simulink library "Centralized_I_Lib_Controller"  (R2024b)
settings: Solver=VariableStepAuto  StartTime=0.0  StopTime=10.0  RelTol=1e-3
(part 2 of 7)

== matlab function Centralized_I_Lib_Controller/computedTorqueControl_sym ==
  data: ddqd input; dqd input; qd input; kd input; kp input; tau output; dq input; q input
function tau = computedTorqueControl_sym(ddqd,dqd,qd,kd,kp,dq,q)
%#codegen

% Manually assign inputs from vectors to scalars
q1 = q(1);  q2 = q(2);  q3 = q(3);
q4 = q(4);  q5 = q(5);  q6 = q(6);

dq1 = dq(1);  dq2 = dq(2);  dq3 = dq(3);
dq4 = dq(4);  dq5 = dq(5);  dq6 = dq(6);

qd1 = qd(1);  qd2 = qd(2);  qd3 = qd(3);
qd4 = qd(4);  qd5 = qd(5);  qd6 = qd(6);

dqd1 = dqd(1);  dqd2 = dqd(2);  dqd3 = dqd(3);
dqd4 = dqd(4);  dqd5 = dqd(5);  dqd6 = dqd(6);

ddqd1 = ddqd(1);  ddqd2 = ddqd(2);  ddqd3 = ddqd(3);
ddqd4 = ddqd(4);  ddqd5 = ddqd(5);  ddqd6 = ddqd(6);

kp1 = kp(1); kp2 = kp(2); kp3 = kp(3);
kp4 = kp(4); kp5 = kp(5); kp6 = kp(6);

kd1 = kd(1); kd2 = kd(2); kd3 = kd(3);
kd4 = kd(4); kd5 = kd(5); kd6 = kd(6);

% Kp = diag(kp);
% Kd = diag(kd);

%    This function was generated by the Symbolic Math Toolbox version 24.2.
%    13-Jun-2025 15:28:52

% ddqd1 = complex(ddqd1);  % if required to enforce complex operations
% ddqd2 = complex(ddqd2);  % if required to enforce complex operations
% ddqd3 = complex(ddqd3);  % if required to enforce complex operations
% ddqd4 = complex(ddqd4);  % if required to enforce complex operations
% ddqd5 = complex(ddqd5);  % if required to enforce complex operations
% ddqd6 = complex(ddqd6);  % if required to enforce complex operations
% dq1 = complex(dq1);  % if required to enforce complex operations
% dq2 = complex(dq2);  % if required to enforce complex operations
% dq3 = complex(dq3);  % if required to enforce complex operations
% dq4 = complex(dq4);  % if required to enforce complex operations
% dq5 = complex(dq5);  % if required to enforce complex operations
% dq6 = complex(dq6);  % if required to enforce complex operations
% dqd1 = complex(dqd1);  % if required to enforce complex operations
% dqd2 = complex(dqd2);  % if required to enforce complex operations
% dqd3 = complex(dqd3);  % if required to enforce complex operations
% dqd4 = complex(dqd4);  % if required to enforce complex operations
% dqd5 = complex(dqd5);  % if required to enforce complex operations
% dqd6 = complex(dqd6);  % if required to enforce complex operations
% kd1 = complex(kd1);  % if required to enforce complex operations
% kd2 = complex(kd2);  % if required to enforce complex operations
% kd3 = complex(kd3);  % if required to enforce complex operations
% kd4 = complex(kd4);  % if required to enforce complex operations
% kd5 = complex(kd5);  % if required to enforce complex operations
% kd6 = complex(kd6);  % if required to enforce complex operations
% kp1 = complex(kp1);  % if required to enforce complex operations
% kp2 = complex(kp2);  % if required to enforce complex operations
% kp3 = complex(kp3);  % if required to enforce complex operations
% kp4 = complex(kp4);  % if required to enforce complex operations
% kp5 = complex(kp5);  % if required to enforce complex operations
% kp6 = complex(kp6);  % if required to enforce complex operations
% q1 = complex(q1);  % if required to enforce complex operations
% q2 = complex(q2);  % if required to enforce complex operations
% q3 = complex(q3);  % if required to enforce complex operations
% q4 = complex(q4);  % if required to enforce complex operations
% q5 = complex(q5);  % if required to enforce complex operations
% q6 = complex(q6);  % if required to enforce complex operations
% qd1 = complex(qd1);  % if required to enforce complex operations
% qd2 = complex(qd2);  % if required to enforce complex operations
% qd3 = complex(qd3);  % if required to enforce complex operations
% qd4 = complex(qd4);  % if required to enforce complex operations
% qd5 = complex(qd5);  % if required to enforce complex operations
% qd6 = complex(qd6);  % if required to enforce complex operations
t2 = cos(q1);
t3 = cos(q2);
t4 = cos(q3);
t5 = cos(q4);
t6 = cos(q5);
t7 = cos(q6);
t8 = sin(q1);
t9 = sin(q2);
t10 = sin(q3);
t11 = sin(q4);
t12 = sin(q5);
t13 = sin(q6);
t14 = q4.*2.0;
t15 = q5.*2.0;
t30 = -ddqd1;
t31 = -ddqd2;
t32 = -ddqd3;
t33 = -ddqd4;
t34 = -ddqd5;
t35 = -ddqd6;
t36 = -dqd1;
t37 = -dqd2;
t38 = -dqd3;
t39 = -dqd4;
t40 = -dqd5;
t41 = -dqd6;
t42 = -qd1;
t43 = -qd2;
t44 = -qd3;
t45 = -qd4;
t46 = -qd5;
t47 = -qd6;
t63 = sqrt(2.0);
t64 = pi./2.0;
t16 = cos(t14);
t17 = cos(t15);
t18 = t3.^2;
t19 = t4.^2;
t20 = t5.^2;
t21 = t6.^2;
t22 = t7.^2;
t23 = sin(t14);
t24 = sin(t15);
t25 = t9.^2;
t26 = t10.^2;
t27 = t11.^2;
t28 = t12.^2;
t29 = t13.^2;
t48 = t2.*t4;
t49 = t3.*t5;
t50 = t4.*t5;
t51 = t4.*t6;
t52 = t2.*t10;
t53 = t4.*t8;
t54 = t3.*t11;
t55 = t5.*t9;
t56 = t4.*t11;
t57 = t4.*t12;
t58 = t6.*t10;
t59 = t8.*t10;
t60 = t9.*t11;
t61 = t10.*t11;
t62 = t10.*t12;
t67 = t5.*t10.*4.0;
t68 = dq1+t36;
t69 = dq2+t37;
t70 = dq3+t38;
t71 = dq4+t39;
t72 = dq5+t40;
t73 = dq6+t41;
t74 = q1+t42;
t75 = q2+t43;
t76 = q3+t44;
t77 = q4+t45;
t78 = q5+t46;
t79 = q6+t47;
t80 = -t64;
t90 = t3.*(3.0./1.0e+1);
t91 = t6.*(3.0./4.0e+1);
t92 = t6.*(3.0./5.0e+1);
t93 = t9.*(3.0./1.0e+1);
t94 = t63+2.0;
t139 = t3.*(9.0./1.0e+1);
t141 = t6.*(3.0./2.0e+2);
t142 = t9.*(9.0./1.0e+1);
t143 = t12.*(3.0./1.0e+2);
t157 = -t63;
t158 = t63.*4.7e+1;
t175 = t5.*t12.*(3.0./4.0e+1);
t182 = t11.*t12.*(3.0./4.0e+1);
t184 = t4.*(3.9e+1./2.0e+2);
t185 = t5.*(9.0./4.0e+2);
t187 = t11.*(2.7e+1./1.0e+2);
t188 = t10.*(9.0./2.0e+2);
t229 = t3.*t6.*(3.0./1.0e+2);
t246 = t6.*t11.*(-3.0./4.0e+1);
t248 = t5.*t10.*(9.0./5.0e+1);
t249 = t3.*t12.*(3.0./2.0e+2);
t253 = t5.*t12.*(3.0./2.0e+2);
t257 = t5.*t10.*(3.0./4.0e+2);
t263 = t11.*t12.*(3.0./2.0e+2);
t266 = t5.*(1.17e+2./2.0e+2);
t309 = t5.*t6.*(-3.0./2.0e+2);
t310 = t3.*t4.*(9.0./2.0e+2);
t312 = t5.*t6.*(9.0./2.0e+2);
t331 = t5.*t12.*(9.0./1.0e+2);
t332 = t6.*t11.*(9.0./1.0e+2);
t335 = t6.*t9.*(-3.0./2.0e+2);
t338 = t6.*t11.*(-3.0./2.0e+2);
t340 = t4.*t9.*(9.0./2.0e+2);
t343 = t3.*t10.*(3.9e+1./2.0e+2);
t347 = t9.*t12.*(-3.0./1.0e+2);
t351 = t11.*t12.*(9.0./2.0e+2);
t352 = t9.*t10.*(3.9e+1./2.0e+2);
t436 = t5.*t6.*t11.*(6.0./2.5e+1);
t494 = t5.*t11.*t12.*(3.0./2.5e+1);
t519 = t6.*5.9765625e-3;
t520 = t2.*1.0675e-2;
t521 = t8.*1.0675e-2;
t522 = t12.*2.98828125e-3;
t595 = t3.*t6.*t9.*(-3.0./5.0e+1);
t663 = t4.*2.444921875e-1;
t664 = t5.*1.048828125e-2;
t667 = t11.*2.09765625e-2;
t933 = t5.*t11.*t12.*(-3.0./1.0e+2);
t955 = t5.*t6.*2.98828125e-3;
t957 = t7.*t13.*5.5078125e-3;
t959 = t5.*t12.*5.9765625e-3;
t1077 = t5.*t6.*t11.*t12.*(-3.0./5.0e+1);
t1132 = t5.*t6.*t11.*(-9.0./2.0e+2);
t1137 = t5.*t6.*t12.*2.05078125e-2;
t1191 = t11.*t12.*(-2.98828125e-3);
t1323 = t63.*2.75390625e-3;
t1418 = t5.*t11.*6.88175e-1;
t1598 = t2.*t6.*t12.*1.865e-2;
t1599 = t3.*t4.*t10.*9.325e-3;
t1618 = t6.*t8.*t12.*1.865e-2;
t1625 = t4.*t9.*t10.*9.325e-3;
t1702 = t4.*5.198296875e-1;
t1803 = t7.*t9.*t13.*(-5.5078125e-3);
t1804 = t7.*t10.*t13.*(-5.5078125e-3);
t1805 = t7.*t11.*t13.*(-5.5078125e-3);
t1806 = t7.*t12.*t13.*(-5.5078125e-3);
t1831 = t3.*t4.*1.039659375;
t1845 = t3.*t9.*1.4703625;
t1846 = t6.*t12.*2.98328125e-2;
t1917 = t3.*t63.*1.376953125e-3;
t1918 = t5.*t63.*1.376953125e-3;
t1925 = t9.*t63.*(-2.75390625e-3);
t1926 = t11.*t63.*(-2.75390625e-3);
t1927 = t12.*t63.*1.376953125e-3;
t2024 = t3.*t10.*5.198296875e-1;
t2061 = t3.*t9.*t63.*5.5078125e-3;
t2062 = t5.*t11.*t63.*5.5078125e-3;
t2091 = t3.*t4.*t7.*t13.*(-5.5078125e-3);
t2213 = t6.*t7.*t63.*(-2.75390625e-3);
t2222 = t7.*t13.*t63.*(-2.75390625e-3);
t2250 = t5.*t6.*t7.*t11.*t13.*1.1015625e-2;
t2362 = t6.*t7.*t12.*t63.*5.5078125e-3;
t2423 = t5.*t10.*t63.*(-1.376953125e-3);
t2425 = t11.*t12.*t63.*(-1.376953125e-3);
t2571 = t5.*t6.*t13.*t63.*(-2.75390625e-3);
t3047 = t5.*t6.*t7.*t12.*t63.*(-5.5078125e-3);
t3690 = t3.*t6.*t7.*t9.*t12.*t63.*(-5.5078125e-3);
t6734 = t3.*1.181403645833333e-1;
t6735 = t9.*2.362807291666667e-1;
t6736 = t4.*t10.*1.180036458333333e-1;
t6754 = t3.*t4.*t10.*(-1.180036458333333e-1);
t65 = t50.*4.0;
t66 = t56.*4.0;
t82 = t9.*t59;
t83 = t8.*t60;
t84 = t11.*t59;
t85 = t10.*t60;
t86 = t12.*t60;
t87 = t12.*t61;
t88 = -t58;
t89 = -t61;
t95 = t2.*t49;
t96 = t5.*t48;
t97 = t3.*t51;
t98 = t6.*t49;
t99 = t6.*t50;
t100 = t9.*t48;
t101 = t2.*t54;
t102 = t2.*t55;
t103 = t8.*t49;
t104 = t11.*t48;
t105 = t5.*t52;
t106 = t8.*t50;
t107 = t10.*t49;
t108 = t3.*t57;
t109 = t3.*t58;
t110 = t9.*t51;
t111 = t12.*t49;
t112 = t6.*t55;
t113 = t12.*t50;
t114 = t11.*t51;
t115 = t9.*t52;
t116 = t9.*t53;
t117 = t2.*t60;
t118 = t8.*t54;
t119 = t8.*t55;
t120 = t11.*t52;
t121 = t11.*t53;
t122 = t5.*t59;
t123 = t10.*t54;
t124 = t10.*t55;
t125 = t3.*t62;
t126 = t9.*t57;
t127 = t12.*t55;
t128 = t6.*t60;
t129 = t12.*t56;
t130 = t11.*t58;
t131 = t49.*(2.0./5.0);
t132 = t49.*(6.0./5.0);
t133 = t54.*(2.0./5.0);
t134 = t55.*(2.0./5.0);
t135 = t54.*(6.0./5.0);
t136 = t55.*(6.0./5.0);
t137 = t60.*(2.0./5.0);
t138 = t60.*(6.0./5.0);
t140 = -t91;
t144 = kd1.*t68;
t145 = kd2.*t69;
t146 = kd3.*t70;
t147 = kd4.*t71;
t148 = kd5.*t72;
t149 = kd6.*t73;
t150 = kp1.*t74;
t151 = kp2.*t75;
t152 = kp3.*t76;
t153 = kp4.*t77;
t154 = kp5.*t78;
t155 = kp6.*t79;
t156 = q6+t80;
t159 = t2.*t90;
t160 = t49./1.0e+1;
t161 = t49.*(3.0./1.0e+1);
t162 = t51.*(3.0./2.5e+1);
t163 = t5.*t91;
t164 = t51.*(3.0./5.0e+1);
t167 = t2.*t93;
t168 = t8.*t90;
t169 = t54./1.0e+1;
t171 = t55./1.0e+1;
t172 = t54.*(3.0./1.0e+1);
t173 = t55.*(3.0./1.0e+1);
t174 = t58.*(3.0./4.0e+1);
t177 = t9.*t92;
t178 = t57.*(3.0./5.0e+1);
t179 = t8.*t93;
t180 = t60./1.0e+1;
t181 = t60.*(3.0./1.0e+1);
t183 = -t141;
t186 = -t143;
t189 = t3.*t6.*t48;
t190 = t49.*t52;
t191 = t48.*t55;
t192 = t3.*t12.*t48;
t194 = t51.*t54;
t195 = t49.*t58;
t196 = t52.*t54;
t197 = t48.*t60;
t198 = t52.*t55;
t199 = t49.*t59;
t201 = t3.*t12.*t53;
t202 = t54.*t57;
t203 = t49.*t62;
t204 = t54.*t58;
t206 = t52.*t60;
t207 = t54.*t59;
t208 = t53.*t60;
t209 = t55.*t59;
t210 = t54.*t62;
t211 = t58.*t60;
t214 = t59.*t60;
t215 = t60.*t62;
t227 = t2.*t139;
t228 = t50.*(9.0./4.0e+1);
t230 = t51.*(3.0./1.0e+2);
t231 = t51.*(3.0./2.0e+2);
t233 = t49.*(3.0./4.0e+2);
t242 = t2.*t142;
t243 = t8.*t139;
t245 = -t175;
t250 = t9.*t141;
t251 = t57.*(3.0./2.0e+2);
t252 = t58.*(3.0./2.0e+2);
t254 = t11.*t141;
t255 = t54.*(3.0./4.0e+2);
t256 = t55.*(3.0./4.0e+2);
t258 = t157+2.0;
t259 = t8.*t142;
t260 = t9.*t143;
t261 = t62.*(3.0./1.0e+2);
t262 = t61.*(3.0./2.0e+2);
t264 = t60.*(3.0./4.0e+2);
t265 = t61.*(3.0./4.0e+2);
t267 = t17.*(3.0./1.0e+2);
t268 = t24.*(3.0./1.0e+2);
t282 = t9.*t50.*(2.0./5.0);
t291 = t9.*t50.*(6.0./5.0);
t308 = -t229;
t311 = t51.*(9.0./2.0e+2);
t313 = t3.*t184;
t318 = (t12.*t59)./1.0e+1;
t321 = (t9.*t62)./1.0e+1;
t322 = t12.*t59.*(3.0./1.0e+1);
t325 = t62.*t93;
t333 = t56.*(2.7e+1./1.0e+2);
t334 = -t249;
t339 = t3.*t188;
t341 = t57.*(9.0./2.0e+2);
t342 = t58.*(9.0./2.0e+2);
t344 = t9.*t184;
t345 = -t257;
t346 = sqrt(t94);
t348 = t62.*(9.0./1.0e+2);
t349 = t9.*t188;
t350 = t62.*(9.0./2.0e+2);
t355 = -t266;
t356 = t6.*t20.*(3.0./2.5e+1);
t357 = t20.*t92;
t358 = t6.*t27.*(3.0./2.5e+1);
t359 = t16.*(3.9e+1./2.0e+2);
t361 = t23.*(3.9e+1./2.0e+2);
t371 = t4.*t49.*(-2.0./5.0);
t377 = (t6.*t48)./1.0e+1;
t381 = t6.*t48.*(3.0./1.0e+1);
t384 = t51.*t90;
t389 = t49.*t92;
t390 = t50.*t92;
t406 = (t12.*t48)./1.0e+1;
t408 = (t6.*t52)./1.0e+1;
t413 = (t8.*t51)./1.0e+1;
t420 = t12.*t48.*(3.0./1.0e+1);
t421 = t6.*t52.*(3.0./1.0e+1);
t425 = t8.*t51.*(3.0./1.0e+1);
t427 = t57.*t90;
t429 = t51.*t93;
t443 = t5.*t58.*(3.0./5.0e+1);
t444 = t5.*t11.*t92;
t460 = (t12.*t52)./1.0e+1;
t463 = (t12.*t53)./1.0e+1;
t464 = (t9.*t56)./1.0e+1;
t468 = (t8.*t58)./1.0e+1;
t474 = (t9.*t58)./1.0e+1;
t475 = t12.*t52.*(3.0./1.0e+1);
t478 = t12.*t53.*(3.0./1.0e+1);
t479 = t56.*t93;
t482 = t8.*t58.*(3.0./1.0e+1);
t484 = t62.*t90;
t486 = t58.*t93;
t490 = t9.*t58.*(3.0./2.5e+1);
t491 = t12.*t54.*(3.0./2.5e+1);
t493 = t5.*t62.*(3.0./2.5e+1);
t499 = t60.*t92;
t500 = t5.*t62.*(3.0./5.0e+1);
t502 = -t310;
t503 = t50.*(1.17e+2./2.0e+2);
t514 = -t340;
t517 = t56.*(8.1e+1./2.0e+2);
t518 = -t351;
t524 = t6.*t20.*(-3.0./5.0e+1);
t525 = t18.*t141;
t526 = t19.*t141;
t527 = t20.*t141;
t528 = t18.*t143;
t529 = t19.*t143;
t530 = t10.*t21.*(3.0./1.0e+2);
t531 = t20.*t143;
t532 = t11.*t19.*(3.0./4.0e+2);
t533 = t10.*t28.*(3.0./1.0e+2);
t534 = t11.*t26.*(3.0./4.0e+2);
t585 = t6.*t54.*(-1.0./1.0e+1);
t592 = t6.*t54.*(-3.0./1.0e+1);
t594 = -t436;
t597 = t10.*t51.*(-3.0./5.0e+1);
t598 = t9.*t49.*(2.7e+1./5.0e+1);
t603 = t51.*t143;
t614 = t9.*t50.*(3.0./4.0e+2);
t615 = t10.*t50.*(3.0./4.0e+2);
t636 = -t494;
t643 = t10.*t57.*(3.0./1.0e+2);
t649 = t12.*t54.*(3.0./2.0e+2);
t652 = t5.*t62.*(3.0./2.0e+2);
t665 = t20.*t51.*(6.0./2.5e+1);
t666 = t21.*t49.*(3.0./5.0e+1);
t668 = t18.*t58.*(3.0./2.5e+1);
t670 = t20.*t57.*(3.0./2.5e+1);
t671 = t5.*t12.*t19.*(3.0./2.5e+1);
t672 = t21.*t54.*(3.0./5.0e+1);
t673 = t21.*t55.*(3.0./5.0e+1);
t675 = t5.*t10.*t21.*(3.0./5.0e+1);
t677 = t25.*t58.*(3.0./2.5e+1);
t679 = t5.*t12.*t26.*(3.0./2.5e+1);
t680 = t21.*t60.*(3.0./5.0e+1);
t681 = t21.*t61.*(3.0./5.0e+1);
t682 = t4.*t20.*(3.9e+1./1.0e+2);
t683 = t6.*t18.*(-3.0./2.0e+2);
t684 = t6.*t19.*(-3.0./2.0e+2);
t685 = t6.*t20.*(-3.0./2.0e+2);
t686 = t4.*t18.*(9.0./2.0e+2);
t691 = t12.*t18.*(-3.0./1.0e+2);
t692 = t12.*t19.*(-3.0./1.0e+2);
t693 = t12.*t20.*(-3.0./1.0e+2);
t695 = t4.*t25.*(9.0./2.0e+2);
t696 = t12.*t20.*(9.0./2.0e+2);
t697 = t10.*t18.*(3.9e+1./2.0e+2);
t698 = t9.*t20.*(3.9e+1./2.0e+2);
t701 = t12.*t27.*(9.0./2.0e+2);
t702 = t10.*t25.*(3.9e+1./2.0e+2);
t703 = t9.*t27.*(3.9e+1./2.0e+2);
t704 = t48.*t49.*(-2.0./5.0);
t705 = t48.*t49.*(-6.0./5.0);
t708 = t6.*t48.*t90;
t715 = t49.*t53.*(-2.0./5.0);
t720 = t49.*t53.*(-6.0./5.0);
t731 = t12.*t48.*t90;
t732 = t6.*t52.*t90;
t734 = t6.*t48.*t93;
t753 = t49.*t57.*(3.0./2.5e+1);
t755 = t50.*t58.*(3.0./2.5e+1);
t762 = t19.*t21.*(3.0./5.0e+1);
t789 = t12.*t52.*t90;
t790 = t12.*t48.*t93;
t793 = t6.*t52.*t93;
t795 = t12.*t53.*t90;
t828 = t11.*t55.*t92;
t829 = t12.*t54.*t92;
t834 = t19.*t28.*(3.0./5.0e+1);
t835 = t4.*t49.*(2.7e+1./1.0e+2);
t861 = t12.*t52.*t93;
t863 = t12.*t59.*t90;
t864 = t12.*t53.*t93;
t887 = t55.*t62.*(3.0./2.5e+1);
t888 = t56.*t62.*(3.0./2.5e+1);
t894 = t12.*t51.*(-3.0./1.0e+2);
t897 = t4.*t54.*(2.7e+1./1.0e+2);
t899 = t9.*t50.*(2.7e+1./1.0e+2);
t900 = t11.*t50.*(3.9e+1./1.0e+2);
t902 = t6.*t54.*(-3.0./2.0e+2);
t905 = t5.*t58.*(-3.0./2.0e+2);
t909 = t6.*t54.*(9.0./2.0e+2);
t913 = t11.*t312;
t915 = t11.*t49.*(3.9e+1./2.0e+2);
t916 = t4.*t54.*(-3.0./4.0e+2);
t931 = t12.*t54.*(-3.0./1.0e+2);
t936 = t11.*t331;
t939 = t11.*t55.*(3.9e+1./1.0e+2);
t954 = t51.*2.98828125e-3;
t956 = t9.*t62.*(-9.0./2.0e+2);
t958 = t58.*5.9765625e-3;
t960 = t54.*1.0675e-2;
t961 = t55.*1.0675e-2;
t962 = t60.*1.0675e-2;
t963 = t62.*2.98828125e-3;
t964 = t11.*t522;
t966 = t3.*t4.*t21.*(3.0./1.0e+2);
t967 = t19.*t229;
t968 = t20.*t229;
t971 = t18.*t50.*(3.0./4.0e+2);
t973 = t6.*t9.*t20.*(-3.0./2.5e+1);
t979 = t3.*t4.*t28.*(3.0./1.0e+2);
t982 = t19.*t54.*(3.0./2.0e+2);
t983 = t19.*t249;
t984 = t20.*t249;
t988 = t25.*t50.*(3.0./4.0e+2);
t992 = t21.*t61.*(3.0./1.0e+2);
t993 = t26.*t249;
t997 = t18.*t266;
t998 = t4.*t21.*1.025390625e-2;
t999 = t5.*t21.*1.025390625e-2;
t1001 = t11.*t18.*(-2.7e+1./1.0e+2);
t1005 = t5.*t28.*1.025390625e-2;
t1009 = t22.*5.5078125e-3;
t1018 = t49.*t57.*(-1.0./1.0e+1);
t1022 = t49.*t57.*(-3.0./1.0e+1);
t1031 = t49.*t57.*(3.0./1.0e+2);
t1040 = t18.*t21.*(3.0./1.0e+2);
t1041 = t20.*t21.*(3.0./1.0e+2);
t1073 = t6.*t12.*t54.*(-3.0./5.0e+1);
t1076 = t5.*t12.*t58.*(-3.0./5.0e+1);
t1078 = t49.*t60.*(3.9e+1./5.0e+1);
t1095 = t18.*t28.*(3.0./1.0e+2);
t1096 = t20.*t28.*(3.0./1.0e+2);
t1098 = t4.*t49.*(1.17e+2./2.0e+2);
t1110 = t55.*t62.*(-1.0./1.0e+1);
t1114 = t55.*t62.*(-3.0./1.0e+1);
t1123 = t55.*t62.*(3.0./2.0e+2);
t1125 = t56.*t62.*(3.0./2.0e+2);
t1131 = t5.*t58.*(-9.0./2.0e+2);
t1134 = t4.*t54.*(1.17e+2./2.0e+2);
t1158 = t9.*t54.*(1.17e+2./1.0e+2);
t1160 = t9.*t56.*(1.17e+2./2.0e+2);
t1162 = t12.*t58.*2.05078125e-2;
t1163 = t50.*2.09765625e-2;
t1169 = -t957;
t1170 = t54.*1.048828125e-2;
tau = ft_1({dq1,dq2,dq3,dq4,dq5,dq6,t10,t100,t1001,t1005,t1009,t101,t1018,t102,t1022,t103,t1031,t104,t1040,t1041,t105,t106,t107,t1073,t1076,t1077,t1078,t108,t109,t1095,t1096,t1098,t11,t110,t111,t1110,t1114,t112,t1123,t1125,t113,t1131,t1132,t1134,t1137,t114,t115,t1158,t116,t1160,t1162,t1163,t1169,t117,t1170,t118,t119,t1191,t12,t120,t121,t122,t123,t124,t125,t126,t127,t128,t129,t13,t130,t131,t132,t1323,t133,t134,t135,t136,t137,t138,t139,t140,t141,t1418,t142,t143,t144,t145,t146,t147,t148,t149,t150,t151,t152,t153,t154,t155,t156,t158,t159,t1598,t1599,t160,t161,t1618,t162,t1625,t163,t164,t167,t168,t169,t1702,t171,t172,t173,t174,t177,t178,t179,t18,t180,t1803,t1804,t1805,t1806,t181,t182,t183,t1831,t184,t1845,t1846,t185,t186,t187,t188,t189,t19,t190,t191,t1917,t1918,t192,t1925,t1926,t1927,t194,t195,t196,t197,t198,t199,t2,t20,t201,t202,t2024,t203,t204,t206,t2061,t2062,t207,t208,t209,t2091,t21,t210,t211,t214,t215,t22,t2213,t2222,t2250,t227,t228,t229,t230,t231,t233,t2362,t242,t2423,t2425,t243,t245,t246,t248,t249,t25,t250,t251,t252,t253,t254,t255,t256,t2571,t258,t259,t26,t260,t261,t262,t263,t264,t265,t267,t268,t27,t28,t282,t29,t291,t3,t30,t3047,t308,t309,t31,t311,t312,t313,t318,t32,t321,t322,t325,t33,t331,t332,t333,t334,t335,t338,t339,t34,t341,t342,t343,t344,t345,t346,t347,t348,t349,t35,t350,t351,t352,t355,t356,t357,t358,t359,t361,t3690,t371,t377,t381,t384,t389,t390,t4,t406,t408,t413,t420,t421,t425,t427,t429,t436,t443,t444,t460,t463,t464,t468,t474,t475,t478,t479,t48,t482,t484,t486,t49,t490,t491,t493,t494,t499,t5,t50,t500,t502,t503,t51,t514,t517,t518,t519,t52,t520,t521,t522,t524,t525,t526,t527,t528,t529,t53,t530,t531,t532,t533,t534,t54,t55,t56,t57,t58,t585,t59,t592,t594,t595,t597,t598,t6,t60,t603,t61,t614,t615,t62,t63,t636,t643,t649,t65,t652,t66,t663,t664,t665,t666,t667,t668,t67,t670,t671,t672,t673,t6734,t6735,t6736,t675,t6754,t677,t679,t680,t681,t682,t683,t684,t685,t686,t691,t692,t693,t695,t696,t697,t698,t7,t701,t702,t703,t704,t705,t708,t715,t720,t731,t732,t734,t753,t755,t762,t789,t790,t793,t795,t8,t82,t828,t829,t83,t834,t835,t84,t85,t86,t861,t863,t864,t87,t88,t887,t888,t89,t894,t897,t899,t9,t90,t900,t902,t905,t909,t913,t915,t916,t92,t93,t931,t933,t936,t939,t95,t954,t955,t956,t957,t958,t959,t96,t960,t961,t962,t963,t964,t966,t967,t968,t97,t971,t973,t979,t98,t982,t983,t984,t988,t99,t992,t993,t997,t998,t999});
end
function tau = ft_1(ct)
[dq1,dq2,dq3,dq4,dq5,dq6,t10,t100,t1001,t1005,t1009,t101,t1018,t102,t1022,t103,t1031,t104,t1040,t1041,t105,t106,t107,t1073,t1076,t1077,t1078,t108,t109,t1095,t1096,t1098,t11,t110,t111,t1110,t1114,t112,t1123,t1125,t113,t1131,t1132,t1134,t1137,t114,t115,t1158,t116,t1160,t1162,t1163,t1169,t117,t1170,t118,t119,t1191,t12,t120,t121,t122,t123,t124,t125,t126,t127,t128,t129,t13,t130,t131,t132,t1323,t133,t134,t135,t136,t137,t138,t139,t140,t141,t1418,t142,t143,t144,t145,t146,t147,t148,t149,t150,t151,t152,t153,t154,t155,t156,t158,t159,t1598,t1599,t160,t161,t1618,t162,t1625,t163,t164,t167,t168,t169,t1702,t171,t172,t173,t174,t177,t178,t179,t18,t180,t1803,t1804,t1805,t1806,t181,t182,t183,t1831,t184,t1845,t1846,t185,t186,t187,t188,t189,t19,t190,t191,t1917,t1918,t192,t1925,t1926,t1927,t194,t195,t196,t197,t198,t199,t2,t20,t201,t202,t2024,t203,t204,t206,t2061,t2062,t207,t208,t209,t2091,t21,t210,t211,t214,t215,t22,t2213,t2222,t2250,t227,t228,t229,t230,t231,t233,t2362,t242,t2423,t2425,t243,t245,t246,t248,t249,t25,t250,t251,t252,t253,t254,t255,t256,t2571,t258,t259,t26,t260,t261,t262,t263,t264,t265,t267,t268,t27,t28,t282,t29,t291,t3,t30,t3047,t308,t309,t31,t311,t312,t313,t318,t32,t321,t322,t325,t33,t331,t332,t333,t334,t335,t338,t339,t34,t341,t342,t343,t344,t345,t346,t347,t348,t349,t35,t350,t351,t352,t355,t356,t357,t358,t359,t361,t3690,t371,t377,t381,t384,t389,t390,t4,t406,t408,t413,t420,t421,t425,t427,t429,t436,t443,t444,t460,t463,t464,t468,t474,t475,t478,t479,t48,t482,t484,t486,t49,t490,t491,t493,t494,t499,t5,t50,t500,t502,t503,t51,t514,t517,t518,t519,t52,t520,t521,t522,t524,t525,t526,t527,t528,t529,t53,t530,t531,t532,t533,t534,t54,t55,t56,t57,t58,t585,t59,t592,t594,t595,t597,t598,t6,t60,t603,t61,t614,t615,t62,t63,t636,t643,t649,t65,t652,t66,t663,t664,t665,t666,t667,t668,t67,t670,t671,t672,t673,t6734,t6735,t6736,t675,t6754,t677,t679,t680,t681,t682,t683,t684,t685,t686,t691,t692,t693,t695,t696,t697,t698,t7,t701,t702,t703,t704,t705,t708,t715,t720,t731,t732,t734,t753,t755,t762,t789,t790,t793,t795,t8,t82,t828,t829,t83,t834,t835,t84,t85,t86,t861,t863,t864,t87,t88,t887,t888,t89,t894,t897,t899,t9,t90,t900,t902,t905,t909,t913,t915,t916,t92,t93,t931,t933,t936,t939,t95,t954,t955,t956,t957,t958,t959,t96,t960,t961,t962,t963,t964,t966,t967,t968,t97,t971,t973,t979,t98,t982,t983,t984,t988,t99,t992,t993,t997,t998,t999] = ct{:};
t1171 = t55.*1.048828125e-2;
t1172 = t56.*1.048828125e-2;
t1173 = t10.*t664;
t1175 = t5.*t6.*t11.*t18.*(3.0./2.5e+1);
t1180 = t3.*t4.*t10.*t21.*(3.0./5.0e+1);
t1184 = t9.*t21.*t50.*(3.0./5.0e+1);
t1186 = t10.*t21.*t50.*(3.0./5.0e+1);
t1189 = t60.*2.09765625e-2;
t1196 = t19.*t494;
t1197 = t9.*t20.*t58.*(6.0./2.5e+1);
t1198 = t5.*t11.*t12.*t18.*(6.0./2.5e+1);
t1199 = t3.*t4.*t10.*t28.*(3.0./5.0e+1);
t1200 = t3.*t9.*t12.*t20.*(3.0./5.0e+1);
t1201 = t12.*t19.*t54.*(3.0./5.0e+1);
t1204 = t3.*t12.*t26.*t92;
t1205 = t5.*t11.*t12.*t18.*(3.0./5.0e+1);
t1207 = t3.*t6.*t20.*(-3.0./1.0e+2);
t1208 = t20.*t51.*(-3.0./1.0e+2);
t1211 = t18.*t312;
t1214 = t19.*t49.*(-3.0./4.0e+2);
t1219 = t3.*t6.*t26.*(-3.0./1.0e+2);
t1220 = t27.*t51.*(-3.0./1.0e+2);
t1221 = t18.*t57.*(9.0./1.0e+2);
t1222 = t18.*t331;
t1223 = t18.*t332;
t1224 = t20.*t57.*(9.0./1.0e+2);
t1225 = t3.*t10.*t20.*(3.9e+1./1.0e+2);
t1228 = t3.*t12.*t19.*(-3.0./2.0e+2);
t1229 = t3.*t12.*t20.*(-3.0./2.0e+2);
t1230 = t20.*t335;
t1231 = t20.*t57.*(-3.0./2.0e+2);
t1233 = t26.*t312;
t1234 = t20.*t347;
t1236 = t25.*t57.*(9.0./1.0e+2);
t1237 = t18.*t61.*(2.7e+1./1.0e+2);
t1238 = t9.*t10.*t20.*(3.9e+1./1.0e+2);
t1239 = t27.*t57.*(-3.0./2.0e+2);
t1240 = t26.*t338;
t1242 = t18.*t351;
t1246 = t11.*t12.*t26.*(-3.0./1.0e+2);
t1247 = t25.*t61.*(2.7e+1./1.0e+2);
t1266 = t6.*t18.*t20.*(6.0./2.5e+1);
t1294 = t6.*t18.*t27.*(6.0./2.5e+1);
t1295 = t12.*t18.*t20.*(3.0./5.0e+1);
t1297 = t49.*t51.*(9.0./1.0e+2);
t1298 = t49.*t51.*(-3.0./2.0e+2);
t1322 = t11.*t21.*t26.*(3.0./5.0e+1);
t1347 = t18.*t20.*(3.9e+1./1.0e+2);
t1348 = t19.*t20.*(3.9e+1./2.0e+2);
t1357 = t51.*t60.*(9.0./1.0e+2);
t1361 = t49.*t61.*(3.9e+1./1.0e+2);
t1362 = t50.*t60.*(3.9e+1./1.0e+2);
t1363 = t50.*t61.*(3.9e+1./1.0e+2);
t1366 = t55.*t58.*(-3.0./2.0e+2);
t1384 = t18.*t27.*(3.9e+1./1.0e+2);
t1385 = t19.*t27.*(3.9e+1./2.0e+2);
t1397 = t9.*t50.*(-1.17e+2./2.0e+2);
t1398 = -t1137;
t1413 = t4.*t21.*t49.*(-3.0./5.0e+1);
t1427 = t3.*t6.*t12.*t19.*(-3.0./5.0e+1);
t1429 = t6.*t19.*t54.*(3.0./1.0e+2);
t1434 = t11.*t21.*t50.*(3.0./1.0e+2);
t1438 = t12.*t19.*t54.*(-3.0./2.5e+1);
t1450 = t11.*t28.*t50.*(3.0./1.0e+2);
t1456 = t3.*t4.*t20.*(-3.9e+1./1.0e+2);
t1457 = t20.*t51.*(-9.0./2.0e+2);
t1458 = t5.*t6.*t19.*(-9.0./2.0e+2);
t1462 = t6.*t11.*t18.*(-9.0./1.0e+2);
t1464 = t4.*t9.*t20.*(-3.9e+1./1.0e+2);
t1465 = t25.*t51.*(-9.0./2.0e+2);
t1467 = t21.*t56.*1.025390625e-2;
t1473 = t28.*t56.*1.025390625e-2;
t1474 = t2.*t19.*9.325e-3;
t1475 = t3.*t19.*9.325e-3;
t1476 = t2.*t21.*9.325e-3;
t1477 = t3.*t22.*2.75390625e-3;
t1478 = t4.*t22.*2.75390625e-3;
t1479 = t5.*t22.*2.75390625e-3;
t1480 = t25.*t62.*(-9.0./2.0e+2);
t1481 = t9.*t12.*t27.*(-9.0./2.0e+2);
t1485 = t8.*t19.*9.325e-3;
t1486 = t3.*t26.*9.325e-3;
t1487 = t8.*t21.*9.325e-3;
t1488 = t12.*t22.*2.75390625e-3;
t1489 = t12.*t29.*2.75390625e-3;
t1490 = t20.*6.88175e-1;
t1493 = t6.*t19.*t20.*(-3.0./2.5e+1);
t1494 = t6.*t18.*t20.*(3.0./1.0e+2);
t1497 = t12.*t48.*t54.*(-1.0./1.0e+1);
t1502 = t12.*t48.*t54.*(-3.0./1.0e+1);
t1528 = t49.*t51.*(-9.0./2.0e+2);
t1532 = t12.*t53.*t54.*(-1.0./1.0e+1);
t1538 = t12.*t53.*t54.*(-3.0./1.0e+1);
t1557 = -t1323;
t1558 = t49.*t57.*(-9.0./2.0e+2);
t1581 = t51.*t60.*(-9.0./2.0e+2);
t1582 = t55.*t58.*(-9.0./2.0e+2);
t1597 = t10.*t48.*1.865e-2;
t1617 = t10.*t53.*1.865e-2;
t1619 = t9.*t957;
t1620 = t10.*t957;
t1621 = t11.*t957;
t1622 = t12.*t957;
t1638 = t3.*t6.*t9.*t12.*t19.*(3.0./2.5e+1);
t1643 = t6.*t18.*t494;
t1651 = t18.*t20.*t28.*(3.0./5.0e+1);
t1660 = -t1418;
t1684 = t10.*t18.*t50.*(-3.0./4.0e+2);
t1685 = t3.*t19.*t347;
t1689 = t10.*t20.*t57.*(-3.0./1.0e+2);
t1696 = t12.*t19.*t54.*(-3.0./2.0e+2);
t1713 = t5.*t10.*t25.*(-1.17e+2./2.0e+2);
t1719 = t18.*t21.*t50.*(3.0./5.0e+1);
t1720 = t10.*t22.*(-5.5078125e-3);
t1726 = t49.*t51.*t61.*(6.0./2.5e+1);
t1730 = t19.*t21.*t54.*(3.0./2.5e+1);
t1732 = t18.*t20.*t58.*(6.0./2.5e+1);
t1733 = t21.*t25.*t50.*(3.0./5.0e+1);
t1740 = t20.*t25.*t58.*(6.0./2.5e+1);
t1741 = t6.*t1323;
t1747 = t9.*t1323;
t1748 = t11.*t1323;
t1756 = t9.*t20.*t21.*(-3.0./1.0e+2);
t1757 = t12.*t18.*t20.*(9.0./1.0e+2);
t1760 = t11.*t18.*t19.*(-3.0./4.0e+2);
t1772 = t9.*t20.*t28.*(-3.0./1.0e+2);
t1773 = t12.*t18.*t27.*(9.0./1.0e+2);
t1774 = t10.*t20.*t25.*(3.9e+1./1.0e+2);
t1776 = t4.*t9.*t49.*(-1.17e+2./2.0e+2);
t1785 = t4.*t49.*1.048828125e-2;
t1801 = t18.*t20.*t21.*(3.0./5.0e+1);
t1808 = -t1625;
t1822 = t20.*t51.*t62.*(-3.0./5.0e+1);
t1823 = t19.*t1077;
t1828 = t21.*t50.*t60.*(3.0./1.0e+2);
t1832 = t18.*t19.*t28.*(-3.0./5.0e+1);
t1839 = t28.*t49.*t61.*(3.0./1.0e+2);
t1840 = t28.*t50.*t60.*(3.0./1.0e+2);
t1849 = t6.*t19.*t54.*(-9.0./2.0e+2);
t1852 = t3.*t4.*t10.*t20.*(-3.9e+1./2.0e+2);
t1853 = t11.*t19.*t49.*(-3.9e+1./2.0e+2);
t1858 = t3.*t4.*t10.*t27.*(-3.9e+1./2.0e+2);
t1861 = t22.*t51.*2.75390625e-3;
t1866 = t18.*t957;
t1867 = t19.*t957;
t1869 = t20.*t957;
t1870 = t21.*t957;
t1872 = t4.*t9.*t20.*9.325e-3;
t1873 = t21.*t54.*9.325e-3;
t1876 = t22.*t54.*2.75390625e-3;
t1877 = t22.*t55.*2.75390625e-3;
t1878 = t22.*t56.*2.75390625e-3;
t1880 = t29.*t51.*2.75390625e-3;
t1881 = t5.*t6.*t29.*2.75390625e-3;
t1884 = t2.*t9.*t26.*9.325e-3;
t1886 = t4.*t9.*t27.*9.325e-3;
t1887 = t28.*t54.*9.325e-3;
t1888 = t22.*t62.*2.75390625e-3;
t1890 = t8.*t9.*t26.*9.325e-3;
t1891 = t29.*t62.*2.75390625e-3;
t1893 = t19.*t21.*t49.*(-3.0./5.0e+1);
t1897 = t49.*t51.*t61.*(-3.0./5.0e+1);
t1899 = t5.*t12.*t18.*t19.*(-3.0./2.5e+1);
t1919 = t21.*2.98328125e-2;
t1944 = t12.*t19.*t27.*(-9.0./2.0e+2);
t1947 = t50.*t957;
t1948 = t51.*t957;
t1949 = t5.*t6.*t957;
t1950 = t3.*t10.*t48.*9.325e-3;
t1951 = t49.*t56.*9.325e-3;
t1962 = t57.*t957;
t1963 = t58.*t957;
t1967 = t3.*t10.*t53.*9.325e-3;
t1968 = t50.*t60.*9.325e-3;
t1969 = t6.*t12.*t54.*9.325e-3;
t1978 = t60.*t957;
t1979 = t62.*t957;
t1983 = t55.*t61.*9.325e-3;
t1989 = t11.*t50.*6.88175e-1;
t1999 = t11.*t55.*6.88175e-1;
t2001 = t18.*t51.*t61.*(-3.0./1.0e+2);
t2002 = t21.*t49.*t61.*(-3.0./1.0e+2);
t2008 = t19.*t49.*t60.*(3.9e+1./1.0e+2);
t2014 = t19.*t20.*t28.*(-3.0./1.0e+2);
t2023 = -t1846;
t2025 = t9.*t1702;
t2030 = t3.*t4.*t22.*(-5.5078125e-3);
t2031 = t5.*t6.*t22.*(-2.75390625e-3);
t2034 = t3.*t9.*t22.*(-5.5078125e-3);
t2035 = t2.*t9.*t19.*(-9.325e-3);
t2036 = t3.*t10.*t22.*(-2.75390625e-3);
t2037 = t4.*t9.*t22.*(-2.75390625e-3);
t2046 = t8.*t9.*t19.*(-9.325e-3);
t2052 = t50.*t1323;
t2053 = t5.*t7.*t1323;
t2055 = t3.*t20.*3.440875e-1;
t2056 = t4.*t20.*3.440875e-1;
t2058 = t11.*t12.*t29.*(-2.75390625e-3);
t2063 = t4.*t10.*t1323;
t2064 = t58.*t1323;
t2065 = t5.*t12.*t1323;
t2066 = t5.*t13.*t1323;
t2070 = t7.*t12.*t1323;
t2071 = t7.*t13.*t1323;
t2072 = t4.*t27.*3.440875e-1;
t2076 = t60.*t1323;
t2078 = t12.*t13.*t1323;
t2085 = -t1917;
t2086 = -t1918;
t2092 = t7.*t13.*t51.*(-5.5078125e-3);
t2094 = t20.*t22.*(-5.5078125e-3);
t2096 = t7.*t13.*t58.*(-5.5078125e-3);
t2097 = t6.*t1805;
t2111 = t7.*t13.*t62.*(-5.5078125e-3);
t2112 = t12.*t1805;
t2124 = t20.*t63.*5.5078125e-3;
t2125 = t21.*t1323;
t2126 = t22.*t1323;
t2136 = t18.*t50.*t62.*(-9.0./2.0e+2);
t2137 = t3.*t20.*t48.*9.325e-3;
t2141 = -t2024;
t2142 = t10.*t21.*t48.*3.73e-2;
t2143 = t2.*t6.*t12.*t19.*3.73e-2;
t2145 = t2.*t5.*t11.*t19.*1.865e-2;
t2146 = t3.*t4.*t10.*t21.*1.865e-2;
t2153 = t3.*t27.*t48.*9.325e-3;
t2154 = t3.*t20.*t53.*9.325e-3;
t2155 = t20.*t1599;
t2163 = t10.*t21.*t53.*3.73e-2;
t2164 = t6.*t8.*t12.*t19.*3.73e-2;
t2166 = t5.*t8.*t11.*t19.*1.865e-2;
t2167 = t4.*t9.*t10.*t21.*1.865e-2;
t2170 = t5.*t6.*t11.*t29.*5.5078125e-3;
t2174 = t3.*t27.*t53.*9.325e-3;
t2176 = t20.*t1625;
t2192 = t3.*t9.*t20.*1.37635;
t2193 = t5.*t11.*t18.*1.37635;
t2212 = t50.*t63.*(-2.75390625e-3);
t2214 = t51.*t63.*1.376953125e-3;
t2215 = t6.*t1918;
t2218 = t4.*t21.*1.491640625e-2;
t2221 = -t2062;
t2223 = t54.*t63.*1.376953125e-3;
t2224 = t55.*t63.*1.376953125e-3;
t2225 = t56.*t63.*1.376953125e-3;
t2226 = t10.*t1918;
t2231 = t60.*t63.*(-2.75390625e-3);
t2232 = t62.*t63.*1.376953125e-3;
t2233 = t11.*t1927;
t2235 = t18.*t20.*t62.*(-9.0./1.0e+2);
t2240 = t2.*t19.*t21.*1.865e-2;
t2241 = t3.*t19.*t21.*1.865e-2;
t2277 = t8.*t19.*t21.*1.865e-2;
t2278 = t3.*t21.*t26.*1.865e-2;
t2309 = t49.*t56.*6.88175e-1;
t2316 = t49.*t61.*6.88175e-1;
t2317 = t50.*t60.*6.88175e-1;
t2321 = t55.*t61.*6.88175e-1;
t2323 = t11.*t18.*t21.*t26.*(-3.0./5.0e+1);
t2324 = t22.*t63.*(-2.75390625e-3);
t2327 = t18.*t19.*t20.*(-3.9e+1./2.0e+2);
t2328 = t12.*t58.*2.98328125e-2;
t2331 = t10.*t20.*t48.*(-1.865e-2);
t2334 = t3.*t4.*t10.*t20.*(-9.325e-3);
t2343 = t6.*t7.*t13.*t27.*(-5.5078125e-3);
t2357 = t7.*t49.*t1323;
t2361 = t11.*t50.*t63.*5.5078125e-3;
t2366 = t7.*t54.*t1323;
t2369 = t7.*t56.*t1323;
t2371 = t13.*t51.*t1323;
t2372 = t7.*t57.*t1323;
t2378 = t4.*t10.*t20.*(-6.88175e-1);
t2379 = t5.*t11.*t19.*(-6.88175e-1);
t2382 = t4.*t10.*t21.*5.9665625e-2;
t2383 = t6.*t12.*t19.*5.9665625e-2;
t2387 = t3.*t4.*t10.*t20.*t21.*(-3.0./1.0e+2);
t2389 = t11.*t55.*t63.*5.5078125e-3;
t2391 = t13.*t54.*t1323;
t2395 = t13.*t56.*t1323;
t2398 = t7.*t61.*t1323;
t2402 = t7.*t62.*t1323;
t2409 = t3.*t10.*t27.*3.440875e-1;
t2412 = t3.*t4.*t10.*t20.*t28.*(-3.0./1.0e+2);
t2419 = t13.*t62.*t1323;
t2429 = t3.*t19.*t20.*(-9.325e-3);
t2430 = t3.*t19.*t22.*(-2.75390625e-3);
t2431 = t3.*t20.*t22.*(-2.75390625e-3);
t2432 = t4.*t20.*t22.*(-2.75390625e-3);
t2433 = t5.*t21.*t22.*(-2.75390625e-3);
t2450 = t4.*t22.*t27.*(-2.75390625e-3);
t2451 = t5.*t22.*t28.*(-2.75390625e-3);
t2453 = t58.*t1803;
t2454 = t54.*t1806;
t2466 = t3.*t20.*t1323;
t2467 = t4.*t20.*t1323;
t2473 = t4.*t27.*t1323;
t2478 = t7.*t28.*t1323;
t2494 = t21.*t48.*t61.*1.865e-2;
t2495 = t11.*t19.*t1598;
t2496 = t6.*t12.*t19.*t54.*1.865e-2;
t2519 = t28.*t48.*t61.*1.865e-2;
t2520 = t21.*t53.*t61.*1.865e-2;
t2526 = t29.*t50.*t62.*5.5078125e-3;
t2540 = t28.*t53.*t61.*1.865e-2;
t2541 = t11.*t26.*t1618;
t2546 = t5.*t18.*t61.*6.88175e-1;
t2556 = t5.*t2213;
t2557 = t4.*t49.*t63.*1.376953125e-3;
t2560 = t3.*t9.*t10.*t27.*6.88175e-1;
t2561 = t5.*t25.*t61.*6.88175e-1;
t2566 = t7.*t54.*t63.*(-2.75390625e-3);
t2567 = t7.*t55.*t63.*(-2.75390625e-3);
t2568 = t7.*t56.*t63.*(-2.75390625e-3);
t2569 = t13.*t51.*t63.*(-2.75390625e-3);
t2570 = t7.*t58.*t63.*(-2.75390625e-3);
t2572 = t6.*t7.*t1926;
t2580 = t3.*t10.*t20.*(-3.440875e-1);
t2581 = t4.*t9.*t20.*(-3.440875e-1);
t2583 = t18.*t1846;
t2585 = t20.*t1846;
t2586 = t3.*t10.*t21.*1.491640625e-2;
t2588 = t21.*t54.*1.491640625e-2;
t2589 = t21.*t55.*1.491640625e-2;
t2590 = t21.*t56.*1.491640625e-2;
t2591 = t5.*t10.*t21.*1.491640625e-2;
t2593 = t18.*t19.*t1132;
t2595 = t13.*t54.*t63.*(-2.75390625e-3);
t2597 = t13.*t55.*t63.*(-2.75390625e-3);
t2598 = t13.*t56.*t63.*(-2.75390625e-3);
t2599 = t13.*t57.*t63.*(-2.75390625e-3);
t2600 = t7.*t13.*t1925;
t2601 = t10.*t2222;
t2602 = t7.*t13.*t1926;
t2603 = t12.*t2222;
t2607 = t4.*t9.*t27.*(-3.440875e-1);
t2608 = t28.*t54.*1.491640625e-2;
t2609 = t28.*t55.*1.491640625e-2;
t2610 = t28.*t56.*1.491640625e-2;
t2611 = t5.*t10.*t28.*1.491640625e-2;
t2614 = t13.*t62.*t63.*(-2.75390625e-3);
t2615 = t12.*t13.*t1926;
t2632 = t3.*t9.*t20.*t22.*1.1015625e-2;
t2633 = t5.*t11.*t18.*t22.*1.1015625e-2;
t2634 = t4.*t10.*t21.*t22.*1.1015625e-2;
t2635 = t7.*t13.*t18.*t20.*1.1015625e-2;
t2636 = t6.*t12.*t19.*t22.*1.1015625e-2;
t2637 = t7.*t13.*t19.*t21.*1.1015625e-2;
t2639 = t19.*t21.*t54.*1.865e-2;
t2646 = t20.*t29.*t51.*5.5078125e-3;
t2672 = t49.*t61.*t957;
t2684 = t2.*t9.*t21.*t26.*1.865e-2;
t2686 = t19.*t28.*t54.*1.865e-2;
t2708 = t8.*t9.*t21.*t26.*1.865e-2;
t2725 = t3.*t20.*t63.*(-2.75390625e-3);
t2726 = t4.*t20.*t63.*(-2.75390625e-3);
t2727 = t7.*t21.*t63.*(-2.75390625e-3);
t2729 = t22.*t1917;
t2730 = t4.*t21.*t63.*1.376953125e-3;
t2731 = t4.*t22.*t63.*1.376953125e-3;
t2732 = t21.*t1918;
t2733 = t22.*t1918;
t2735 = t54.*t1846;
t2738 = t4.*t27.*t63.*(-2.75390625e-3);
t2740 = t26.*t1917;
t2741 = t28.*t1918;
t2742 = t22.*t1927;
t2746 = t29.*t1927;
t2749 = t7.*t13.*t20.*t51.*1.1015625e-2;
t2762 = t3.*t10.*t21.*t53.*(-1.865e-2);
t2765 = t6.*t12.*t22.*t54.*(-5.5078125e-3);
t2769 = t7.*t13.*t20.*t57.*(-5.5078125e-3);
t2771 = t3.*t10.*t20.*t53.*(-9.325e-3);
t2779 = t2.*t6.*t11.*t12.*t26.*(-1.865e-2);
t2780 = t6.*t8.*t11.*t12.*t19.*(-1.865e-2);
t2785 = t6.*t27.*t1803;
t2786 = t5.*t26.*t1806;
t2788 = t21.*t55.*t61.*(-9.325e-3);
t2791 = t49.*t56.*t63.*5.5078125e-3;
t2792 = t5.*t2362;
t2793 = t4.*t13.*t49.*t1323;
t2822 = t18.*t19.*t20.*t21.*(-3.0./1.0e+2);
t2823 = t49.*t61.*t63.*5.5078125e-3;
t2824 = t50.*t60.*t63.*5.5078125e-3;
t2825 = t7.*t12.*t58.*t63.*5.5078125e-3;
t2854 = t3.*t9.*t10.*t20.*(-6.88175e-1);
t2867 = t3.*t4.*t21.*(-2.98328125e-2);
t2868 = t55.*t61.*t63.*5.5078125e-3;
t2869 = t12.*t13.*t2062;
t2899 = t5.*t11.*t21.*(-2.98328125e-2);
t2900 = t6.*t12.*t20.*(-2.98328125e-2);
t2902 = t4.*t9.*t21.*(-1.491640625e-2);
t2933 = t6.*t12.*t18.*t22.*(-5.5078125e-3);
t2935 = t4.*t9.*t20.*t21.*(-9.325e-3);
t2939 = t21.*t22.*t54.*(-2.75390625e-3);
t2942 = t7.*t13.*t49.*t61.*(-5.5078125e-3);
t2948 = t2.*t9.*t20.*t26.*(-9.325e-3);
t2951 = t22.*t28.*t54.*(-2.75390625e-3);
t2952 = t22.*t28.*t55.*(-2.75390625e-3);
t2953 = t22.*t28.*t56.*(-2.75390625e-3);
t2961 = t5.*t7.*t21.*t63.*5.5078125e-3;
t2967 = t8.*t9.*t20.*t26.*(-9.325e-3);
t2968 = t9.*t49.*t56.*(-6.88175e-1);
t2974 = t3.*t9.*t20.*t63.*1.1015625e-2;
t2975 = t5.*t11.*t18.*t63.*1.1015625e-2;
t2977 = t4.*t10.*t21.*t63.*5.5078125e-3;
t2978 = t19.*t2062;
t2979 = t6.*t12.*t19.*t63.*5.5078125e-3;
t3002 = t3.*t10.*t27.*t1323;
t3010 = t3.*t19.*t63.*(-1.376953125e-3);
t3011 = t3.*t22.*t63.*(-1.376953125e-3);
t3013 = t5.*t21.*t63.*(-1.376953125e-3);
t3015 = t5.*t12.*t58.*(-2.98328125e-2);
t3016 = t5.*t28.*t63.*(-1.376953125e-3);
t3017 = t12.*t22.*t63.*(-1.376953125e-3);
t3020 = t12.*t29.*t63.*(-1.376953125e-3);
t3021 = t3.*t10.*t21.*t48.*(-1.865e-2);
t3023 = t3.*t10.*t20.*t48.*(-9.325e-3);
t3034 = t4.*t7.*t49.*t63.*(-2.75390625e-3);
t3049 = t7.*t50.*t1925;
t3052 = t3.*t4.*t2222;
t3054 = t51.*t2222;
t3056 = t4.*t28.*t49.*1.491640625e-2;
t3058 = t20.*t21.*t63.*(-2.75390625e-3);
t3067 = t6.*t12.*t54.*t63.*(-2.75390625e-3);
t3075 = t5.*t13.*t58.*t63.*(-2.75390625e-3);
t3077 = t5.*t6.*t13.*t1926;
t3078 = t58.*t2222;
t3099 = t62.*t2222;
t3101 = t10.*t28.*t56.*2.98328125e-2;
t3102 = t11.*t26.*t1846;
t3109 = t13.*t62.*t1925;
t3118 = t19.*t20.*t1598;
t3138 = t5.*t6.*t11.*t18.*t29.*1.1015625e-2;
t3139 = t6.*t7.*t13.*t18.*t27.*1.1015625e-2;
t3143 = t19.*t20.*t1618;
t3192 = t3.*t20.*t21.*1.491640625e-2;
t3204 = t4.*t10.*t20.*t63.*(-5.5078125e-3);
t3206 = t5.*t11.*t19.*t63.*(-5.5078125e-3);
t3208 = t3.*t19.*t1925;
t3210 = t3.*t21.*t1925;
t3211 = t4.*t20.*t1925;
t3212 = t3.*t22.*t1925;
t3213 = t6.*t12.*t18.*t63.*(-2.75390625e-3);
t3214 = t6.*t12.*t20.*t63.*(-2.75390625e-3);
t3216 = t5.*t13.*t21.*t63.*(-2.75390625e-3);
t3217 = t10.*t21.*t1917;
t3231 = t3.*t20.*t26.*(-3.440875e-1);
t3245 = t4.*t27.*t1925;
t3246 = t7.*t26.*t1926;
t3262 = t12.*t13.*t27.*t63.*(-2.75390625e-3);
t3272 = t3.*t4.*t7.*t10.*t13.*t21.*1.1015625e-2;
t3298 = t7.*t9.*t13.*t20.*t58.*1.1015625e-2;
t3299 = t5.*t7.*t11.*t12.*t13.*t18.*1.1015625e-2;
t3320 = t7.*t51.*t62.*t63.*1.1015625e-2;
t3326 = t54.*t2362;
t3330 = t6.*t7.*t12.*t2062;
t3388 = t7.*t19.*t28.*t63.*5.5078125e-3;
t3396 = t4.*t21.*t49.*(-1.491640625e-2);
t3453 = t11.*t21.*t50.*(-2.98328125e-2);
t3470 = t10.*t21.*t56.*(-2.98328125e-2);
t3471 = t11.*t21.*t55.*(-2.98328125e-2);
t3473 = t6.*t11.*t12.*t19.*(-2.98328125e-2);
t3479 = t3.*t20.*t21.*t48.*(-9.325e-3);
t3480 = t4.*t21.*t22.*t49.*(-2.75390625e-3);
t3483 = t3.*t4.*t10.*t21.*t22.*(-1.1015625e-2);
t3484 = t5.*t6.*t11.*t18.*t22.*(-1.1015625e-2);
t3485 = t6.*t7.*t13.*t18.*t20.*(-1.1015625e-2);
t3486 = t2.*t5.*t11.*t19.*t21.*(-1.865e-2);
t3490 = t3.*t20.*t21.*t53.*(-9.325e-3);
t3491 = t4.*t22.*t28.*t49.*(-2.75390625e-3);
t3497 = t10.*t20.*t21.*t53.*(-1.865e-2);
t3498 = t5.*t18.*t22.*t61.*(-5.5078125e-3);
t3501 = t5.*t6.*t11.*t19.*t29.*(-5.5078125e-3);
t3510 = t7.*t21.*t49.*t63.*5.5078125e-3;
t3511 = t7.*t21.*t50.*t63.*5.5078125e-3;
t3521 = t6.*t11.*t12.*t22.*t26.*(-5.5078125e-3);
t3526 = t7.*t19.*t54.*t63.*5.5078125e-3;
t3527 = t7.*t21.*t54.*t63.*5.5078125e-3;
t3528 = t7.*t21.*t55.*t63.*5.5078125e-3;
t3529 = t7.*t21.*t56.*t63.*5.5078125e-3;
t3546 = t3.*t9.*t19.*t21.*5.9665625e-2;
t3547 = t3.*t9.*t20.*t21.*5.9665625e-2;
t3549 = t5.*t11.*t18.*t21.*5.9665625e-2;
t3551 = t6.*t12.*t18.*t20.*5.9665625e-2;
t3559 = t5.*t18.*t61.*t63.*5.5078125e-3;
t3560 = t7.*t21.*t60.*t63.*5.5078125e-3;
t3562 = t7.*t21.*t61.*t63.*5.5078125e-3;
t3589 = t5.*t6.*t22.*t63.*(-1.376953125e-3);
t3590 = t3.*t19.*t21.*(-2.98328125e-2);
t3592 = t4.*t20.*t21.*(-1.491640625e-2);
t3593 = t10.*t27.*t2061;
t3594 = t5.*t25.*t61.*t63.*5.5078125e-3;
t3595 = t10.*t28.*t56.*t1323;
t3608 = t3.*t10.*t21.*t63.*(-1.376953125e-3);
t3609 = t21.*t54.*t63.*(-1.376953125e-3);
t3611 = t4.*t9.*t22.*t63.*(-1.376953125e-3);
t3612 = t22.*t54.*t63.*(-1.376953125e-3);
t3613 = t21.*t2423;
t3614 = t22.*t56.*t63.*(-1.376953125e-3);
t3615 = t29.*t51.*t63.*(-1.376953125e-3);
tau = ft_2({dq1,dq2,dq3,dq4,dq5,dq6,t10,t100,t1001,t1005,t1009,t101,t1018,t102,t1022,t103,t1031,t104,t1040,t1041,t105,t106,t107,t1073,t1076,t1077,t1078,t108,t109,t1095,t1096,t1098,t11,t110,t111,t1110,t1114,t112,t1123,t1125,t113,t1131,t1132,t1134,t114,t115,t1158,t116,t1160,t1162,t1163,t1169,t117,t1170,t1171,t1172,t1173,t1175,t118,t1180,t1184,t1186,t1189,t119,t1191,t1196,t1197,t1198,t1199,t12,t120,t1200,t1201,t1204,t1205,t1207,t1208,t121,t1211,t1214,t1219,t122,t1220,t1221,t1222,t1223,t1224,t1225,t1228,t1229,t123,t1230,t1231,t1233,t1234,t1236,t1237,t1238,t1239,t124,t1240,t1242,t1246,t1247,t125,t126,t1266,t127,t128,t129,t1294,t1295,t1297,t1298,t13,t130,t131,t132,t1322,t1323,t133,t134,t1347,t1348,t135,t1357,t136,t1361,t1362,t1363,t1366,t137,t138,t1384,t1385,t139,t1397,t1398,t140,t141,t1413,t142,t1427,t1429,t143,t1434,t1438,t144,t145,t1450,t1456,t1457,t1458,t146,t1462,t1464,t1465,t1467,t147,t1473,t1474,t1475,t1476,t1477,t1478,t1479,t148,t1480,t1481,t1485,t1486,t1487,t1488,t1489,t149,t1490,t1493,t1494,t1497,t150,t1502,t151,t152,t1528,t153,t1532,t1538,t154,t155,t1557,t1558,t156,t158,t1581,t1582,t159,t1597,t1598,t1599,t160,t161,t1617,t1618,t1619,t162,t1620,t1621,t1622,t163,t1638,t164,t1643,t1651,t1660,t167,t168,t1684,t1685,t1689,t169,t1696,t1702,t171,t1713,t1719,t172,t1720,t1726,t173,t1730,t1732,t1733,t174,t1740,t1741,t1747,t1748,t1756,t1757,t1760,t177,t1772,t1773,t1774,t1776,t178,t1785,t179,t18,t180,t1801,t1803,t1804,t1805,t1806,t1808,t181,t182,t1822,t1823,t1828,t183,t1831,t1832,t1839,t184,t1840,t1845,t1849,t185,t1852,t1853,t1858,t186,t1861,t1866,t1867,t1869,t187,t1870,t1872,t1873,t1876,t1877,t1878,t188,t1880,t1881,t1884,t1886,t1887,t1888,t189,t1890,t1891,t1893,t1897,t1899,t19,t190,t191,t1917,t1919,t192,t1925,t1926,t1927,t194,t1944,t1947,t1948,t1949,t195,t1950,t1951,t196,t1962,t1963,t1967,t1968,t1969,t197,t1978,t1979,t198,t1983,t1989,t199,t1999,t2,t20,t2001,t2002,t2008,t201,t2014,t202,t2023,t2024,t2025,t203,t2030,t2031,t2034,t2035,t2036,t2037,t204,t2046,t2052,t2053,t2055,t2056,t2058,t206,t2061,t2062,t2063,t2064,t2065,t2066,t207,t2070,t2071,t2072,t2076,t2078,t208,t2085,t2086,t209,t2091,t2092,t2094,t2096,t2097,t21,t210,t211,t2111,t2112,t2124,t2125,t2126,t2136,t2137,t214,t2141,t2142,t2143,t2145,t2146,t215,t2153,t2154,t2155,t2163,t2164,t2166,t2167,t2170,t2174,t2176,t2192,t2193,t22,t2212,t2213,t2214,t2215,t2218,t2221,t2222,t2223,t2224,t2225,t2226,t2231,t2232,t2233,t2235,t2240,t2241,t2250,t227,t2277,t2278,t228,t229,t230,t2309,t231,t2316,t2317,t2321,t2323,t2324,t2327,t2328,t233,t2331,t2334,t2343,t2357,t2361,t2362,t2366,t2369,t2371,t2372,t2378,t2379,t2382,t2383,t2387,t2389,t2391,t2395,t2398,t2402,t2409,t2412,t2419,t242,t2423,t2425,t2429,t243,t2430,t2431,t2432,t2433,t245,t2450,t2451,t2453,t2454,t246,t2466,t2467,t2473,t2478,t248,t249,t2494,t2495,t2496,t25,t250,t251,t2519,t252,t2520,t2526,t253,t254,t2540,t2541,t2546,t255,t2556,t2557,t256,t2560,t2561,t2566,t2567,t2568,t2569,t2570,t2571,t2572,t258,t2580,t2581,t2583,t2585,t2586,t2588,t2589,t259,t2590,t2591,t2593,t2595,t2597,t2598,t2599,t26,t260,t2600,t2601,t2602,t2603,t2607,t2608,t2609,t261,t2610,t2611,t2614,t2615,t262,t263,t2632,t2633,t2634,t2635,t2636,t2637,t2639,t264,t2646,t265,t267,t2672,t268,t2684,t2686,t27,t2708,t2725,t2726,t2727,t2729,t2730,t2731,t2732,t2733,t2735,t2738,t2740,t2741,t2742,t2746,t2749,t2762,t2765,t2769,t2771,t2779,t2780,t2785,t2786,t2788,t2791,t2792,t2793,t28,t282,t2822,t2823,t2824,t2825,t2854,t2867,t2868,t2869,t2899,t29,t2900,t2902,t291,t2933,t2935,t2939,t2942,t2948,t2951,t2952,t2953,t2961,t2967,t2968,t2974,t2975,t2977,t2978,t2979,t3,t30,t3002,t3010,t3011,t3013,t3015,t3016,t3017,t3020,t3021,t3023,t3034,t3047,t3049,t3052,t3054,t3056,t3058,t3067,t3075,t3077,t3078,t308,t309,t3099,t31,t3101,t3102,t3109,t311,t3118,t312,t313,t3138,t3139,t3143,t318,t3192,t32,t3204,t3206,t3208,t321,t3210,t3211,t3212,t3213,t3214,t3216,t3217,t322,t3231,t3245,t3246,t325,t3262,t3272,t3298,t3299,t33,t331,t332,t3320,t3326,t333,t3330,t334,t338,t3388,t339,t3396,t34,t341,t342,t343,t344,t345,t3453,t346,t347,t3470,t3471,t3473,t3479,t348,t3480,t3483,t3484,t3485,t3486,t349,t3490,t3491,t3497,t3498,t35,t350,t3501,t3510,t3511,t352,t3521,t3526,t3527,t3528,t3529,t3546,t3547,t3549,t355,t3551,t3559,t356,t3560,t3562,t357,t358,t3589,t359,t3590,t3592,t3593,t3594,t3595,t3608,t3609,t361,t3611,t3612,t3613,t3614,t3615,t3690,t371,t377,t381,t384,t389,t390,t4,t406,t408,t413,t420,t421,t425,t427,t429,t436,t443,t444,t460,t463,t464,t468,t474,t475,t478,t479,t48,t482,t484,t486,t49,t490,t491,t493,t494,t499,t5,t50,t500,t502,t503,t51,t514,t517,t518,t519,t52,t520,t521,t522,t524,t525,t526,t527,t528,t529,t53,t530,t531,t532,t533,t534,t54,t55,t56,t57,t58,t585,t59,t592,t594,t595,t597,t598,t6,t60,t603,t61,t614,t615,t62,t63,t636,t643,t649,t65,t652,t66,t663,t664,t665,t666,t667,t668,t67,t670,t671,t672,t673,t6734,t6735,t6736,t675,t6754,t677,t679,t680,t681,t682,t683,t684,t685,t686,t691,t692,t693,t695,t696,t697,t698,t7,t701,t702,t703,t704,t705,t708,t715,t720,t731,t732,t734,t753,t755,t762,t789,t790,t793,t795,t8,t82,t828,t829,t83,t834,t835,t84,t85,t86,t861,t863,t864,t87,t88,t887,t888,t89,t894,t897,t899,t9,t90,t900,t902,t905,t909,t913,t915,t916,t92,t93,t931,t933,t936,t939,t95,t954,t955,t956,t957,t958,t959,t96,t960,t961,t962,t963,t964,t966,t967,t968,t97,t971,t973,t979,t98,t982,t983,t984,t988,t99,t992,t993,t997,t998,t999});
end
function tau = ft_2(ct)
[dq1,dq2,dq3,dq4,dq5,dq6,t10,t100,t1001,t1005,t1009,t101,t1018,t102,t1022,t103,t1031,t104,t1040,t1041,t105,t106,t107,t1073,t1076,t1077,t1078,t108,t109,t1095,t1096,t1098,t11,t110,t111,t1110,t1114,t112,t1123,t1125,t113,t1131,t1132,t1134,t114,t115,t1158,t116,t1160,t1162,t1163,t1169,t117,t1170,t1171,t1172,t1173,t1175,t118,t1180,t1184,t1186,t1189,t119,t1191,t1196,t1197,t1198,t1199,t12,t120,t1200,t1201,t1204,t1205,t1207,t1208,t121,t1211,t1214,t1219,t122,t1220,t1221,t1222,t1223,t1224,t1225,t1228,t1229,t123,t1230,t1231,t1233,t1234,t1236,t1237,t1238,t1239,t124,t1240,t1242,t1246,t1247,t125,t126,t1266,t127,t128,t129,t1294,t1295,t1297,t1298,t13,t130,t131,t132,t1322,t1323,t133,t134,t1347,t1348,t135,t1357,t136,t1361,t1362,t1363,t1366,t137,t138,t1384,t1385,t139,t1397,t1398,t140,t141,t1413,t142,t1427,t1429,t143,t1434,t1438,t144,t145,t1450,t1456,t1457,t1458,t146,t1462,t1464,t1465,t1467,t147,t1473,t1474,t1475,t1476,t1477,t1478,t1479,t148,t1480,t1481,t1485,t1486,t1487,t1488,t1489,t149,t1490,t1493,t1494,t1497,t150,t1502,t151,t152,t1528,t153,t1532,t1538,t154,t155,t1557,t1558,t156,t158,t1581,t1582,t159,t1597,t1598,t1599,t160,t161,t1617,t1618,t1619,t162,t1620,t1621,t1622,t163,t1638,t164,t1643,t1651,t1660,t167,t168,t1684,t1685,t1689,t169,t1696,t1702,t171,t1713,t1719,t172,t1720,t1726,t173,t1730,t1732,t1733,t174,t1740,t1741,t1747,t1748,t1756,t1757,t1760,t177,t1772,t1773,t1774,t1776,t178,t1785,t179,t18,t180,t1801,t1803,t1804,t1805,t1806,t1808,t181,t182,t1822,t1823,t1828,t183,t1831,t1832,t1839,t184,t1840,t1845,t1849,t185,t1852,t1853,t1858,t186,t1861,t1866,t1867,t1869,t187,t1870,t1872,t1873,t1876,t1877,t1878,t188,t1880,t1881,t1884,t1886,t1887,t1888,t189,t1890,t1891,t1893,t1897,t1899,t19,t190,t191,t1917,t1919,t192,t1925,t1926,t1927,t194,t1944,t1947,t1948,t1949,t195,t1950,t1951,t196,t1962,t1963,t1967,t1968,t1969,t197,t1978,t1979,t198,t1983,t1989,t199,t1999,t2,t20,t2001,t2002,t2008,t201,t2014,t202,t2023,t2024,t2025,t203,t2030,t2031,t2034,t2035,t2036,t2037,t204,t2046,t2052,t2053,t2055,t2056,t2058,t206,t2061,t2062,t2063,t2064,t2065,t2066,t207,t2070,t2071,t2072,t2076,t2078,t208,t2085,t2086,t209,t2091,t2092,t2094,t2096,t2097,t21,t210,t211,t2111,t2112,t2124,t2125,t2126,t2136,t2137,t214,t2141,t2142,t2143,t2145,t2146,t215,t2153,t2154,t2155,t2163,t2164,t2166,t2167,t2170,t2174,t2176,t2192,t2193,t22,t2212,t2213,t2214,t2215,t2218,t2221,t2222,t2223,t2224,t2225,t2226,t2231,t2232,t2233,t2235,t2240,t2241,t2250,t227,t2277,t2278,t228,t229,t230,t2309,t231,t2316,t2317,t2321,t2323,t2324,t2327,t2328,t233,t2331,t2334,t2343,t2357,t2361,t2362,t2366,t2369,t2371,t2372,t2378,t2379,t2382,t2383,t2387,t2389,t2391,t2395,t2398,t2402,t2409,t2412,t2419,t242,t2423,t2425,t2429,t243,t2430,t2431,t2432,t2433,t245,t2450,t2451,t2453,t2454,t246,t2466,t2467,t2473,t2478,t248,t249,t2494,t2495,t2496,t25,t250,t251,t2519,t252,t2520,t2526,t253,t254,t2540,t2541,t2546,t255,t2556,t2557,t256,t2560,t2561,t2566,t2567,t2568,t2569,t2570,t2571,t2572,t258,t2580,t2581,t2583,t2585,t2586,t2588,t2589,t259,t2590,t2591,t2593,t2595,t2597,t2598,t2599,t26,t260,t2600,t2601,t2602,t2603,t2607,t2608,t2609,t261,t2610,t2611,t2614,t2615,t262,t263,t2632,t2633,t2634,t2635,t2636,t2637,t2639,t264,t2646,t265,t267,t2672,t268,t2684,t2686,t27,t2708,t2725,t2726,t2727,t2729,t2730,t2731,t2732,t2733,t2735,t2738,t2740,t2741,t2742,t2746,t2749,t2762,t2765,t2769,t2771,t2779,t2780,t2785,t2786,t2788,t2791,t2792,t2793,t28,t282,t2822,t2823,t2824,t2825,t2854,t2867,t2868,t2869,t2899,t29,t2900,t2902,t291,t2933,t2935,t2939,t2942,t2948,t2951,t2952,t2953,t2961,t2967,t2968,t2974,t2975,t2977,t2978,t2979,t3,t30,t3002,t3010,t3011,t3013,t3015,t3016,t3017,t3020,t3021,t3023,t3034,t3047,t3049,t3052,t3054,t3056,t3058,t3067,t3075,t3077,t3078,t308,t309,t3099,t31,t3101,t3102,t3109,t311,t3118,t312,t313,t3138,t3139,t3143,t318,t3192,t32,t3204,t3206,t3208,t321,t3210,t3211,t3212,t3213,t3214,t3216,t3217,t322,t3231,t3245,t3246,t325,t3262,t3272,t3298,t3299,t33,t331,t332,t3320,t3326,t333,t3330,t334,t338,t3388,t339,t3396,t34,t341,t342,t343,t344,t345,t3453,t346,t347,t3470,t3471,t3473,t3479,t348,t3480,t3483,t3484,t3485,t3486,t349,t3490,t3491,t3497,t3498,t35,t350,t3501,t3510,t3511,t352,t3521,t3526,t3527,t3528,t3529,t3546,t3547,t3549,t355,t3551,t3559,t356,t3560,t3562,t357,t358,t3589,t359,t3590,t3592,t3593,t3594,t3595,t3608,t3609,t361,t3611,t3612,t3613,t3614,t3615,t3690,t371,t377,t381,t384,t389,t390,t4,t406,t408,t413,t420,t421,t425,t427,t429,t436,t443,t444,t460,t463,t464,t468,t474,t475,t478,t479,t48,t482,t484,t486,t49,t490,t491,t493,t494,t499,t5,t50,t500,t502,t503,t51,t514,t517,t518,t519,t52,t520,t521,t522,t524,t525,t526,t527,t528,t529,t53,t530,t531,t532,t533,t534,t54,t55,t56,t57,t58,t585,t59,t592,t594,t595,t597,t598,t6,t60,t603,t61,t614,t615,t62,t63,t636,t643,t649,t65,t652,t66,t663,t664,t665,t666,t667,t668,t67,t670,t671,t672,t673,t6734,t6735,t6736,t675,t6754,t677,t679,t680,t681,t682,t683,t684,t685,t686,t691,t692,t693,t695,t696,t697,t698,t7,t701,t702,t703,t704,t705,t708,t715,t720,t731,t732,t734,t753,t755,t762,t789,t790,t793,t795,t8,t82,t828,t829,t83,t834,t835,t84,t85,t86,t861,t863,t864,t87,t88,t887,t888,t89,t894,t897,t899,t9,t90,t900,t902,t905,t909,t913,t915,t916,t92,t93,t931,t933,t936,t939,t95,t954,t955,t956,t957,t958,t959,t96,t960,t961,t962,t963,t964,t966,t967,t968,t97,t971,t973,t979,t98,t982,t983,t984,t988,t99,t992,t993,t997,t998,t999] = ct{:};
t3616 = t5.*t6.*t29.*t63.*(-1.376953125e-3);
t3617 = t4.*t21.*t27.*(-1.491640625e-2);
t3627 = t28.*t54.*t63.*(-1.376953125e-3);
t3628 = t28.*t55.*t63.*(-1.376953125e-3);
t3629 = t28.*t56.*t63.*(-1.376953125e-3);
t3630 = t28.*t2423;
t3635 = t29.*t62.*t63.*(-1.376953125e-3);
t3636 = t29.*t2425;
t3637 = t2.*t19.*t20.*t21.*(-9.325e-3);
t3648 = t3.*t21.*t22.*t26.*(-5.5078125e-3);
t3650 = t8.*t19.*t20.*t21.*(-9.325e-3);
t3651 = t3.*t20.*t21.*t26.*(-9.325e-3);
t3680 = t7.*t19.*t21.*t63.*5.5078125e-3;
t3687 = t9.*t49.*t56.*t63.*(-5.5078125e-3);
t3691 = t6.*t7.*t12.*t54.*t63.*(-5.5078125e-3);
t3692 = t5.*t7.*t12.*t58.*t63.*(-5.5078125e-3);
t3704 = t6.*t12.*t19.*t54.*(-5.9665625e-2);
t3705 = t4.*t9.*t28.*t49.*2.98328125e-2;
t3722 = t3.*t21.*t26.*t63.*(-2.75390625e-3);
t3723 = t20.*t21.*t1925;
t3724 = t20.*t22.*t1925;
t3725 = t7.*t18.*t28.*t63.*(-2.75390625e-3);
t3726 = t7.*t20.*t28.*t63.*(-2.75390625e-3);
t3779 = t7.*t13.*t49.*t51.*t61.*1.1015625e-2;
t3796 = t7.*t13.*t20.*t25.*t58.*1.1015625e-2;
t3811 = t7.*t19.*t49.*t63.*(-2.75390625e-3);
t3822 = t3.*t4.*t10.*t21.*t63.*(-5.5078125e-3);
t3823 = t5.*t7.*t10.*t21.*t63.*(-5.5078125e-3);
t3824 = t6.*t7.*t12.*t20.*t63.*(-5.5078125e-3);
t3827 = t7.*t20.*t57.*t63.*(-2.75390625e-3);
t3828 = t19.*t2571;
t3839 = t6.*t12.*t18.*t19.*(-5.9665625e-2);
t3862 = t3.*t9.*t10.*t20.*t63.*(-5.5078125e-3);
t3865 = t6.*t12.*t13.*t19.*t63.*(-5.5078125e-3);
t3868 = t6.*t12.*t20.*t1925;
t3871 = t5.*t6.*t29.*t1926;
t3872 = t13.*t27.*t2213;
t3884 = t19.*t28.*t54.*2.98328125e-2;
t3909 = t10.*t28.*t56.*t63.*(-2.75390625e-3);
t3910 = t6.*t12.*t26.*t1926;
t3932 = t12.*t13.*t27.*t1925;
t3935 = t3.*t9.*t19.*t21.*t22.*1.1015625e-2;
t3941 = t6.*t12.*t18.*t20.*t22.*1.1015625e-2;
t3960 = t6.*t7.*t12.*t13.*t19.*t54.*1.1015625e-2;
t3963 = t29.*t49.*t51.*t61.*5.5078125e-3;
t4031 = t20.*t21.*t1917;
t4042 = t21.*t49.*t61.*(-2.98328125e-2);
t4043 = t21.*t50.*t60.*(-2.98328125e-2);
t4046 = t4.*t21.*t27.*t63.*(-1.376953125e-3);
t4047 = t4.*t22.*t27.*t63.*(-1.376953125e-3);
t4057 = t21.*t55.*t61.*(-2.98328125e-2);
t4060 = t7.*t13.*t18.*t20.*t58.*(-1.1015625e-2);
t4061 = t4.*t9.*t22.*t28.*t49.*(-5.5078125e-3);
t4067 = t18.*t29.*t50.*t62.*(-5.5078125e-3);
t4075 = t3.*t19.*t2362;
t4103 = t3.*t4.*t7.*t10.*t28.*t63.*5.5078125e-3;
t4109 = t6.*t13.*t18.*t2062;
t4168 = t4.*t21.*t49.*t63.*(-1.376953125e-3);
t4174 = t10.*t13.*t21.*t56.*t63.*5.5078125e-3;
t4204 = t4.*t28.*t49.*t63.*(-1.376953125e-3);
t4208 = t19.*t21.*t54.*(-2.98328125e-2);
t4209 = t4.*t10.*t20.*t21.*(-2.98328125e-2);
t4212 = t3.*t10.*t20.*t21.*(-1.491640625e-2);
t4260 = t4.*t10.*t18.*t21.*t22.*(-1.1015625e-2);
t4261 = t5.*t11.*t18.*t21.*t22.*(-1.1015625e-2);
t4262 = t7.*t13.*t18.*t19.*t21.*(-1.1015625e-2);
t4263 = t7.*t13.*t18.*t20.*t21.*(-1.1015625e-2);
t4265 = t19.*t21.*t22.*t54.*(-5.5078125e-3);
t4280 = t19.*t22.*t28.*t54.*(-5.5078125e-3);
t4344 = t19.*t20.*t2061;
t4345 = t19.*t21.*t2061;
t4347 = t20.*t21.*t2061;
t4372 = t20.*t29.*t51.*t1323;
t4451 = t7.*t11.*t21.*t26.*t63.*5.5078125e-3;
t4452 = t19.*t28.*t54.*t1323;
t4456 = t4.*t9.*t21.*t49.*(-2.98328125e-2);
t4457 = t21.*t49.*t56.*(-2.98328125e-2);
t4475 = t3.*t20.*t21.*t63.*(-1.376953125e-3);
t4477 = t4.*t20.*t21.*t63.*(-1.376953125e-3);
t4478 = t4.*t20.*t22.*t63.*(-1.376953125e-3);
t4508 = t12.*t13.*t18.*t27.*t63.*5.5078125e-3;
t4539 = t4.*t7.*t21.*t54.*t63.*(-5.5078125e-3);
t4542 = t7.*t10.*t21.*t50.*t63.*(-5.5078125e-3);
t4544 = t4.*t13.*t21.*t49.*t63.*(-2.75390625e-3);
t4545 = t3.*t12.*t20.*t2213;
t4546 = t7.*t21.*t50.*t1926;
t4547 = t7.*t12.*t20.*t51.*t63.*(-2.75390625e-3);
t4565 = t3.*t6.*t7.*t12.*t26.*t63.*(-5.5078125e-3);
t4566 = t5.*t7.*t11.*t12.*t18.*t63.*(-5.5078125e-3);
t4568 = t4.*t28.*t49.*t1925;
t4579 = t7.*t28.*t50.*t1926;
t4581 = t7.*t12.*t27.*t51.*t63.*(-2.75390625e-3);
t4584 = t20.*t57.*t2222;
t4763 = t4.*t10.*t18.*t21.*t63.*(-5.5078125e-3);
t4765 = t5.*t11.*t18.*t21.*t63.*(-5.5078125e-3);
t4766 = t5.*t11.*t18.*t22.*t63.*(-5.5078125e-3);
t4768 = t7.*t13.*t18.*t20.*t63.*(-5.5078125e-3);
t4769 = t7.*t11.*t19.*t21.*t63.*(-5.5078125e-3);
t4770 = t6.*t12.*t19.*t22.*t63.*(-5.5078125e-3);
t4771 = t7.*t13.*t19.*t21.*t63.*(-5.5078125e-3);
t4773 = t19.*t21.*t54.*t63.*(-2.75390625e-3);
t4806 = t49.*t61.*t2222;
t4808 = t12.*t13.*t54.*t2213;
t4830 = t12.*t13.*t18.*t20.*t63.*(-5.5078125e-3);
t4831 = t19.*t28.*t54.*t63.*(-2.75390625e-3);
t4833 = t7.*t20.*t28.*t1925;
t4895 = t3.*t6.*t7.*t9.*t12.*t19.*t63.*1.1015625e-2;
t4898 = t6.*t7.*t12.*t19.*t54.*t63.*1.1015625e-2;
t4900 = t4.*t9.*t13.*t21.*t49.*t63.*5.5078125e-3;
t5041 = t3.*t9.*t10.*t20.*t21.*(-2.98328125e-2);
t5054 = t10.*t18.*t28.*t56.*(-2.98328125e-2);
t5055 = t5.*t21.*t25.*t61.*(-2.98328125e-2);
t5103 = t7.*t19.*t21.*t54.*t63.*1.1015625e-2;
t5175 = t13.*t19.*t21.*t54.*t63.*5.5078125e-3;
t5176 = t6.*t18.*t29.*t2062;
t5280 = t3.*t20.*t21.*t26.*(-1.491640625e-2);
t5343 = t7.*t18.*t19.*t21.*t63.*(-5.5078125e-3);
t5344 = t7.*t18.*t20.*t21.*t63.*(-5.5078125e-3);
t5354 = t7.*t18.*t51.*t62.*t63.*(-1.1015625e-2);
t5356 = t5.*t6.*t7.*t11.*t12.*t18.*t63.*(-1.1015625e-2);
t5361 = t3.*t4.*t21.*t63.*t1804;
t5411 = t7.*t28.*t49.*t61.*t63.*(-2.75390625e-3);
t5491 = t7.*t19.*t21.*t49.*t63.*(-5.5078125e-3);
t5492 = t7.*t18.*t21.*t50.*t63.*(-5.5078125e-3);
t5551 = t10.*t18.*t21.*t56.*t63.*(-2.75390625e-3);
t5552 = t5.*t18.*t21.*t61.*t63.*(-2.75390625e-3);
t5613 = t13.*t18.*t20.*t62.*t63.*(-5.5078125e-3);
t6023 = t29.*t49.*t51.*t61.*t63.*(-2.75390625e-3);
t6473 = t19.*t20.*t3690;
t6742 = -t6734;
t6743 = -t6736;
t6744 = t3.*t19.*5.900182291666667e-2;
t6745 = t3.*t26.*5.900182291666667e-2;
t6755 = t3.*t9.*t19.*1.180036458333333e-1;
t6772 = t4.*t10.*t18.*(-1.180036458333333e-1);
t81 = -t65;
t165 = -t133;
t166 = -t134;
t170 = -t136;
t193 = t8.*t97;
t200 = t9.*t106;
t212 = cos(t156);
t213 = -t113;
t216 = sin(t156);
t217 = -t115;
t218 = -t116;
t219 = -t118;
t220 = -t121;
t221 = -t123;
t222 = -t124;
t223 = -t126;
t224 = -t127;
t225 = -t129;
t226 = t11.*t88;
t234 = t83.*(2.0./5.0);
t235 = t84.*(2.0./5.0);
t236 = t85.*(2.0./5.0);
t237 = t83.*(6.0./5.0);
t238 = t84.*(6.0./5.0);
t239 = t85.*(6.0./5.0);
t240 = -t169;
t241 = -t172;
t244 = -t174;
t247 = -t178;
t269 = t95.*(2.0./5.0);
t270 = t96.*(2.0./5.0);
t272 = t95.*(6.0./5.0);
t273 = t96.*(6.0./5.0);
t274 = t101.*(2.0./5.0);
t275 = t102.*(2.0./5.0);
t276 = t103.*(2.0./5.0);
t277 = t104.*(2.0./5.0);
t278 = t105.*(2.0./5.0);
t279 = t106.*(2.0./5.0);
t280 = t4.*t133;
t281 = t107.*(2.0./5.0);
t283 = t101.*(6.0./5.0);
t284 = t102.*(6.0./5.0);
t285 = t103.*(6.0./5.0);
t286 = t104.*(6.0./5.0);
t287 = t105.*(6.0./5.0);
t288 = t106.*(6.0./5.0);
t289 = t4.*t135;
t290 = t107.*(6.0./5.0);
t292 = t117.*(2.0./5.0);
t293 = t118.*(2.0./5.0);
t294 = t119.*(2.0./5.0);
t295 = t120.*(2.0./5.0);
t296 = t121.*(2.0./5.0);
t297 = t122.*(2.0./5.0);
t298 = t123.*(2.0./5.0);
t299 = t124.*(2.0./5.0);
t300 = t117.*(6.0./5.0);
t301 = t118.*(6.0./5.0);
t302 = t119.*(6.0./5.0);
t303 = t120.*(6.0./5.0);
t304 = t121.*(6.0./5.0);
t305 = t122.*(6.0./5.0);
t306 = t123.*(6.0./5.0);
t307 = t124.*(6.0./5.0);
t314 = -t233;
t315 = t83./1.0e+1;
t316 = t84./1.0e+1;
t317 = t83.*(3.0./1.0e+1);
t319 = t85./1.0e+1;
t320 = t84.*(3.0./1.0e+1);
t323 = t85.*(3.0./1.0e+1);
t324 = t86./1.0e+1;
t326 = t86.*(3.0./1.0e+1);
t327 = t86.*(3.0./2.5e+1);
t328 = t87.*(3.0./2.5e+1);
t329 = t86.*(3.0./5.0e+1);
t330 = t87.*(3.0./5.0e+1);
t336 = -t251;
t337 = -t252;
t353 = -t264;
t354 = -t265;
t360 = -t268;
t364 = -t196;
t365 = -t198;
t367 = -t202;
t368 = t54.*t88;
t373 = t95./1.0e+1;
t375 = t96./1.0e+1;
t376 = t95.*(3.0./1.0e+1);
t378 = t4.*t160;
t379 = t96.*(3.0./1.0e+1);
t380 = t97./1.0e+1;
t382 = t4.*t161;
t383 = t98./1.0e+1;
t385 = t98.*(3.0./1.0e+1);
t386 = t97.*(3.0./2.5e+1);
t387 = t97.*(3.0./4.0e+1);
t388 = t97.*(3.0./5.0e+1);
t391 = -t207;
t392 = -t208;
t396 = -t282;
t397 = t101./1.0e+1;
t399 = t102./1.0e+1;
t400 = t103./1.0e+1;
t401 = t104./1.0e+1;
t402 = t105./1.0e+1;
t404 = t106./1.0e+1;
t405 = t101.*(3.0./1.0e+1);
t407 = t102.*(3.0./1.0e+1);
t409 = t4.*t169;
t410 = t103.*(3.0./1.0e+1);
t411 = t107./1.0e+1;
t412 = -t291;
t414 = t104.*(3.0./1.0e+1);
t415 = t105.*(3.0./1.0e+1);
t416 = t108./1.0e+1;
t417 = t109./1.0e+1;
t418 = t106.*(3.0./1.0e+1);
t419 = t110./1.0e+1;
t422 = t107.*(3.0./1.0e+1);
t423 = t111./1.0e+1;
t424 = t6.*t169;
t426 = t112./1.0e+1;
t430 = t111.*(3.0./1.0e+1);
t431 = t6.*t172;
t432 = t112.*(3.0./1.0e+1);
t433 = t109.*(3.0./2.5e+1);
t434 = t110.*(3.0./2.5e+1);
t435 = t111.*(3.0./2.5e+1);
t437 = t114.*(3.0./4.0e+1);
t438 = t3.*t177;
t439 = t109.*(3.0./5.0e+1);
t440 = t110.*(3.0./5.0e+1);
t441 = t111.*(3.0./5.0e+1);
t442 = t10.*t164;
t450 = t117./1.0e+1;
t451 = t118./1.0e+1;
t453 = t119./1.0e+1;
t454 = t120./1.0e+1;
t456 = t121./1.0e+1;
t458 = t122./1.0e+1;
t459 = t117.*(3.0./1.0e+1);
t461 = t118.*(3.0./1.0e+1);
t462 = t123./1.0e+1;
t465 = t119.*(3.0./1.0e+1);
t467 = t124./1.0e+1;
t469 = t120.*(3.0./1.0e+1);
t470 = t125./1.0e+1;
t471 = t121.*(3.0./1.0e+1);
t472 = t126./1.0e+1;
t473 = t122.*(3.0./1.0e+1);
t476 = t123.*(3.0./1.0e+1);
t477 = t12.*t169;
t480 = t124.*(3.0./1.0e+1);
t481 = t127./1.0e+1;
t483 = t128./1.0e+1;
t487 = t12.*t172;
t488 = t127.*(3.0./1.0e+1);
t489 = t128.*(3.0./1.0e+1);
t492 = t127.*(3.0./2.5e+1);
t495 = t127.*(3.0./4.0e+1);
t496 = t129.*(3.0./4.0e+1);
t497 = t125.*(3.0./5.0e+1);
t498 = t126.*(3.0./5.0e+1);
t501 = t130.*(3.0./5.0e+1);
t509 = t86.*(3.0./1.0e+2);
t510 = t87.*(3.0./1.0e+2);
t511 = t86.*(3.0./2.0e+2);
t512 = t87.*(3.0./2.0e+2);
t513 = t85.*(3.0./4.0e+2);
t515 = -t341;
t516 = -t342;
t523 = -t356;
t535 = -t359;
t536 = -t361;
t539 = t52.*t131;
t540 = t48.*t134;
t542 = t52.*t132;
t543 = t48.*t136;
t545 = t52.*t133;
t546 = t48.*t137;
t547 = t52.*t134;
t548 = t59.*t131;
t550 = t52.*t135;
t551 = t48.*t138;
t552 = t52.*t136;
t553 = t59.*t132;
t556 = t98.*(-3.0./5.0e+1);
t557 = t99.*(-3.0./5.0e+1);
t558 = t97.*(3.0./2.0e+2);
t559 = t98.*(3.0./2.0e+2);
t560 = t99.*(3.0./2.0e+2);
t561 = t4.*t233;
t562 = t52.*t137;
t563 = t59.*t133;
t565 = t59.*t134;
t566 = t52.*t138;
t567 = t59.*t135;
t569 = t59.*t136;
t574 = -t406;
t582 = -t420;
t589 = t109.*(-3.0./1.0e+1);
t590 = t110.*(-3.0./1.0e+1);
t599 = t108.*(3.0./1.0e+2);
t600 = t109.*(3.0./1.0e+2);
t601 = t110.*(3.0./1.0e+2);
t602 = t111.*(3.0./1.0e+2);
t604 = t109.*(3.0./2.0e+2);
t605 = t110.*(3.0./2.0e+2);
t606 = t111.*(3.0./2.0e+2);
t608 = t112.*(3.0./2.0e+2);
t609 = t113.*(3.0./2.0e+2);
t610 = t114.*(3.0./2.0e+2);
t611 = t5.*t252;
t613 = t107.*(3.0./4.0e+2);
t616 = t59.*t137;
t617 = t59.*t138;
t624 = -t463;
t630 = -t478;
t632 = t126.*(-3.0./1.0e+1);
t635 = -t493;
t641 = t3.*t260;
t644 = t127.*(3.0./1.0e+2);
t645 = t5.*t261;
t647 = t125.*(3.0./2.0e+2);
t648 = t126.*(3.0./2.0e+2);
t650 = t127.*(3.0./2.0e+2);
t651 = t128.*(3.0./2.0e+2);
t653 = t130.*(3.0./2.0e+2);
t654 = t123.*(3.0./4.0e+2);
t655 = t124.*(3.0./4.0e+2);
t656 = -t503;
t657 = t9.*t348;
t658 = t85.*(2.7e+1./1.0e+2);
t660 = t9.*t350;
t661 = t87.*(9.0./2.0e+2);
t669 = t9.*t356;
t674 = t20.*t177;
t676 = t12.*t357;
t678 = t9.*t358;
t687 = t48+t82;
t688 = t59+t100;
t689 = t49+t85;
t690 = t60+t107;
t699 = -t532;
t700 = -t533;
t706 = t189./1.0e+1;
t711 = t51.*t160;
t713 = t51.*t161;
t716 = t48.*t169;
t717 = t52.*t160;
t719 = t48.*t171;
t721 = t192./1.0e+1;
t722 = t3.*t408;
t723 = (t6.*t100)./1.0e+1;
t725 = t48.*t172;
t726 = t52.*t161;
t729 = t48.*t173;
t737 = t51.*t168;
t738 = (t8.*t99)./1.0e+1;
t742 = t51.*t169;
t744 = t58.*t160;
t748 = t8.*t99.*(3.0./1.0e+1);
t750 = t51.*t172;
t751 = t58.*t161;
t754 = t11.*t98.*(3.0./2.5e+1);
t756 = t11.*t99.*(6.0./2.5e+1);
t758 = t54.*t164;
t759 = t195.*(3.0./5.0e+1);
t761 = t11.*t390;
t763 = t198.*(-2.0./5.0);
t766 = t48.*t180;
t767 = t198.*(-6.0./5.0);
t768 = t52.*t171;
t769 = t53.*t169;
t770 = t59.*t160;
t773 = t3.*t460;
t774 = (t12.*t100)./1.0e+1;
t775 = (t6.*t115)./1.0e+1;
t776 = t201./1.0e+1;
t781 = t48.*t181;
t782 = t52.*t173;
t784 = t53.*t172;
t785 = t59.*t161;
t788 = t93.*t106;
t796 = t58.*t168;
t798 = t51.*t179;
t799 = (t8.*t114)./1.0e+1;
t800 = t5.*t468;
t803 = t57.*t169;
t805 = t62.*t160;
t807 = t58.*t169;
t808 = t51.*t180;
t809 = t58.*t171;
t814 = t8.*t114.*(3.0./1.0e+1);
t815 = t5.*t482;
t816 = t57.*t172;
t817 = t62.*t161;
t819 = t51.*t181;
t820 = t58.*t173;
t821 = t202.*(3.0./2.5e+1);
t822 = t203.*(3.0./2.5e+1);
t823 = t62.*t162;
t824 = t11.*t112.*(6.0./2.5e+1);
t826 = t203.*(3.0./5.0e+1);
t831 = t12.*t114.*(3.0./5.0e+1);
t832 = t12.*t443;
t833 = t12.*t444;
t837 = t97.*(9.0./2.0e+2);
t838 = t98.*(9.0./2.0e+2);
t839 = t99.*(9.0./2.0e+2);
t842 = t209.*(-2.0./5.0);
t844 = t52.*t180;
t847 = t53.*t180;
t848 = t209.*(-6.0./5.0);
t849 = t59.*t171;
t850 = (t12.*t115)./1.0e+1;
t851 = t3.*t318;
t852 = (t12.*t116)./1.0e+1;
t853 = t9.*t468;
t854 = t52.*t181;
t858 = t53.*t181;
t859 = t59.*t173;
t867 = t58.*t179;
t868 = (t8.*t130)./1.0e+1;
t871 = t62.*t169;
t872 = (t9.*t129)./1.0e+1;
t875 = t58.*t180;
t879 = t8.*t130.*(3.0./1.0e+1);
t880 = t62.*t172;
t883 = t58.*t181;
t884 = t9.*t125.*(3.0./2.5e+1);
t885 = t210.*(3.0./2.5e+1);
t886 = t9.*t129.*(3.0./2.5e+1);
t890 = t210.*(3.0./4.0e+1);
t891 = t211.*(3.0./5.0e+1);
t895 = t108.*(9.0./1.0e+2);
t896 = t114.*(9.0./1.0e+2);
t898 = t107.*(2.7e+1./1.0e+2);
t906 = t108.*(9.0./2.0e+2);
t907 = t109.*(9.0./2.0e+2);
t908 = t110.*(9.0./2.0e+2);
t910 = t112.*(9.0./2.0e+2);
t911 = t114.*(9.0./2.0e+2);
t912 = t5.*t342;
t914 = t9.*t313;
t918 = -t615;
t919 = t59.*t180;
t920 = (t12.*t82)./1.0e+1;
t921 = t59.*t181;
t923 = t12.*t82.*(3.0./1.0e+1);
t926 = t62.*t180;
t928 = t62.*t181;
t929 = t215.*(3.0./2.5e+1);
t930 = t215.*(3.0./5.0e+1);
t934 = t125.*(9.0./1.0e+2);
t935 = t126.*(9.0./1.0e+2);
t937 = t123.*(2.7e+1./1.0e+2);
t938 = t9.*t333;
t944 = t9.*t339;
t945 = t125.*(9.0./2.0e+2);
t946 = t126.*(9.0./2.0e+2);
t947 = t9.*t342;
t948 = t128.*(9.0./2.0e+2);
tau = ft_3({dq1,dq2,dq3,dq4,dq5,dq6,t10,t100,t1001,t1005,t1009,t101,t1018,t102,t1022,t103,t1031,t104,t1040,t1041,t105,t106,t107,t1073,t1076,t1077,t1078,t108,t109,t1095,t1096,t1098,t11,t110,t111,t1110,t1114,t112,t1123,t1125,t113,t1131,t1132,t1134,t114,t115,t1158,t116,t1160,t1162,t1163,t1169,t117,t1170,t1171,t1172,t1173,t1175,t118,t1180,t1184,t1186,t1189,t119,t1191,t1196,t1197,t1198,t1199,t12,t120,t1200,t1201,t1204,t1205,t1207,t1208,t121,t1211,t1214,t1219,t122,t1220,t1221,t1222,t1223,t1224,t1225,t1228,t1229,t123,t1230,t1231,t1233,t1234,t1236,t1237,t1238,t1239,t124,t1240,t1242,t1246,t1247,t125,t126,t1266,t127,t128,t129,t1294,t1295,t1297,t1298,t13,t130,t131,t132,t1322,t1323,t133,t1347,t1348,t135,t1357,t1361,t1362,t1363,t1366,t137,t138,t1384,t1385,t139,t1397,t1398,t140,t141,t1413,t142,t1427,t1429,t143,t1434,t1438,t144,t145,t1450,t1456,t1457,t1458,t146,t1462,t1464,t1465,t1467,t147,t1473,t1474,t1475,t1476,t1477,t1478,t1479,t148,t1480,t1481,t1485,t1486,t1487,t1488,t1489,t149,t1490,t1493,t1494,t1497,t150,t1502,t151,t152,t1528,t153,t1532,t1538,t154,t155,t1557,t1558,t158,t1581,t1582,t159,t1597,t1598,t1599,t160,t161,t1617,t1618,t1619,t162,t1620,t1621,t1622,t163,t1638,t164,t1643,t165,t1651,t166,t1660,t167,t168,t1684,t1685,t1689,t1696,t170,t1702,t171,t1713,t1719,t1720,t1726,t173,t1730,t1732,t1733,t1740,t1741,t1747,t1748,t1756,t1757,t1760,t177,t1772,t1773,t1774,t1776,t178,t1785,t179,t18,t180,t1801,t1803,t1804,t1805,t1806,t1808,t181,t182,t1822,t1823,t1828,t183,t1831,t1832,t1839,t184,t1840,t1845,t1849,t185,t1852,t1853,t1858,t186,t1861,t1866,t1867,t1869,t187,t1870,t1872,t1873,t1876,t1877,t1878,t188,t1880,t1881,t1884,t1886,t1887,t1888,t189,t1890,t1891,t1893,t1897,t1899,t19,t190,t191,t1917,t1919,t192,t1925,t1926,t1927,t193,t194,t1944,t1947,t1948,t1949,t195,t1950,t1951,t196,t1962,t1963,t1967,t1968,t1969,t197,t1978,t1979,t198,t1983,t1989,t199,t1999,t2,t20,t200,t2001,t2002,t2008,t201,t2014,t202,t2023,t2024,t2025,t203,t2030,t2031,t2034,t2035,t2036,t2037,t204,t2046,t2052,t2053,t2055,t2056,t2058,t206,t2061,t2063,t2064,t2065,t2066,t207,t2070,t2071,t2072,t2076,t2078,t208,t2085,t2086,t209,t2091,t2092,t2094,t2096,t2097,t21,t210,t211,t2111,t2112,t212,t2124,t2125,t2126,t213,t2136,t2137,t214,t2141,t2142,t2143,t2145,t2146,t215,t2153,t2154,t2155,t216,t2163,t2164,t2166,t2167,t217,t2170,t2174,t2176,t218,t219,t2192,t2193,t22,t220,t221,t2212,t2213,t2214,t2215,t2218,t222,t2221,t2222,t2223,t2224,t2225,t2226,t223,t2231,t2232,t2233,t2235,t224,t2240,t2241,t225,t2250,t226,t227,t2277,t2278,t228,t229,t230,t2309,t231,t2316,t2317,t2321,t2323,t2324,t2327,t2328,t233,t2331,t2334,t234,t2343,t235,t2357,t236,t2361,t2362,t2366,t2369,t237,t2371,t2372,t2378,t2379,t238,t2382,t2383,t2387,t2389,t239,t2391,t2395,t2398,t240,t2402,t2409,t241,t2412,t2419,t242,t2423,t2425,t2429,t243,t2430,t2431,t2432,t2433,t244,t245,t2450,t2451,t2453,t2454,t246,t2466,t2467,t247,t2473,t2478,t248,t249,t2494,t2495,t2496,t25,t250,t251,t2519,t252,t2520,t2526,t253,t254,t2540,t2541,t2546,t255,t2556,t2557,t256,t2560,t2561,t2566,t2567,t2568,t2569,t2570,t2571,t2572,t258,t2580,t2581,t2583,t2585,t2586,t2588,t2589,t259,t2590,t2591,t2593,t2595,t2597,t2598,t2599,t26,t260,t2600,t2601,t2602,t2603,t2607,t2608,t2609,t261,t2610,t2611,t2614,t2615,t262,t263,t2632,t2633,t2634,t2635,t2636,t2637,t2639,t2646,t265,t267,t2672,t2684,t2686,t269,t27,t270,t2708,t272,t2725,t2726,t2727,t2729,t273,t2730,t2731,t2732,t2733,t2735,t2738,t274,t2740,t2741,t2742,t2746,t2749,t275,t276,t2762,t2765,t2769,t277,t2771,t2779,t278,t2780,t2785,t2786,t2788,t279,t2791,t2792,t2793,t28,t280,t281,t2822,t2823,t2824,t2825,t283,t284,t285,t2854,t286,t2867,t2868,t2869,t287,t288,t289,t2899,t29,t290,t2900,t2902,t292,t293,t2933,t2935,t2939,t294,t2942,t2948,t295,t2951,t2952,t2953,t296,t2961,t2967,t2968,t297,t2974,t2975,t2977,t2978,t2979,t298,t299,t3,t30,t300,t3002,t301,t3010,t3011,t3013,t3015,t3016,t3017,t302,t3020,t3021,t3023,t303,t3034,t304,t3047,t3049,t305,t3052,t3054,t3056,t3058,t306,t3067,t307,t3075,t3077,t3078,t308,t309,t3099,t31,t3101,t3102,t3109,t311,t3118,t312,t313,t3138,t3139,t314,t3143,t315,t316,t317,t318,t319,t3192,t32,t320,t3204,t3206,t3208,t321,t3210,t3211,t3212,t3213,t3214,t3216,t3217,t322,t323,t3231,t324,t3245,t3246,t325,t326,t3262,t327,t3272,t328,t329,t3298,t3299,t33,t330,t331,t332,t3320,t3326,t333,t3330,t334,t336,t337,t338,t3388,t339,t3396,t34,t341,t342,t343,t344,t345,t3453,t346,t347,t3470,t3471,t3473,t3479,t348,t3480,t3483,t3484,t3485,t3486,t349,t3490,t3491,t3497,t3498,t35,t350,t3501,t3510,t3511,t352,t3521,t3526,t3527,t3528,t3529,t353,t354,t3546,t3547,t3549,t355,t3551,t3559,t356,t3560,t3562,t357,t358,t3589,t3590,t3592,t3593,t3594,t3595,t360,t3608,t3609,t3611,t3612,t3613,t3614,t3615,t3616,t3617,t3627,t3628,t3629,t3630,t3635,t3636,t3637,t364,t3648,t365,t3650,t3651,t367,t368,t3680,t3687,t3690,t3691,t3692,t3704,t3705,t371,t3722,t3723,t3724,t3725,t3726,t373,t375,t376,t377,t3779,t378,t379,t3796,t380,t381,t3811,t382,t3822,t3823,t3824,t3827,t3828,t383,t3839,t384,t385,t386,t3862,t3865,t3868,t387,t3871,t3872,t388,t3884,t389,t390,t3909,t391,t3910,t392,t3932,t3935,t3941,t396,t3960,t3963,t397,t399,t4,t400,t401,t402,t4031,t404,t4042,t4043,t4046,t4047,t405,t4057,t406,t4060,t4061,t4067,t407,t4075,t408,t409,t410,t4103,t4109,t411,t412,t413,t414,t415,t416,t4168,t417,t4174,t418,t419,t420,t4204,t4208,t4209,t421,t4212,t422,t423,t424,t425,t426,t4260,t4261,t4262,t4263,t4265,t427,t4280,t429,t430,t431,t432,t433,t434,t4344,t4345,t4347,t435,t436,t437,t4372,t438,t439,t440,t441,t442,t443,t444,t4451,t4452,t4456,t4457,t4475,t4477,t4478,t450,t4508,t451,t453,t4539,t454,t4542,t4544,t4545,t4546,t4547,t456,t4565,t4566,t4568,t4579,t458,t4581,t4584,t459,t460,t461,t462,t463,t464,t465,t467,t468,t469,t470,t471,t472,t473,t474,t475,t476,t4763,t4765,t4766,t4768,t4769,t477,t4770,t4771,t4773,t478,t479,t48,t480,t4806,t4808,t481,t482,t483,t4830,t4831,t4833,t484,t486,t487,t488,t489,t4895,t4898,t49,t490,t4900,t491,t492,t494,t495,t496,t497,t498,t499,t5,t50,t500,t501,t502,t5041,t5054,t5055,t509,t51,t510,t5103,t511,t512,t513,t514,t515,t516,t517,t5175,t5176,t518,t519,t52,t520,t521,t522,t523,t524,t525,t526,t527,t528,t5280,t529,t53,t530,t531,t533,t534,t5343,t5344,t535,t5354,t5356,t536,t5361,t539,t54,t540,t5411,t542,t543,t545,t546,t547,t548,t5491,t5492,t55,t550,t551,t552,t553,t5551,t5552,t556,t557,t558,t559,t56,t560,t561,t5613,t562,t563,t565,t566,t567,t569,t57,t574,t58,t582,t585,t589,t59,t590,t592,t594,t595,t597,t598,t599,t6,t60,t600,t601,t602,t6023,t603,t604,t605,t606,t608,t609,t61,t610,t611,t613,t614,t616,t617,t62,t624,t63,t630,t632,t635,t636,t641,t643,t644,t645,t647,t6473,t648,t649,t650,t651,t652,t653,t654,t655,t656,t657,t658,t66,t660,t661,t663,t664,t665,t666,t667,t668,t669,t67,t670,t671,t672,t673,t6734,t6735,t6736,t674,t6742,t6743,t6744,t6745,t675,t6754,t6755,t676,t677,t6772,t678,t679,t680,t681,t682,t683,t684,t685,t686,t687,t688,t689,t690,t691,t692,t693,t695,t696,t697,t698,t699,t7,t700,t701,t702,t703,t704,t705,t706,t708,t711,t713,t715,t716,t717,t719,t720,t721,t722,t723,t725,t726,t729,t731,t732,t734,t737,t738,t742,t744,t748,t750,t751,t753,t754,t755,t756,t758,t759,t761,t762,t763,t766,t767,t768,t769,t770,t773,t774,t775,t776,t781,t782,t784,t785,t788,t789,t790,t793,t795,t796,t798,t799,t8,t800,t803,t805,t807,t808,t809,t81,t814,t815,t816,t817,t819,t82,t820,t821,t822,t823,t824,t826,t828,t829,t83,t831,t832,t833,t834,t835,t837,t838,t839,t84,t842,t844,t847,t848,t849,t85,t850,t851,t852,t853,t854,t858,t859,t86,t861,t863,t864,t867,t868,t87,t871,t872,t875,t879,t88,t880,t883,t884,t885,t886,t887,t888,t89,t890,t891,t894,t895,t896,t897,t898,t899,t9,t90,t900,t902,t905,t906,t907,t908,t909,t910,t911,t912,t913,t914,t915,t916,t918,t919,t92,t920,t921,t923,t926,t928,t929,t93,t930,t931,t933,t934,t935,t936,t937,t938,t939,t944,t945,t946,t947,t948,t95,t954,t955,t956,t957,t958,t959,t96,t960,t961,t962,t963,t964,t966,t967,t968,t97,t971,t973,t979,t98,t982,t983,t984,t988,t99,t992,t993,t997,t998,t999});
end
function tau = ft_3(ct)
[dq1,dq2,dq3,dq4,dq5,dq6,t10,t100,t1001,t1005,t1009,t101,t1018,t102,t1022,t103,t1031,t104,t1040,t1041,t105,t106,t107,t1073,t1076,t1077,t1078,t108,t109,t1095,t1096,t1098,t11,t110,t111,t1110,t1114,t112,t1123,t1125,t113,t1131,t1132,t1134,t114,t115,t1158,t116,t1160,t1162,t1163,t1169,t117,t1170,t1171,t1172,t1173,t1175,t118,t1180,t1184,t1186,t1189,t119,t1191,t1196,t1197,t1198,t1199,t12,t120,t1200,t1201,t1204,t1205,t1207,t1208,t121,t1211,t1214,t1219,t122,t1220,t1221,t1222,t1223,t1224,t1225,t1228,t1229,t123,t1230,t1231,t1233,t1234,t1236,t1237,t1238,t1239,t124,t1240,t1242,t1246,t1247,t125,t126,t1266,t127,t128,t129,t1294,t1295,t1297,t1298,t13,t130,t131,t132,t1322,t1323,t133,t1347,t1348,t135,t1357,t1361,t1362,t1363,t1366,t137,t138,t1384,t1385,t139,t1397,t1398,t140,t141,t1413,t142,t1427,t1429,t143,t1434,t1438,t144,t145,t1450,t1456,t1457,t1458,t146,t1462,t1464,t1465,t1467,t147,t1473,t1474,t1475,t1476,t1477,t1478,t1479,t148,t1480,t1481,t1485,t1486,t1487,t1488,t1489,t149,t1490,t1493,t1494,t1497,t150,t1502,t151,t152,t1528,t153,t1532,t1538,t154,t155,t1557,t1558,t158,t1581,t1582,t159,t1597,t1598,t1599,t160,t161,t1617,t1618,t1619,t162,t1620,t1621,t1622,t163,t1638,t164,t1643,t165,t1651,t166,t1660,t167,t168,t1684,t1685,t1689,t1696,t170,t1702,t171,t1713,t1719,t1720,t1726,t173,t1730,t1732,t1733,t1740,t1741,t1747,t1748,t1756,t1757,t1760,t177,t1772,t1773,t1774,t1776,t178,t1785,t179,t18,t180,t1801,t1803,t1804,t1805,t1806,t1808,t181,t182,t1822,t1823,t1828,t183,t1831,t1832,t1839,t184,t1840,t1845,t1849,t185,t1852,t1853,t1858,t186,t1861,t1866,t1867,t1869,t187,t1870,t1872,t1873,t1876,t1877,t1878,t188,t1880,t1881,t1884,t1886,t1887,t1888,t189,t1890,t1891,t1893,t1897,t1899,t19,t190,t191,t1917,t1919,t192,t1925,t1926,t1927,t193,t194,t1944,t1947,t1948,t1949,t195,t1950,t1951,t196,t1962,t1963,t1967,t1968,t1969,t197,t1978,t1979,t198,t1983,t1989,t199,t1999,t2,t20,t200,t2001,t2002,t2008,t201,t2014,t202,t2023,t2024,t2025,t203,t2030,t2031,t2034,t2035,t2036,t2037,t204,t2046,t2052,t2053,t2055,t2056,t2058,t206,t2061,t2063,t2064,t2065,t2066,t207,t2070,t2071,t2072,t2076,t2078,t208,t2085,t2086,t209,t2091,t2092,t2094,t2096,t2097,t21,t210,t211,t2111,t2112,t212,t2124,t2125,t2126,t213,t2136,t2137,t214,t2141,t2142,t2143,t2145,t2146,t215,t2153,t2154,t2155,t216,t2163,t2164,t2166,t2167,t217,t2170,t2174,t2176,t218,t219,t2192,t2193,t22,t220,t221,t2212,t2213,t2214,t2215,t2218,t222,t2221,t2222,t2223,t2224,t2225,t2226,t223,t2231,t2232,t2233,t2235,t224,t2240,t2241,t225,t2250,t226,t227,t2277,t2278,t228,t229,t230,t2309,t231,t2316,t2317,t2321,t2323,t2324,t2327,t2328,t233,t2331,t2334,t234,t2343,t235,t2357,t236,t2361,t2362,t2366,t2369,t237,t2371,t2372,t2378,t2379,t238,t2382,t2383,t2387,t2389,t239,t2391,t2395,t2398,t240,t2402,t2409,t241,t2412,t2419,t242,t2423,t2425,t2429,t243,t2430,t2431,t2432,t2433,t244,t245,t2450,t2451,t2453,t2454,t246,t2466,t2467,t247,t2473,t2478,t248,t249,t2494,t2495,t2496,t25,t250,t251,t2519,t252,t2520,t2526,t253,t254,t2540,t2541,t2546,t255,t2556,t2557,t256,t2560,t2561,t2566,t2567,t2568,t2569,t2570,t2571,t2572,t258,t2580,t2581,t2583,t2585,t2586,t2588,t2589,t259,t2590,t2591,t2593,t2595,t2597,t2598,t2599,t26,t260,t2600,t2601,t2602,t2603,t2607,t2608,t2609,t261,t2610,t2611,t2614,t2615,t262,t263,t2632,t2633,t2634,t2635,t2636,t2637,t2639,t2646,t265,t267,t2672,t2684,t2686,t269,t27,t270,t2708,t272,t2725,t2726,t2727,t2729,t273,t2730,t2731,t2732,t2733,t2735,t2738,t274,t2740,t2741,t2742,t2746,t2749,t275,t276,t2762,t2765,t2769,t277,t2771,t2779,t278,t2780,t2785,t2786,t2788,t279,t2791,t2792,t2793,t28,t280,t281,t2822,t2823,t2824,t2825,t283,t284,t285,t2854,t286,t2867,t2868,t2869,t287,t288,t289,t2899,t29,t290,t2900,t2902,t292,t293,t2933,t2935,t2939,t294,t2942,t2948,t295,t2951,t2952,t2953,t296,t2961,t2967,t2968,t297,t2974,t2975,t2977,t2978,t2979,t298,t299,t3,t30,t300,t3002,t301,t3010,t3011,t3013,t3015,t3016,t3017,t302,t3020,t3021,t3023,t303,t3034,t304,t3047,t3049,t305,t3052,t3054,t3056,t3058,t306,t3067,t307,t3075,t3077,t3078,t308,t309,t3099,t31,t3101,t3102,t3109,t311,t3118,t312,t313,t3138,t3139,t314,t3143,t315,t316,t317,t318,t319,t3192,t32,t320,t3204,t3206,t3208,t321,t3210,t3211,t3212,t3213,t3214,t3216,t3217,t322,t323,t3231,t324,t3245,t3246,t325,t326,t3262,t327,t3272,t328,t329,t3298,t3299,t33,t330,t331,t332,t3320,t3326,t333,t3330,t334,t336,t337,t338,t3388,t339,t3396,t34,t341,t342,t343,t344,t345,t3453,t346,t347,t3470,t3471,t3473,t3479,t348,t3480,t3483,t3484,t3485,t3486,t349,t3490,t3491,t3497,t3498,t35,t350,t3501,t3510,t3511,t352,t3521,t3526,t3527,t3528,t3529,t353,t354,t3546,t3547,t3549,t355,t3551,t3559,t356,t3560,t3562,t357,t358,t3589,t3590,t3592,t3593,t3594,t3595,t360,t3608,t3609,t3611,t3612,t3613,t3614,t3615,t3616,t3617,t3627,t3628,t3629,t3630,t3635,t3636,t3637,t364,t3648,t365,t3650,t3651,t367,t368,t3680,t3687,t3690,t3691,t3692,t3704,t3705,t371,t3722,t3723,t3724,t3725,t3726,t373,t375,t376,t377,t3779,t378,t379,t3796,t380,t381,t3811,t382,t3822,t3823,t3824,t3827,t3828,t383,t3839,t384,t385,t386,t3862,t3865,t3868,t387,t3871,t3872,t388,t3884,t389,t390,t3909,t391,t3910,t392,t3932,t3935,t3941,t396,t3960,t3963,t397,t399,t4,t400,t401,t402,t4031,t404,t4042,t4043,t4046,t4047,t405,t4057,t406,t4060,t4061,t4067,t407,t4075,t408,t409,t410,t4103,t4109,t411,t412,t413,t414,t415,t416,t4168,t417,t4174,t418,t419,t420,t4204,t4208,t4209,t421,t4212,t422,t423,t424,t425,t426,t4260,t4261,t4262,t4263,t4265,t427,t4280,t429,t430,t431,t432,t433,t434,t4344,t4345,t4347,t435,t436,t437,t4372,t438,t439,t440,t441,t442,t443,t444,t4451,t4452,t4456,t4457,t4475,t4477,t4478,t450,t4508,t451,t453,t4539,t454,t4542,t4544,t4545,t4546,t4547,t456,t4565,t4566,t4568,t4579,t458,t4581,t4584,t459,t460,t461,t462,t463,t464,t465,t467,t468,t469,t470,t471,t472,t473,t474,t475,t476,t4763,t4765,t4766,t4768,t4769,t477,t4770,t4771,t4773,t478,t479,t48,t480,t4806,t4808,t481,t482,t483,t4830,t4831,t4833,t484,t486,t487,t488,t489,t4895,t4898,t49,t490,t4900,t491,t492,t494,t495,t496,t497,t498,t499,t5,t50,t500,t501,t502,t5041,t5054,t5055,t509,t51,t510,t5103,t511,t512,t513,t514,t515,t516,t517,t5175,t5176,t518,t519,t52,t520,t521,t522,t523,t524,t525,t526,t527,t528,t5280,t529,t53,t530,t531,t533,t534,t5343,t5344,t535,t5354,t5356,t536,t5361,t539,t54,t540,t5411,t542,t543,t545,t546,t547,t548,t5491,t5492,t55,t550,t551,t552,t553,t5551,t5552,t556,t557,t558,t559,t56,t560,t561,t5613,t562,t563,t565,t566,t567,t569,t57,t574,t58,t582,t585,t589,t59,t590,t592,t594,t595,t597,t598,t599,t6,t60,t600,t601,t602,t6023,t603,t604,t605,t606,t608,t609,t61,t610,t611,t613,t614,t616,t617,t62,t624,t63,t630,t632,t635,t636,t641,t643,t644,t645,t647,t6473,t648,t649,t650,t651,t652,t653,t654,t655,t656,t657,t658,t66,t660,t661,t663,t664,t665,t666,t667,t668,t669,t67,t670,t671,t672,t673,t6734,t6735,t6736,t674,t6742,t6743,t6744,t6745,t675,t6754,t6755,t676,t677,t6772,t678,t679,t680,t681,t682,t683,t684,t685,t686,t687,t688,t689,t690,t691,t692,t693,t695,t696,t697,t698,t699,t7,t700,t701,t702,t703,t704,t705,t706,t708,t711,t713,t715,t716,t717,t719,t720,t721,t722,t723,t725,t726,t729,t731,t732,t734,t737,t738,t742,t744,t748,t750,t751,t753,t754,t755,t756,t758,t759,t761,t762,t763,t766,t767,t768,t769,t770,t773,t774,t775,t776,t781,t782,t784,t785,t788,t789,t790,t793,t795,t796,t798,t799,t8,t800,t803,t805,t807,t808,t809,t81,t814,t815,t816,t817,t819,t82,t820,t821,t822,t823,t824,t826,t828,t829,t83,t831,t832,t833,t834,t835,t837,t838,t839,t84,t842,t844,t847,t848,t849,t85,t850,t851,t852,t853,t854,t858,t859,t86,t861,t863,t864,t867,t868,t87,t871,t872,t875,t879,t88,t880,t883,t884,t885,t886,t887,t888,t89,t890,t891,t894,t895,t896,t897,t898,t899,t9,t90,t900,t902,t905,t906,t907,t908,t909,t910,t911,t912,t913,t914,t915,t916,t918,t919,t92,t920,t921,t923,t926,t928,t929,t93,t930,t931,t933,t934,t935,t936,t937,t938,t939,t944,t945,t946,t947,t948,t95,t954,t955,t956,t957,t958,t959,t96,t960,t961,t962,t963,t964,t966,t967,t968,t97,t971,t973,t979,t98,t982,t983,t984,t988,t99,t992,t993,t997,t998,t999] = ct{:};
t949 = t129.*(9.0./2.0e+2);
t950 = t5.*t350;
t951 = t130.*(9.0./2.0e+2);
t965 = -t665;
t969 = t20.*t230;
t970 = t19.*t233;
t972 = -t668;
t974 = -t670;
t975 = -t671;
t976 = -t672;
t977 = -t673;
t978 = t9.*t524;
t981 = t27.*t230;
t986 = t20.*t251;
t987 = t19.*t254;
t990 = t20.*t260;
t991 = t11.*t529;
t994 = t27.*t251;
t996 = -t682;
t1002 = -t695;
t1003 = -t697;
t1004 = -t698;
t1006 = sqrt(t258);
t1007 = -t701;
t1010 = t49.*t231;
t1011 = t12.*t95.*(-1.0./1.0e+1);
t1013 = t12.*t96.*(-1.0./1.0e+1);
t1016 = t12.*t95.*(-3.0./1.0e+1);
t1019 = t12.*t96.*(-3.0./1.0e+1);
t1023 = -t753;
t1025 = -t755;
t1027 = t10.*t97.*(-3.0./5.0e+1);
t1029 = t12.*t97.*(-3.0./5.0e+1);
t1030 = t9.*t98.*(9.0./5.0e+1);
t1033 = t49.*t251;
t1034 = t194.*(3.0./2.0e+2);
t1035 = t195.*(3.0./2.0e+2);
t1037 = t50.*t252;
t1039 = -t762;
t1042 = t196.*(-1.0./1.0e+1);
t1043 = t197.*(-1.0./1.0e+1);
t1047 = t196.*(-3.0./1.0e+1);
t1048 = t197.*(-3.0./1.0e+1);
t1050 = t12.*t103.*(-1.0./1.0e+1);
t1051 = t6.*t118.*(-1.0./1.0e+1);
t1053 = t12.*t104.*(-1.0./1.0e+1);
t1055 = t6.*t115.*(-3.0./1.0e+1);
t1056 = t6.*t120.*(-1.0./1.0e+1);
t1058 = t202.*(-1.0./1.0e+1);
t1059 = t12.*t103.*(-3.0./1.0e+1);
t1060 = t203.*(-1.0./1.0e+1);
t1061 = t6.*t118.*(-3.0./1.0e+1);
t1062 = t204.*(-1.0./1.0e+1);
t1063 = t12.*t104.*(-3.0./1.0e+1);
t1065 = t6.*t120.*(-3.0./1.0e+1);
t1067 = t203.*(-3.0./1.0e+1);
t1068 = t204.*(-3.0./1.0e+1);
t1072 = t11.*t112.*(-3.0./5.0e+1);
t1074 = t12.*t112.*(-3.0./5.0e+1);
t1080 = t202.*(3.0./1.0e+2);
t1081 = t203.*(3.0./1.0e+2);
t1082 = t9.*t113.*(3.0./1.0e+2);
t1083 = t109.*t143;
t1084 = t50.*t261;
t1085 = t110.*t143;
t1086 = t61.*t230;
t1087 = t11.*t113.*(3.0./1.0e+2);
t1088 = t4.*t123.*(3.0./2.0e+2);
t1089 = t202.*(3.0./2.0e+2);
t1090 = t203.*(3.0./2.0e+2);
t1091 = t204.*(3.0./2.0e+2);
t1092 = t55.*t252;
t1099 = t206.*(-1.0./1.0e+1);
t1100 = t207.*(-1.0./1.0e+1);
t1101 = t206.*(-3.0./1.0e+1);
t1102 = t2.*t86.*(-1.0./1.0e+1);
t1103 = t207.*(-3.0./1.0e+1);
t1104 = t12.*t118.*(-1.0./1.0e+1);
t1105 = t12.*t121.*(-1.0./1.0e+1);
t1106 = t12.*t122.*(-1.0./1.0e+1);
t1107 = t2.*t86.*(-3.0./1.0e+1);
t1108 = t12.*t118.*(-3.0./1.0e+1);
t1111 = t12.*t121.*(-3.0./1.0e+1);
t1112 = t12.*t122.*(-3.0./1.0e+1);
t1113 = t9.*t129.*(-3.0./1.0e+1);
t1116 = -t887;
t1117 = t11.*t127.*(-3.0./2.5e+1);
t1119 = t210.*(3.0./1.0e+2);
t1120 = t55.*t261;
t1122 = t210.*(3.0./2.0e+2);
t1124 = t211.*(3.0./2.0e+2);
t1127 = -t900;
t1133 = -t915;
t1135 = t107.*(1.17e+2./2.0e+2);
t1141 = t12.*t83.*(-1.0./1.0e+1);
t1144 = t12.*t83.*(-3.0./1.0e+1);
t1145 = t215.*(-1.0./1.0e+1);
t1147 = t215.*(-3.0./1.0e+1);
t1148 = t215.*(3.0./1.0e+2);
t1149 = t215.*(3.0./2.0e+2);
t1151 = -t939;
t1159 = t123.*(1.17e+2./2.0e+2);
t1161 = t124.*(1.17e+2./2.0e+2);
t1164 = -t954;
t1165 = t86.*1.35e-3;
t1166 = t19.*t98.*(3.0./2.5e+1);
t1167 = t20.*t97.*(6.0./2.5e+1);
t1176 = t19.*t111.*(6.0./2.5e+1);
t1177 = t20.*t109.*(6.0./2.5e+1);
t1178 = t20.*t110.*(6.0./2.5e+1);
t1182 = t4.*t672;
t1183 = t21.*t107.*(3.0./5.0e+1);
t1188 = t19.*t444;
t1190 = -t963;
t1192 = t19.*t491;
t1193 = t20.*t125.*(3.0./2.5e+1);
t1194 = t20.*t126.*(3.0./2.5e+1);
t1195 = t18.*t129.*(3.0./2.5e+1);
t1202 = t21.*t123.*(3.0./5.0e+1);
t1203 = t21.*t124.*(3.0./5.0e+1);
t1210 = t18.*t311;
t1212 = t20.*t311;
t1215 = -t971;
t1216 = t25.*t129.*(3.0./2.5e+1);
t1217 = t21.*t85.*(3.0./5.0e+1);
t1218 = -t979;
t1227 = -t982;
t1235 = -t992;
t1241 = t18.*t350;
t1243 = t9.*t696;
t1244 = -t998;
t1245 = -t999;
t1254 = -t1005;
t1255 = t346.*9.6e+1;
t1256 = -t1009;
t1263 = t49.*t114.*(3.0./5.0e+1);
t1283 = t49.*t126.*(3.0./2.5e+1);
t1286 = t57.*t107.*(6.0./2.5e+1);
t1287 = t49.*t130.*(6.0./2.5e+1);
t1288 = t60.*t99.*(6.0./2.5e+1);
t1289 = t50.*t130.*(6.0./2.5e+1);
t1291 = t60.*t390;
t1293 = t19.*t358;
t1296 = t11.*t762;
t1299 = t49.*t311;
t1316 = t87.*t162;
t1317 = t123.*t178;
t1319 = t12.*t204.*(3.0./5.0e+1);
t1320 = t58.*t127.*(3.0./5.0e+1);
t1324 = -t1031;
t1325 = t9.*t97.*(9.0./1.0e+2);
t1326 = t194.*(9.0./1.0e+2);
t1327 = t195.*(9.0./1.0e+2);
t1328 = t9.*t99.*(9.0./1.0e+2);
t1329 = t10.*t97.*(-3.0./2.0e+2);
t1331 = t9.*t99.*(-3.0./2.0e+2);
t1332 = t11.*t99.*(-3.0./2.0e+2);
t1333 = t49.*t341;
t1334 = t194.*(9.0./2.0e+2);
t1335 = t195.*(9.0./2.0e+2);
t1345 = -t1040;
t1346 = -t1041;
t1349 = t10.*t108.*(-3.0./1.0e+2);
t1352 = t12.*t109.*(-3.0./1.0e+2);
t1353 = t12.*t110.*(-3.0./1.0e+2);
t1355 = t9.*t111.*(9.0./1.0e+2);
t1356 = t204.*(9.0./1.0e+2);
t1358 = t11.*t113.*(9.0./1.0e+2);
t1359 = t9.*t897;
t1369 = t202.*(9.0./2.0e+2);
t1370 = t203.*(9.0./2.0e+2);
t1371 = t204.*(9.0./2.0e+2);
t1372 = t9.*t113.*(9.0./2.0e+2);
t1373 = t60.*t311;
t1375 = t11.*t111.*(9.0./2.0e+2);
t1376 = t50.*t350;
t1377 = t61.*t311;
t1379 = t9.*t916;
t1380 = t9.*t107.*(-3.0./4.0e+2);
t1383 = -t1096;
t1386 = -t1098;
t1387 = t97.*1.35e-3;
t1388 = t11.*t127.*(-3.0./1.0e+2);
t1390 = t211.*(9.0./1.0e+2);
t1391 = t11.*t127.*(9.0./1.0e+2);
t1392 = -t1125;
t1393 = t210.*(9.0./2.0e+2);
t1395 = t211.*(9.0./2.0e+2);
t1399 = t108.*1.35e-3;
t1400 = t109.*1.35e-3;
t1401 = t110.*1.35e-3;
t1402 = t111.*1.35e-3;
t1403 = t112.*1.35e-3;
t1404 = t215.*(9.0./2.0e+2);
t1406 = -t1162;
t1407 = t127.*1.35e-3;
t1408 = t83.*1.0675e-2;
t1409 = t86.*2.98828125e-3;
t1410 = t87.*2.98828125e-3;
t1416 = -t1170;
t1417 = -t1172;
t1419 = -t1175;
t1423 = -t1180;
t1424 = t18.*t597;
t1426 = -t1184;
t1432 = t18.*t113.*(3.0./1.0e+2);
t1433 = t3.*t6.*t531;
t1435 = t51.*t531;
t1441 = -t1197;
t1442 = -t1199;
t1443 = -t1200;
t1445 = t18.*t643;
t1447 = t25.*t113.*(3.0./1.0e+2);
t1452 = t27.*t603;
t1453 = t19.*t649;
t1463 = -t1225;
t1466 = t10.*t997;
t1468 = -t1236;
t1469 = -t1237;
t1470 = -t1238;
t1482 = t9.*t1009;
t1483 = t10.*t1009;
t1484 = t11.*t1009;
t1491 = t51.*t111.*(-3.0./5.0e+1);
t1495 = t19.*t525;
t1496 = t20.*t526;
t1498 = t52.*t111.*(-1.0./1.0e+1);
t1499 = t48.*t127.*(-1.0./1.0e+1);
t1500 = t52.*t112.*(-1.0./1.0e+1);
t1503 = t52.*t111.*(-3.0./1.0e+1);
t1504 = t48.*t127.*(-3.0./1.0e+1);
t1505 = t52.*t112.*(-3.0./1.0e+1);
t1511 = t60.*t98.*(1.2e+1./2.5e+1);
t1513 = t123.*t230;
t1523 = -t1294;
t1524 = t19.*t528;
t1525 = t9.*t1041;
t1526 = t20.*t529;
t1530 = t52.*t127.*(-1.0./1.0e+1);
t1531 = t52.*t128.*(-1.0./1.0e+1);
t1533 = t59.*t111.*(-1.0./1.0e+1);
t1534 = t51.*t83.*(-1.0./1.0e+1);
t1536 = t52.*t127.*(-3.0./1.0e+1);
t1537 = t52.*t128.*(-3.0./1.0e+1);
t1539 = t59.*t111.*(-3.0./1.0e+1);
t1540 = t51.*t83.*(-3.0./1.0e+1);
t1541 = t51.*t87.*(-3.0./2.5e+1);
t1544 = t49.*t86.*(9.0./5.0e+1);
t1545 = t49.*t85.*(3.9e+1./5.0e+1);
t1546 = t54.*t126.*(3.0./1.0e+2);
t1554 = -t1322;
t1555 = t9.*t1096;
t1556 = t18.*t534;
t1562 = t52.*t86.*(-1.0./1.0e+1);
t1563 = t53.*t86.*(-1.0./1.0e+1);
t1564 = t59.*t127.*(-1.0./1.0e+1);
t1566 = t52.*t86.*(-3.0./1.0e+1);
t1567 = t53.*t86.*(-3.0./1.0e+1);
t1568 = t59.*t127.*(-3.0./1.0e+1);
t1571 = -t1348;
t1575 = -t1362;
t1576 = t9.*t108.*(-9.0./2.0e+2);
t1584 = t11.*t112.*(-9.0./2.0e+2);
t1585 = t59.*t86.*(-1.0./1.0e+1);
t1586 = t59.*t86.*(-3.0./1.0e+1);
t1587 = -t1384;
t1589 = t97.*5.9765625e-3;
t1590 = t95.*1.0675e-2;
t1591 = t96.*1.0675e-2;
t1592 = t97.*1.0675e-2;
t1593 = t98.*1.0675e-2;
t1595 = t9.*t129.*(-9.0./2.0e+2);
t1600 = t101.*1.0675e-2;
t1601 = t103.*1.0675e-2;
t1602 = t104.*1.0675e-2;
t1603 = t105.*1.0675e-2;
t1604 = t106.*1.0675e-2;
t1605 = t107.*1.0675e-2;
t1606 = t108.*1.0675e-2;
t1607 = t112.*1.0675e-2;
t1608 = t108.*2.98828125e-3;
t1609 = t109.*2.98828125e-3;
t1610 = t110.*2.98828125e-3;
t1611 = t111.*2.98828125e-3;
t1612 = t112.*2.98828125e-3;
t1613 = t113.*2.98828125e-3;
t1614 = t114.*2.98828125e-3;
t1623 = t127.*5.9765625e-3;
t1624 = t129.*5.9765625e-3;
t1626 = t117.*1.0675e-2;
t1627 = t118.*1.0675e-2;
t1628 = t121.*1.0675e-2;
t1629 = t122.*1.0675e-2;
t1630 = t123.*1.0675e-2;
t1631 = t124.*1.0675e-2;
t1632 = t125.*1.0675e-2;
t1633 = t126.*1.0675e-2;
t1634 = t127.*1.0675e-2;
t1635 = t128.*1.0675e-2;
t1637 = t4.*t21.*t123.*(3.0./2.5e+1);
t1654 = t19.*t98.*(9.0./1.0e+2);
t1655 = t19.*t98.*(-3.0./2.0e+2);
t1656 = t18.*t888;
t1657 = t9.*t20.*t125.*(6.0./2.5e+1);
t1661 = t117+t190;
t1662 = t122+t191;
t1663 = t125+t194;
t1664 = t128+t195;
t1665 = t19.*t111.*(-3.0./1.0e+2);
t1666 = -t1429;
t1668 = t20.*t110.*(-3.0./1.0e+2);
t1669 = t3.*t6.*t693;
t1670 = -t1434;
t1671 = t51.*t693;
t1673 = t5.*t1223;
t1675 = t25.*t99.*(-3.0./2.0e+2);
t1676 = t19.*t111.*(9.0./2.0e+2);
t1677 = t19.*t909;
t1681 = t19.*t913;
t1682 = t10.*t20.*t313;
t1686 = t27.*t109.*(-3.0./1.0e+2);
t1688 = t27.*t110.*(-3.0./1.0e+2);
t1690 = -t1450;
t1691 = t5.*t11.*t692;
t1692 = t27.*t894;
t1695 = t18.*t130.*(9.0./1.0e+2);
t1697 = t20.*t125.*(-3.0./2.0e+2);
t1698 = t20.*t126.*(-3.0./2.0e+2);
t1700 = t10.*t27.*t313;
t1701 = t26.*t915;
t1703 = t83+t199;
t1704 = t84+t197;
t1705 = t86+t203;
t1706 = t25.*t130.*(9.0./1.0e+2);
t1709 = t27.*t126.*(-3.0./2.0e+2);
t1711 = -t1467;
t1714 = -t1474;
t1715 = -t1476;
t1716 = -t1477;
t1717 = -t1478;
t1718 = t19.*t666;
t1721 = -t1485;
t1722 = -t1486;
t1723 = -t1487;
t1724 = -t1488;
t1727 = t49.*t60.*t164;
t1728 = t49.*t61.*t164;
t1734 = -t1489;
t1736 = t107.*t126.*(6.0./2.5e+1);
t1739 = t18.*t679;
t1742 = t51.*t107.*(9.0./1.0e+2);
t1749 = t56.*t111.*(-3.0./1.0e+2);
t1750 = t54.*t110.*(9.0./1.0e+2);
t1752 = t56.*t107.*(3.9e+1./1.0e+2);
t1753 = t49.*t126.*(-3.0./2.0e+2);
t1754 = t49.*t130.*(-3.0./2.0e+2);
t1755 = t60.*t99.*(-3.0./2.0e+2);
t1758 = t10.*t1347;
t1759 = t19.*t696;
t1761 = t189.*1.35e-3;
t1763 = t49.*t87.*(-3.0./1.0e+2);
t1764 = t50.*t86.*(-3.0./1.0e+2);
t1765 = t49.*t87.*(9.0./1.0e+2);
t1766 = t50.*t86.*(9.0./1.0e+2);
t1767 = t50.*t87.*(9.0./1.0e+2);
t1768 = t4.*t9.*t123.*(-3.0./2.0e+2);
t1778 = t55.*t87.*(-3.0./1.0e+2);
t1779 = t9.*t210.*(9.0./1.0e+2);
t1780 = t202.*1.35e-3;
t1781 = t203.*1.35e-3;
t1782 = t204.*1.35e-3;
t1786 = t210.*1.35e-3;
t1787 = t107.*2.09765625e-2;
t1794 = t215.*1.35e-3;
t1796 = t50.*t668;
t1800 = t18.*t762;
t1802 = -t1617;
t1815 = t123.*1.048828125e-2;
t1816 = t124.*1.048828125e-2;
t1817 = t10.*t27.*t97.*(-3.0./2.5e+1);
t1818 = -t1638;
t1819 = t3.*t12.*t973;
t1820 = t6.*t1438;
t1821 = t5.*t18.*t130.*(-3.0./5.0e+1);
t1827 = t49.*t992;
t1829 = t109.*t531;
t1830 = t110.*t531;
t1833 = -t1651;
t1837 = t9.*t27.*t109.*(-3.0./5.0e+1);
t1838 = t9.*t20.*t125.*(3.0./1.0e+2);
t1844 = t18.*t1125;
t1847 = t9.*t1456;
t1850 = t20.*t109.*(-9.0./2.0e+2);
t1851 = t20.*t110.*(-9.0./2.0e+2);
t1854 = t9.*t27.*t125.*(3.0./1.0e+2);
t1857 = t25.*t114.*(-9.0./2.0e+2);
t1859 = t3.*t4.*t1009;
t1860 = t50.*t1009;
t1862 = t6.*t1479;
t1868 = t6.*t12.*t1009;
t1871 = t9.*t1474;
t1874 = t10.*t1477;
t1875 = t9.*t1478;
t1879 = t10.*t1479;
t1882 = t25.*t87.*(-9.0./2.0e+2);
t1883 = t60.*t1009;
t1885 = t9.*t1485;
t1889 = t11.*t1488;
t1895 = t9.*t1490;
t1896 = t110.*t111.*(-3.0./2.5e+1);
t1898 = t111.*t114.*(-3.0./5.0e+1);
t1900 = -t1733;
t1901 = t26.*t968;
t1902 = t20.*t983;
t1904 = t56.*t203.*(-3.0./2.5e+1);
t1906 = t60.*t195.*(1.2e+1./2.5e+1);
t1907 = t111.*t130.*(-3.0./5.0e+1);
t1911 = t60.*t195.*(3.0./1.0e+2);
t1913 = -t1740;
t1921 = t49.*t110.*(-9.0./2.0e+2);
t1922 = t127.*t130.*(-3.0./5.0e+1);
t1923 = t60.*t203.*(9.0./5.0e+1);
t1931 = -t1757;
t1936 = t54.*t126.*(-9.0./2.0e+2);
t1937 = t9.*t203.*(-9.0./2.0e+2);
t1943 = -t1774;
t1952 = t12.*t98.*9.325e-3;
t1953 = t190.*1.0675e-2;
t1954 = t191.*1.0675e-2;
t1955 = t192.*1.0675e-2;
t1956 = t194.*1.0675e-2;
t1957 = t195.*1.0675e-2;
t1958 = t20.*t1009;
t1959 = t21.*t1009;
t1964 = t5.*t1622;
t1965 = t6.*t1621;
t1966 = t10.*t100.*9.325e-3;
t1970 = t198.*1.0675e-2;
t1971 = t199.*1.0675e-2;
t1973 = t201.*1.0675e-2;
t1974 = t204.*1.0675e-2;
t1975 = t202.*2.98828125e-3;
t1976 = t203.*2.98828125e-3;
t1977 = t204.*2.98828125e-3;
t1980 = t12.*t1621;
t1981 = t210.*5.9765625e-3;
t1982 = t10.*t116.*9.325e-3;
t1984 = t6.*t86.*9.325e-3;
t1985 = t206.*1.0675e-2;
t1986 = t209.*1.0675e-2;
t1987 = t210.*1.0675e-2;
t1988 = t211.*1.0675e-2;
t1990 = t214.*1.0675e-2;
t1991 = t215.*2.98828125e-3;
t1992 = t10.*t20.*t97.*(-3.0./2.5e+1);
t1993 = t11.*t19.*t98.*(-3.0./2.5e+1);
t1994 = t9.*t20.*t97.*(-6.0./2.5e+1);
t1997 = t19.*t1041;
t2003 = -t1828;
t2004 = t109.*t693;
t2005 = t110.*t693;
t2007 = t9.*t20.*t109.*(9.0./1.0e+2);
t2009 = t18.*t1363;
t2010 = t20.*t108.*t188;
t2015 = t18.*t1385;
t2017 = -t1839;
t2018 = -t1840;
t2021 = t27.*t108.*t188;
t2029 = t5.*t25.*t87.*(-3.0./1.0e+2);
t2038 = -t1876;
t2039 = -t1878;
t2040 = -t1880;
t2041 = -t1881;
t2043 = t18.*t1186;
t2047 = -t1886;
t2048 = -t1887;
t2050 = t49.*t87.*t164;
t2054 = t7.*t1741;
t2057 = -t1891;
t2059 = t19.*t1207;
t2067 = t12.*t1741;
t2068 = t7.*t1748;
t2069 = t13.*t1741;
t2073 = t107.*t110.*(9.0./1.0e+2);
t2075 = t26.*t1211;
t2077 = t13.*t1748;
t2080 = t56.*t203.*(-3.0./1.0e+2);
t2081 = t56.*t203.*(9.0./1.0e+2);
t2083 = t26.*t1229;
t2084 = t18.*t1240;
t2087 = -t1919;
t2089 = t11.*t26.*t691;
t2090 = t20.*t25.*t348;
t2093 = -t1951;
t2098 = -t1968;
t2099 = -t1969;
t2106 = t19.*t60.*t98.*(6.0./2.5e+1);
t2115 = t12.*t130.*4.6625e-3;
t2118 = t85.*t666;
t2121 = -t1989;
tau = ft_4({dq1,dq2,dq3,dq4,dq5,dq6,t10,t100,t1001,t1002,t1003,t1004,t1005,t1006,t1007,t1009,t101,t1010,t1011,t1013,t1016,t1018,t1019,t102,t1022,t1023,t1025,t1027,t1029,t103,t1030,t1033,t1034,t1035,t1037,t1039,t104,t1041,t1042,t1043,t1047,t1048,t105,t1050,t1051,t1053,t1055,t1056,t1058,t1059,t106,t1060,t1061,t1062,t1063,t1065,t1067,t1068,t107,t1072,t1073,t1074,t1076,t1077,t1078,t108,t1080,t1081,t1082,t1083,t1084,t1085,t1086,t1087,t1088,t1089,t109,t1090,t1091,t1092,t1095,t1096,t1098,t1099,t11,t110,t1100,t1101,t1102,t1103,t1104,t1105,t1106,t1107,t1108,t111,t1110,t1111,t1112,t1113,t1114,t1116,t1117,t1119,t112,t1120,t1122,t1123,t1124,t1127,t113,t1131,t1132,t1133,t1134,t1135,t114,t1141,t1144,t1145,t1147,t1148,t1149,t1151,t1158,t1159,t116,t1160,t1161,t1162,t1163,t1164,t1165,t1166,t1167,t1169,t117,t1170,t1171,t1172,t1173,t1176,t1177,t1178,t118,t1180,t1182,t1183,t1186,t1188,t1189,t119,t1190,t1191,t1192,t1193,t1194,t1195,t1196,t1198,t1199,t12,t120,t1201,t1202,t1203,t1204,t1205,t1207,t1208,t121,t1210,t1211,t1212,t1214,t1215,t1216,t1217,t1218,t1219,t1220,t1221,t1222,t1224,t1227,t1228,t1229,t123,t1230,t1231,t1233,t1234,t1235,t1239,t124,t1240,t1241,t1242,t1243,t1244,t1245,t1246,t1247,t125,t1254,t1255,t1256,t126,t1263,t1266,t127,t128,t1283,t1286,t1287,t1288,t1289,t129,t1291,t1293,t1295,t1296,t1297,t1298,t1299,t13,t130,t131,t1316,t1317,t1319,t132,t1320,t1323,t1324,t1325,t1326,t1327,t1328,t1329,t133,t1331,t1332,t1333,t1334,t1335,t1345,t1346,t1347,t1349,t135,t1352,t1353,t1355,t1356,t1357,t1358,t1359,t1361,t1362,t1363,t1366,t1369,t137,t1370,t1371,t1372,t1373,t1375,t1376,t1377,t1379,t138,t1380,t1383,t1385,t1386,t1387,t1388,t139,t1390,t1391,t1392,t1393,t1395,t1397,t1398,t1399,t140,t1400,t1401,t1402,t1403,t1404,t1406,t1407,t1408,t1409,t141,t1410,t1413,t1416,t1417,t1419,t142,t1423,t1424,t1426,t1427,t1429,t143,t1432,t1433,t1434,t1435,t1438,t144,t1441,t1442,t1443,t1445,t1447,t145,t1450,t1452,t1453,t1456,t1457,t1458,t146,t1462,t1463,t1464,t1465,t1466,t1467,t1468,t1469,t147,t1470,t1473,t1474,t1475,t1476,t1477,t1478,t1479,t148,t1480,t1481,t1482,t1483,t1484,t1485,t1486,t1487,t1488,t1489,t149,t1490,t1491,t1493,t1494,t1495,t1496,t1497,t1498,t1499,t150,t1500,t1502,t1503,t1504,t1505,t151,t1511,t1513,t152,t1523,t1524,t1525,t1526,t1528,t153,t1530,t1531,t1532,t1533,t1534,t1536,t1537,t1538,t1539,t154,t1540,t1541,t1544,t1545,t1546,t155,t1554,t1555,t1556,t1557,t1558,t1562,t1563,t1564,t1566,t1567,t1568,t1571,t1575,t1576,t158,t1581,t1582,t1584,t1585,t1586,t1587,t1589,t159,t1590,t1591,t1592,t1593,t1595,t1597,t1598,t1599,t160,t1600,t1601,t1602,t1603,t1604,t1605,t1606,t1607,t1608,t1609,t161,t1610,t1611,t1612,t1613,t1614,t1617,t1618,t1619,t162,t1620,t1621,t1622,t1623,t1624,t1626,t1627,t1628,t1629,t163,t1630,t1631,t1632,t1633,t1634,t1635,t1637,t164,t1643,t165,t1654,t1655,t1656,t1657,t166,t1660,t1661,t1662,t1663,t1664,t1665,t1666,t1668,t1669,t167,t1670,t1671,t1673,t1675,t1676,t1677,t168,t1681,t1682,t1684,t1685,t1686,t1688,t1689,t1690,t1691,t1692,t1695,t1696,t1697,t1698,t170,t1700,t1701,t1702,t1703,t1704,t1705,t1706,t1709,t171,t1711,t1713,t1714,t1715,t1716,t1717,t1718,t1719,t1720,t1721,t1722,t1723,t1724,t1726,t1727,t1728,t173,t1730,t1732,t1734,t1736,t1739,t1741,t1742,t1747,t1748,t1749,t1750,t1752,t1753,t1754,t1755,t1756,t1758,t1759,t1760,t1761,t1763,t1764,t1765,t1766,t1767,t1768,t177,t1772,t1773,t1776,t1778,t1779,t178,t1780,t1781,t1782,t1785,t1786,t1787,t179,t1794,t1796,t18,t180,t1800,t1801,t1802,t1803,t1804,t1805,t1806,t1808,t181,t1815,t1816,t1817,t1818,t1819,t182,t1820,t1821,t1822,t1823,t1827,t1828,t1829,t183,t1830,t1831,t1832,t1833,t1837,t1838,t1839,t184,t1840,t1844,t1845,t1847,t1849,t185,t1850,t1851,t1852,t1853,t1854,t1857,t1858,t1859,t186,t1860,t1861,t1862,t1866,t1867,t1868,t1869,t187,t1870,t1871,t1872,t1873,t1874,t1875,t1876,t1877,t1878,t1879,t188,t1881,t1882,t1883,t1884,t1885,t1886,t1888,t1889,t189,t1890,t1893,t1895,t1896,t1897,t1898,t1899,t19,t190,t1900,t1901,t1902,t1904,t1906,t1907,t191,t1911,t1913,t1917,t1919,t192,t1921,t1922,t1923,t1925,t1926,t1927,t193,t1931,t1936,t1937,t194,t1943,t1944,t1947,t1948,t1949,t195,t1950,t1951,t1952,t1953,t1954,t1955,t1956,t1957,t1958,t1959,t196,t1962,t1963,t1964,t1965,t1966,t1967,t1968,t1970,t1971,t1973,t1974,t1975,t1976,t1977,t1978,t1979,t1980,t1981,t1982,t1983,t1984,t1985,t1986,t1987,t1988,t199,t1990,t1991,t1992,t1993,t1994,t1997,t1999,t2,t20,t200,t2001,t2002,t2003,t2004,t2005,t2007,t2008,t2009,t201,t2010,t2014,t2015,t2017,t2018,t202,t2021,t2023,t2024,t2025,t2029,t203,t2030,t2031,t2034,t2035,t2036,t2037,t2038,t2039,t204,t2040,t2041,t2043,t2046,t2047,t2048,t2050,t2052,t2053,t2054,t2055,t2056,t2057,t2058,t2059,t206,t2061,t2063,t2064,t2065,t2066,t2067,t2068,t2069,t2070,t2071,t2072,t2073,t2075,t2076,t2077,t2078,t208,t2080,t2081,t2083,t2084,t2085,t2086,t2087,t2089,t209,t2090,t2091,t2092,t2093,t2094,t2096,t2097,t2098,t2099,t21,t210,t2106,t211,t2111,t2112,t2115,t2118,t212,t2121,t2124,t2125,t2126,t213,t2136,t2137,t214,t2141,t2142,t2143,t2145,t2146,t215,t2153,t2154,t2155,t216,t2163,t2164,t2166,t2167,t217,t2170,t2174,t2176,t218,t219,t2192,t2193,t22,t220,t221,t2212,t2213,t2214,t2215,t2218,t222,t2221,t2222,t2223,t2224,t2225,t2226,t223,t2231,t2232,t2233,t2235,t224,t2240,t2241,t225,t2250,t226,t227,t2277,t2278,t228,t229,t230,t2309,t231,t2316,t2317,t2321,t2323,t2324,t2327,t2328,t2331,t2334,t234,t2343,t235,t2357,t236,t2361,t2362,t2366,t2369,t237,t2371,t2372,t2378,t2379,t238,t2382,t2383,t2387,t2389,t239,t2391,t2395,t2398,t240,t2402,t2409,t241,t2412,t2419,t242,t2423,t2425,t2429,t243,t2430,t2431,t2432,t2433,t244,t245,t2450,t2451,t2453,t2454,t246,t2466,t2467,t247,t2473,t2478,t248,t249,t2494,t2495,t2496,t25,t250,t251,t2519,t252,t2520,t2526,t253,t2540,t2541,t2546,t255,t2556,t2557,t256,t2560,t2561,t2566,t2567,t2568,t2569,t2570,t2571,t2572,t2580,t2581,t2583,t2585,t2586,t2588,t2589,t259,t2590,t2591,t2593,t2595,t2597,t2598,t2599,t26,t260,t2600,t2601,t2602,t2603,t2607,t2608,t2609,t261,t2610,t2611,t2614,t2615,t262,t263,t2632,t2633,t2634,t2635,t2636,t2637,t2639,t2646,t265,t267,t2672,t2684,t2686,t269,t27,t270,t2708,t272,t2725,t2726,t2727,t2729,t273,t2730,t2731,t2732,t2733,t2735,t2738,t274,t2740,t2741,t2742,t2746,t2749,t275,t276,t2762,t2765,t2769,t277,t2771,t2779,t278,t2780,t2785,t2786,t2788,t279,t2791,t2792,t2793,t28,t280,t281,t2822,t2823,t2824,t2825,t283,t284,t285,t2854,t286,t2867,t2868,t2869,t287,t288,t289,t2899,t29,t290,t2900,t2902,t292,t293,t2933,t2935,t2939,t294,t2942,t2948,t295,t2951,t2952,t2953,t296,t2961,t2967,t2968,t297,t2974,t2975,t2977,t2978,t2979,t298,t299,t3,t30,t300,t3002,t301,t3010,t3011,t3013,t3015,t3016,t3017,t302,t3020,t3021,t3023,t303,t3034,t304,t3047,t3049,t305,t3052,t3054,t3056,t3058,t306,t3067,t307,t3075,t3077,t3078,t308,t309,t3099,t31,t3101,t3102,t3109,t311,t3118,t312,t313,t3138,t3139,t314,t3143,t315,t316,t317,t318,t319,t3192,t32,t320,t3204,t3206,t3208,t321,t3210,t3211,t3212,t3213,t3214,t3216,t3217,t322,t323,t3231,t324,t3245,t3246,t325,t326,t3262,t327,t3272,t328,t329,t3298,t3299,t33,t330,t331,t332,t3320,t3326,t333,t3330,t334,t336,t337,t338,t3388,t339,t3396,t34,t341,t342,t343,t344,t345,t3453,t346,t347,t3470,t3471,t3473,t3479,t348,t3480,t3483,t3484,t3485,t3486,t349,t3490,t3491,t3497,t3498,t35,t350,t3501,t3510,t3511,t352,t3521,t3526,t3527,t3528,t3529,t353,t354,t3546,t3547,t3549,t355,t3551,t3559,t356,t3560,t3562,t357,t358,t3589,t3590,t3592,t3593,t3594,t3595,t360,t3608,t3609,t3611,t3612,t3613,t3614,t3615,t3616,t3617,t3627,t3628,t3629,t3630,t3635,t3636,t3637,t364,t3648,t365,t3650,t3651,t367,t368,t3680,t3687,t3690,t3691,t3692,t3704,t3705,t371,t3722,t3723,t3724,t3725,t3726,t373,t375,t376,t377,t3779,t378,t379,t3796,t380,t381,t3811,t382,t3822,t3823,t3824,t3827,t3828,t383,t3839,t384,t385,t386,t3862,t3865,t3868,t387,t3871,t3872,t388,t3884,t389,t3909,t391,t3910,t392,t3932,t3935,t3941,t396,t3960,t3963,t397,t399,t4,t400,t401,t402,t4031,t404,t4042,t4043,t4046,t4047,t405,t4057,t406,t4060,t4061,t4067,t407,t4075,t408,t409,t410,t4103,t4109,t411,t412,t413,t414,t415,t416,t4168,t417,t4174,t418,t419,t420,t4204,t4208,t4209,t421,t4212,t422,t423,t424,t425,t426,t4260,t4261,t4262,t4263,t4265,t427,t4280,t429,t430,t431,t432,t433,t434,t4344,t4345,t4347,t435,t436,t437,t4372,t438,t439,t440,t441,t442,t443,t444,t4451,t4452,t4456,t4457,t4475,t4477,t4478,t450,t4508,t451,t453,t4539,t454,t4542,t4544,t4545,t4546,t4547,t456,t4565,t4566,t4568,t4579,t458,t4581,t4584,t459,t460,t461,t462,t463,t464,t465,t467,t468,t469,t470,t471,t472,t473,t474,t475,t476,t4763,t4765,t4766,t4768,t4769,t477,t4770,t4771,t4773,t478,t479,t48,t480,t4806,t4808,t481,t482,t483,t4830,t4831,t4833,t484,t486,t487,t488,t489,t4895,t4898,t49,t490,t4900,t491,t492,t494,t495,t496,t497,t498,t499,t5,t50,t500,t501,t502,t5041,t5054,t5055,t509,t51,t510,t5103,t511,t512,t513,t514,t515,t516,t517,t5175,t5176,t518,t519,t52,t520,t521,t522,t523,t524,t527,t528,t5280,t529,t53,t530,t531,t533,t534,t5343,t5344,t535,t5354,t5356,t536,t5361,t539,t54,t540,t5411,t542,t543,t545,t546,t547,t548,t5491,t5492,t55,t550,t551,t552,t553,t5551,t5552,t556,t557,t558,t559,t56,t560,t561,t5613,t562,t563,t565,t566,t567,t569,t57,t574,t58,t582,t585,t589,t59,t590,t592,t594,t595,t597,t598,t599,t6,t60,t600,t601,t602,t6023,t604,t605,t606,t608,t609,t61,t610,t611,t613,t614,t616,t617,t62,t624,t63,t630,t632,t635,t636,t641,t643,t644,t645,t647,t6473,t648,t649,t650,t651,t652,t653,t654,t655,t656,t657,t658,t66,t660,t661,t663,t664,t666,t667,t669,t67,t670,t6734,t6735,t6736,t674,t6742,t6743,t6744,t6745,t675,t6754,t6755,t676,t677,t6772,t678,t679,t680,t681,t683,t684,t685,t686,t687,t688,t689,t690,t691,t692,t693,t696,t699,t7,t700,t702,t703,t704,t705,t706,t708,t711,t713,t715,t716,t717,t719,t720,t721,t722,t723,t725,t726,t729,t731,t732,t734,t737,t738,t742,t744,t748,t750,t751,t754,t756,t758,t759,t761,t763,t766,t767,t768,t769,t770,t773,t774,t775,t776,t781,t782,t784,t785,t788,t789,t790,t793,t795,t796,t798,t799,t8,t800,t803,t805,t807,t808,t809,t81,t814,t815,t816,t817,t819,t82,t820,t821,t822,t823,t824,t826,t828,t829,t83,t831,t832,t833,t834,t835,t837,t838,t839,t84,t842,t844,t847,t848,t849,t85,t850,t851,t852,t853,t854,t858,t859,t86,t861,t863,t864,t867,t868,t87,t871,t872,t875,t879,t88,t880,t883,t884,t885,t886,t888,t89,t890,t891,t894,t895,t896,t897,t898,t899,t9,t90,t900,t902,t905,t906,t907,t908,t909,t910,t911,t912,t913,t914,t915,t916,t918,t919,t92,t920,t921,t923,t926,t928,t929,t93,t930,t931,t933,t934,t935,t936,t937,t938,t944,t945,t946,t947,t948,t949,t95,t950,t951,t954,t955,t956,t957,t958,t959,t96,t960,t961,t962,t963,t964,t965,t966,t967,t968,t969,t97,t970,t972,t973,t974,t975,t976,t977,t978,t98,t981,t982,t984,t986,t987,t988,t99,t990,t991,t992,t993,t994,t996,t997,t999});
end
function tau = ft_4(ct)
[dq1,dq2,dq3,dq4,dq5,dq6,t10,t100,t1001,t1002,t1003,t1004,t1005,t1006,t1007,t1009,t101,t1010,t1011,t1013,t1016,t1018,t1019,t102,t1022,t1023,t1025,t1027,t1029,t103,t1030,t1033,t1034,t1035,t1037,t1039,t104,t1041,t1042,t1043,t1047,t1048,t105,t1050,t1051,t1053,t1055,t1056,t1058,t1059,t106,t1060,t1061,t1062,t1063,t1065,t1067,t1068,t107,t1072,t1073,t1074,t1076,t1077,t1078,t108,t1080,t1081,t1082,t1083,t1084,t1085,t1086,t1087,t1088,t1089,t109,t1090,t1091,t1092,t1095,t1096,t1098,t1099,t11,t110,t1100,t1101,t1102,t1103,t1104,t1105,t1106,t1107,t1108,t111,t1110,t1111,t1112,t1113,t1114,t1116,t1117,t1119,t112,t1120,t1122,t1123,t1124,t1127,t113,t1131,t1132,t1133,t1134,t1135,t114,t1141,t1144,t1145,t1147,t1148,t1149,t1151,t1158,t1159,t116,t1160,t1161,t1162,t1163,t1164,t1165,t1166,t1167,t1169,t117,t1170,t1171,t1172,t1173,t1176,t1177,t1178,t118,t1180,t1182,t1183,t1186,t1188,t1189,t119,t1190,t1191,t1192,t1193,t1194,t1195,t1196,t1198,t1199,t12,t120,t1201,t1202,t1203,t1204,t1205,t1207,t1208,t121,t1210,t1211,t1212,t1214,t1215,t1216,t1217,t1218,t1219,t1220,t1221,t1222,t1224,t1227,t1228,t1229,t123,t1230,t1231,t1233,t1234,t1235,t1239,t124,t1240,t1241,t1242,t1243,t1244,t1245,t1246,t1247,t125,t1254,t1255,t1256,t126,t1263,t1266,t127,t128,t1283,t1286,t1287,t1288,t1289,t129,t1291,t1293,t1295,t1296,t1297,t1298,t1299,t13,t130,t131,t1316,t1317,t1319,t132,t1320,t1323,t1324,t1325,t1326,t1327,t1328,t1329,t133,t1331,t1332,t1333,t1334,t1335,t1345,t1346,t1347,t1349,t135,t1352,t1353,t1355,t1356,t1357,t1358,t1359,t1361,t1362,t1363,t1366,t1369,t137,t1370,t1371,t1372,t1373,t1375,t1376,t1377,t1379,t138,t1380,t1383,t1385,t1386,t1387,t1388,t139,t1390,t1391,t1392,t1393,t1395,t1397,t1398,t1399,t140,t1400,t1401,t1402,t1403,t1404,t1406,t1407,t1408,t1409,t141,t1410,t1413,t1416,t1417,t1419,t142,t1423,t1424,t1426,t1427,t1429,t143,t1432,t1433,t1434,t1435,t1438,t144,t1441,t1442,t1443,t1445,t1447,t145,t1450,t1452,t1453,t1456,t1457,t1458,t146,t1462,t1463,t1464,t1465,t1466,t1467,t1468,t1469,t147,t1470,t1473,t1474,t1475,t1476,t1477,t1478,t1479,t148,t1480,t1481,t1482,t1483,t1484,t1485,t1486,t1487,t1488,t1489,t149,t1490,t1491,t1493,t1494,t1495,t1496,t1497,t1498,t1499,t150,t1500,t1502,t1503,t1504,t1505,t151,t1511,t1513,t152,t1523,t1524,t1525,t1526,t1528,t153,t1530,t1531,t1532,t1533,t1534,t1536,t1537,t1538,t1539,t154,t1540,t1541,t1544,t1545,t1546,t155,t1554,t1555,t1556,t1557,t1558,t1562,t1563,t1564,t1566,t1567,t1568,t1571,t1575,t1576,t158,t1581,t1582,t1584,t1585,t1586,t1587,t1589,t159,t1590,t1591,t1592,t1593,t1595,t1597,t1598,t1599,t160,t1600,t1601,t1602,t1603,t1604,t1605,t1606,t1607,t1608,t1609,t161,t1610,t1611,t1612,t1613,t1614,t1617,t1618,t1619,t162,t1620,t1621,t1622,t1623,t1624,t1626,t1627,t1628,t1629,t163,t1630,t1631,t1632,t1633,t1634,t1635,t1637,t164,t1643,t165,t1654,t1655,t1656,t1657,t166,t1660,t1661,t1662,t1663,t1664,t1665,t1666,t1668,t1669,t167,t1670,t1671,t1673,t1675,t1676,t1677,t168,t1681,t1682,t1684,t1685,t1686,t1688,t1689,t1690,t1691,t1692,t1695,t1696,t1697,t1698,t170,t1700,t1701,t1702,t1703,t1704,t1705,t1706,t1709,t171,t1711,t1713,t1714,t1715,t1716,t1717,t1718,t1719,t1720,t1721,t1722,t1723,t1724,t1726,t1727,t1728,t173,t1730,t1732,t1734,t1736,t1739,t1741,t1742,t1747,t1748,t1749,t1750,t1752,t1753,t1754,t1755,t1756,t1758,t1759,t1760,t1761,t1763,t1764,t1765,t1766,t1767,t1768,t177,t1772,t1773,t1776,t1778,t1779,t178,t1780,t1781,t1782,t1785,t1786,t1787,t179,t1794,t1796,t18,t180,t1800,t1801,t1802,t1803,t1804,t1805,t1806,t1808,t181,t1815,t1816,t1817,t1818,t1819,t182,t1820,t1821,t1822,t1823,t1827,t1828,t1829,t183,t1830,t1831,t1832,t1833,t1837,t1838,t1839,t184,t1840,t1844,t1845,t1847,t1849,t185,t1850,t1851,t1852,t1853,t1854,t1857,t1858,t1859,t186,t1860,t1861,t1862,t1866,t1867,t1868,t1869,t187,t1870,t1871,t1872,t1873,t1874,t1875,t1876,t1877,t1878,t1879,t188,t1881,t1882,t1883,t1884,t1885,t1886,t1888,t1889,t189,t1890,t1893,t1895,t1896,t1897,t1898,t1899,t19,t190,t1900,t1901,t1902,t1904,t1906,t1907,t191,t1911,t1913,t1917,t1919,t192,t1921,t1922,t1923,t1925,t1926,t1927,t193,t1931,t1936,t1937,t194,t1943,t1944,t1947,t1948,t1949,t195,t1950,t1951,t1952,t1953,t1954,t1955,t1956,t1957,t1958,t1959,t196,t1962,t1963,t1964,t1965,t1966,t1967,t1968,t1970,t1971,t1973,t1974,t1975,t1976,t1977,t1978,t1979,t1980,t1981,t1982,t1983,t1984,t1985,t1986,t1987,t1988,t199,t1990,t1991,t1992,t1993,t1994,t1997,t1999,t2,t20,t200,t2001,t2002,t2003,t2004,t2005,t2007,t2008,t2009,t201,t2010,t2014,t2015,t2017,t2018,t202,t2021,t2023,t2024,t2025,t2029,t203,t2030,t2031,t2034,t2035,t2036,t2037,t2038,t2039,t204,t2040,t2041,t2043,t2046,t2047,t2048,t2050,t2052,t2053,t2054,t2055,t2056,t2057,t2058,t2059,t206,t2061,t2063,t2064,t2065,t2066,t2067,t2068,t2069,t2070,t2071,t2072,t2073,t2075,t2076,t2077,t2078,t208,t2080,t2081,t2083,t2084,t2085,t2086,t2087,t2089,t209,t2090,t2091,t2092,t2093,t2094,t2096,t2097,t2098,t2099,t21,t210,t2106,t211,t2111,t2112,t2115,t2118,t212,t2121,t2124,t2125,t2126,t213,t2136,t2137,t214,t2141,t2142,t2143,t2145,t2146,t215,t2153,t2154,t2155,t216,t2163,t2164,t2166,t2167,t217,t2170,t2174,t2176,t218,t219,t2192,t2193,t22,t220,t221,t2212,t2213,t2214,t2215,t2218,t222,t2221,t2222,t2223,t2224,t2225,t2226,t223,t2231,t2232,t2233,t2235,t224,t2240,t2241,t225,t2250,t226,t227,t2277,t2278,t228,t229,t230,t2309,t231,t2316,t2317,t2321,t2323,t2324,t2327,t2328,t2331,t2334,t234,t2343,t235,t2357,t236,t2361,t2362,t2366,t2369,t237,t2371,t2372,t2378,t2379,t238,t2382,t2383,t2387,t2389,t239,t2391,t2395,t2398,t240,t2402,t2409,t241,t2412,t2419,t242,t2423,t2425,t2429,t243,t2430,t2431,t2432,t2433,t244,t245,t2450,t2451,t2453,t2454,t246,t2466,t2467,t247,t2473,t2478,t248,t249,t2494,t2495,t2496,t25,t250,t251,t2519,t252,t2520,t2526,t253,t2540,t2541,t2546,t255,t2556,t2557,t256,t2560,t2561,t2566,t2567,t2568,t2569,t2570,t2571,t2572,t2580,t2581,t2583,t2585,t2586,t2588,t2589,t259,t2590,t2591,t2593,t2595,t2597,t2598,t2599,t26,t260,t2600,t2601,t2602,t2603,t2607,t2608,t2609,t261,t2610,t2611,t2614,t2615,t262,t263,t2632,t2633,t2634,t2635,t2636,t2637,t2639,t2646,t265,t267,t2672,t2684,t2686,t269,t27,t270,t2708,t272,t2725,t2726,t2727,t2729,t273,t2730,t2731,t2732,t2733,t2735,t2738,t274,t2740,t2741,t2742,t2746,t2749,t275,t276,t2762,t2765,t2769,t277,t2771,t2779,t278,t2780,t2785,t2786,t2788,t279,t2791,t2792,t2793,t28,t280,t281,t2822,t2823,t2824,t2825,t283,t284,t285,t2854,t286,t2867,t2868,t2869,t287,t288,t289,t2899,t29,t290,t2900,t2902,t292,t293,t2933,t2935,t2939,t294,t2942,t2948,t295,t2951,t2952,t2953,t296,t2961,t2967,t2968,t297,t2974,t2975,t2977,t2978,t2979,t298,t299,t3,t30,t300,t3002,t301,t3010,t3011,t3013,t3015,t3016,t3017,t302,t3020,t3021,t3023,t303,t3034,t304,t3047,t3049,t305,t3052,t3054,t3056,t3058,t306,t3067,t307,t3075,t3077,t3078,t308,t309,t3099,t31,t3101,t3102,t3109,t311,t3118,t312,t313,t3138,t3139,t314,t3143,t315,t316,t317,t318,t319,t3192,t32,t320,t3204,t3206,t3208,t321,t3210,t3211,t3212,t3213,t3214,t3216,t3217,t322,t323,t3231,t324,t3245,t3246,t325,t326,t3262,t327,t3272,t328,t329,t3298,t3299,t33,t330,t331,t332,t3320,t3326,t333,t3330,t334,t336,t337,t338,t3388,t339,t3396,t34,t341,t342,t343,t344,t345,t3453,t346,t347,t3470,t3471,t3473,t3479,t348,t3480,t3483,t3484,t3485,t3486,t349,t3490,t3491,t3497,t3498,t35,t350,t3501,t3510,t3511,t352,t3521,t3526,t3527,t3528,t3529,t353,t354,t3546,t3547,t3549,t355,t3551,t3559,t356,t3560,t3562,t357,t358,t3589,t3590,t3592,t3593,t3594,t3595,t360,t3608,t3609,t3611,t3612,t3613,t3614,t3615,t3616,t3617,t3627,t3628,t3629,t3630,t3635,t3636,t3637,t364,t3648,t365,t3650,t3651,t367,t368,t3680,t3687,t3690,t3691,t3692,t3704,t3705,t371,t3722,t3723,t3724,t3725,t3726,t373,t375,t376,t377,t3779,t378,t379,t3796,t380,t381,t3811,t382,t3822,t3823,t3824,t3827,t3828,t383,t3839,t384,t385,t386,t3862,t3865,t3868,t387,t3871,t3872,t388,t3884,t389,t3909,t391,t3910,t392,t3932,t3935,t3941,t396,t3960,t3963,t397,t399,t4,t400,t401,t402,t4031,t404,t4042,t4043,t4046,t4047,t405,t4057,t406,t4060,t4061,t4067,t407,t4075,t408,t409,t410,t4103,t4109,t411,t412,t413,t414,t415,t416,t4168,t417,t4174,t418,t419,t420,t4204,t4208,t4209,t421,t4212,t422,t423,t424,t425,t426,t4260,t4261,t4262,t4263,t4265,t427,t4280,t429,t430,t431,t432,t433,t434,t4344,t4345,t4347,t435,t436,t437,t4372,t438,t439,t440,t441,t442,t443,t444,t4451,t4452,t4456,t4457,t4475,t4477,t4478,t450,t4508,t451,t453,t4539,t454,t4542,t4544,t4545,t4546,t4547,t456,t4565,t4566,t4568,t4579,t458,t4581,t4584,t459,t460,t461,t462,t463,t464,t465,t467,t468,t469,t470,t471,t472,t473,t474,t475,t476,t4763,t4765,t4766,t4768,t4769,t477,t4770,t4771,t4773,t478,t479,t48,t480,t4806,t4808,t481,t482,t483,t4830,t4831,t4833,t484,t486,t487,t488,t489,t4895,t4898,t49,t490,t4900,t491,t492,t494,t495,t496,t497,t498,t499,t5,t50,t500,t501,t502,t5041,t5054,t5055,t509,t51,t510,t5103,t511,t512,t513,t514,t515,t516,t517,t5175,t5176,t518,t519,t52,t520,t521,t522,t523,t524,t527,t528,t5280,t529,t53,t530,t531,t533,t534,t5343,t5344,t535,t5354,t5356,t536,t5361,t539,t54,t540,t5411,t542,t543,t545,t546,t547,t548,t5491,t5492,t55,t550,t551,t552,t553,t5551,t5552,t556,t557,t558,t559,t56,t560,t561,t5613,t562,t563,t565,t566,t567,t569,t57,t574,t58,t582,t585,t589,t59,t590,t592,t594,t595,t597,t598,t599,t6,t60,t600,t601,t602,t6023,t604,t605,t606,t608,t609,t61,t610,t611,t613,t614,t616,t617,t62,t624,t63,t630,t632,t635,t636,t641,t643,t644,t645,t647,t6473,t648,t649,t650,t651,t652,t653,t654,t655,t656,t657,t658,t66,t660,t661,t663,t664,t666,t667,t669,t67,t670,t6734,t6735,t6736,t674,t6742,t6743,t6744,t6745,t675,t6754,t6755,t676,t677,t6772,t678,t679,t680,t681,t683,t684,t685,t686,t687,t688,t689,t690,t691,t692,t693,t696,t699,t7,t700,t702,t703,t704,t705,t706,t708,t711,t713,t715,t716,t717,t719,t720,t721,t722,t723,t725,t726,t729,t731,t732,t734,t737,t738,t742,t744,t748,t750,t751,t754,t756,t758,t759,t761,t763,t766,t767,t768,t769,t770,t773,t774,t775,t776,t781,t782,t784,t785,t788,t789,t790,t793,t795,t796,t798,t799,t8,t800,t803,t805,t807,t808,t809,t81,t814,t815,t816,t817,t819,t82,t820,t821,t822,t823,t824,t826,t828,t829,t83,t831,t832,t833,t834,t835,t837,t838,t839,t84,t842,t844,t847,t848,t849,t85,t850,t851,t852,t853,t854,t858,t859,t86,t861,t863,t864,t867,t868,t87,t871,t872,t875,t879,t88,t880,t883,t884,t885,t886,t888,t89,t890,t891,t894,t895,t896,t897,t898,t899,t9,t90,t900,t902,t905,t906,t907,t908,t909,t910,t911,t912,t913,t914,t915,t916,t918,t919,t92,t920,t921,t923,t926,t928,t929,t93,t930,t931,t933,t934,t935,t936,t937,t938,t944,t945,t946,t947,t948,t949,t95,t950,t951,t954,t955,t956,t957,t958,t959,t96,t960,t961,t962,t963,t964,t965,t966,t967,t968,t969,t97,t970,t972,t973,t974,t975,t976,t977,t978,t98,t981,t982,t984,t986,t987,t988,t99,t990,t991,t992,t993,t994,t996,t997,t999] = ct{:};
t2128 = t28.*t49.*t85.*(3.0./5.0e+1);
t2132 = -t1999;
t2134 = -t2008;
t2135 = t10.*t20.*t108.*(-9.0./2.0e+2);
t2138 = t49.*t1478;
t2139 = t10.*t27.*t108.*(-9.0./2.0e+2);
t2140 = t11.*t26.*t111.*(-9.0./2.0e+2);
t2144 = t20.*t1597;
t2148 = t107.*t1009;
t2152 = t6.*t1869;
t2156 = t22.*t108.*2.75390625e-3;
t2157 = t22.*t109.*2.75390625e-3;
t2158 = t22.*t110.*2.75390625e-3;
t2159 = t22.*t111.*2.75390625e-3;
t2160 = t22.*t112.*2.75390625e-3;
t2161 = t22.*t113.*2.75390625e-3;
t2162 = t22.*t114.*2.75390625e-3;
t2165 = t20.*t1617;
t2169 = t20.*t1619;
t2171 = t12.*t58.*t1009;
t2172 = t21.*t1620;
t2175 = t21.*t117.*9.325e-3;
t2177 = t21.*t124.*9.325e-3;
t2178 = t22.*t123.*2.75390625e-3;
t2179 = t22.*t124.*2.75390625e-3;
t2180 = t29.*t108.*2.75390625e-3;
t2181 = t29.*t109.*2.75390625e-3;
t2182 = t29.*t110.*2.75390625e-3;
t2183 = t29.*t111.*2.75390625e-3;
t2184 = t29.*t112.*2.75390625e-3;
t2185 = t29.*t113.*2.75390625e-3;
t2186 = t29.*t114.*2.75390625e-3;
t2187 = t28.*t117.*9.325e-3;
t2188 = t21.*t83.*9.325e-3;
t2189 = t28.*t124.*9.325e-3;
t2190 = t22.*t86.*2.75390625e-3;
t2191 = t22.*t87.*2.75390625e-3;
t2196 = t28.*t83.*9.325e-3;
t2197 = t29.*t86.*2.75390625e-3;
t2198 = t29.*t87.*2.75390625e-3;
t2199 = t7.*t346.*(9.0./3.2e+2);
t2201 = t3.*t4.*t20.*t530;
t2203 = t49.*t51.*t86.*(-3.0./5.0e+1);
t2204 = t49.*t51.*t87.*(-3.0./5.0e+1);
t2205 = t13.*t346.*(9.0./1.6e+2);
t2206 = t11.*t1899;
t2208 = t3.*t4.*t20.*t533;
t2216 = -t2055;
t2217 = -t2056;
t2219 = t18.*t1458;
t2227 = -t2072;
t2229 = t61.*t1528;
t2236 = t97.*t957;
t2237 = t98.*t957;
t2238 = t99.*t957;
t2239 = t49.*t104.*9.325e-3;
t2242 = t20.*t1474;
t2243 = t20.*t1475;
t2245 = t20.*t1477;
t2246 = t20.*t1478;
t2247 = t21.*t1478;
t2248 = t21.*t1479;
t2249 = t62.*t97.*3.73e-2;
t2251 = t56.*t107.*1.865e-2;
t2252 = t3.*t4.*t1620;
t2253 = t107.*t957;
t2254 = t108.*t957;
t2256 = t110.*t957;
t2258 = t50.*t1621;
t2259 = t112.*t957;
t2263 = t49.*t120.*9.325e-3;
t2264 = t55.*t104.*9.325e-3;
t2265 = t49.*t121.*9.325e-3;
t2266 = t6.*t12.*t101.*9.325e-3;
t2267 = t6.*t12.*t102.*9.325e-3;
t2268 = t58.*t111.*9.325e-3;
t2269 = t9.*t12.*t99.*9.325e-3;
t2281 = t20.*t1485;
t2282 = t20.*t1486;
t2283 = t26.*t1477;
t2284 = t27.*t1478;
t2285 = t28.*t1479;
t2287 = t126.*t957;
t2289 = t54.*t1622;
t2290 = t127.*t957;
t2292 = t129.*t957;
t2293 = t5.*t1979;
t2296 = t49.*t84.*9.325e-3;
t2297 = t50.*t83.*9.325e-3;
t2299 = t6.*t12.*t118.*9.325e-3;
t2300 = t8.*t12.*t112.*9.325e-3;
t2301 = t58.*t127.*9.325e-3;
t2310 = t86.*t957;
t2312 = t6.*t12.*t83.*9.325e-3;
t2313 = t58.*t86.*9.325e-3;
t2314 = t18.*t1493;
t2319 = t20.*t62.*t97.*(-3.0./5.0e+1);
t2322 = t9.*t12.*t20.*t109.*(-3.0./5.0e+1);
t2326 = t5.*t12.*t25.*t130.*(-3.0./5.0e+1);
t2329 = -t2142;
t2330 = -t2143;
t2332 = -t2146;
t2333 = -t2153;
t2338 = -t2164;
t2339 = -t2166;
t2342 = -t2170;
t2344 = -t2174;
t2356 = t97.*t1323;
t2358 = t7.*t2052;
t2363 = -t2192;
t2364 = t3.*t2063;
t2365 = t107.*t1323;
t2368 = t13.*t2052;
t2370 = t10.*t2053;
t2374 = t7.*t2064;
t2376 = t12.*t2053;
t2381 = t9.*t2056;
t2386 = t7.*t346.*5.625e-3;
t2390 = t127.*t1323;
t2392 = t129.*t1323;
t2394 = t7.*t2076;
t2396 = t10.*t2066;
t2397 = t12.*t2064;
t2400 = t13.*t2064;
t2401 = t7.*t13.*t1747;
t2403 = t13.*t2065;
t2405 = t10.*t2071;
t2408 = t13.*t2070;
t2410 = t9.*t2072;
t2413 = t18.*t1689;
t2414 = t5.*t11.*t19.*t691;
t2416 = -t2214;
t2417 = -t2218;
t2418 = t13.*t2076;
t2421 = -t2224;
t2422 = -t2225;
t2424 = -t2232;
t2426 = t7.*t13.*t97.*(-5.5078125e-3);
t2427 = t7.*t13.*t98.*(-5.5078125e-3);
t2428 = -t2241;
t2436 = t7.*t13.*t109.*(-5.5078125e-3);
t2437 = t7.*t13.*t110.*(-5.5078125e-3);
t2438 = t7.*t13.*t111.*(-5.5078125e-3);
t2439 = t7.*t13.*t113.*(-5.5078125e-3);
t2440 = t7.*t13.*t114.*(-5.5078125e-3);
t2449 = t9.*t2094;
t2452 = t7.*t13.*t125.*(-5.5078125e-3);
t2455 = t7.*t13.*t128.*(-5.5078125e-3);
t2456 = t7.*t13.*t130.*(-5.5078125e-3);
t2457 = t5.*t2112;
t2459 = t2.*t6.*t86.*(-9.325e-3);
t2464 = -t2309;
t2465 = t7.*t13.*t87.*(-5.5078125e-3);
t2468 = t7.*t2125;
t2469 = t19.*t20.*t683;
t2470 = -t2316;
t2471 = -t2317;
t2472 = t9.*t2124;
t2474 = t10.*t2125;
t2475 = t22.*t1747;
t2476 = t10.*t2126;
t2477 = t22.*t1748;
t2479 = t19.*t20.*t691;
t2481 = -t2321;
t2482 = t30+t144+t150;
t2483 = t31+t145+t151;
t2484 = t32+t146+t152;
t2485 = t33+t147+t153;
t2486 = t34+t148+t154;
t2487 = t35+t149+t155;
t2488 = t19.*t49.*t86.*(9.0./1.0e+2);
t2491 = -t2328;
t2492 = t10.*t21.*t100.*1.865e-2;
t2498 = t49.*t61.*t1009;
t2504 = t58.*t1866;
t2508 = t57.*t1869;
t2511 = t20.*t1967;
t2512 = t28.*t190.*9.325e-3;
t2513 = t21.*t199.*9.325e-3;
t2514 = t21.*t1968;
t2515 = t22.*t202.*2.75390625e-3;
t2516 = t22.*t203.*2.75390625e-3;
t2517 = t22.*t204.*2.75390625e-3;
t2518 = t10.*t21.*t116.*1.865e-2;
t2523 = t6.*t19.*t86.*1.865e-2;
t2524 = t9.*t29.*t109.*5.5078125e-3;
t2525 = t55.*t61.*t1009;
t2527 = t11.*t29.*t112.*5.5078125e-3;
t2529 = t6.*t86.*t1009;
t2531 = t12.*t130.*t1009;
t2534 = t28.*t199.*9.325e-3;
t2536 = t29.*t202.*2.75390625e-3;
t2537 = t29.*t203.*2.75390625e-3;
t2538 = t29.*t204.*2.75390625e-3;
t2542 = t22.*t215.*2.75390625e-3;
t2547 = t29.*t215.*2.75390625e-3;
t2548 = t4.*t13.*t346.*(9.0./3.2e+2);
t2550 = t6.*t13.*t346.*(9.0./3.2e+2);
t2552 = t18.*t1822;
t2553 = t18.*t1823;
t2554 = t63.*t97.*(-2.75390625e-3);
t2555 = t7.*t2212;
t2559 = t19.*t20.*t1095;
t2563 = t12.*t13.*t346.*(9.0./3.2e+2);
t2564 = -t2361;
t2565 = t63.*t107.*(-2.75390625e-3);
t2573 = t63.*t108.*1.376953125e-3;
t2574 = t63.*t109.*1.376953125e-3;
t2575 = t63.*t110.*1.376953125e-3;
t2576 = t63.*t111.*1.376953125e-3;
t2577 = t63.*t112.*1.376953125e-3;
t2578 = t63.*t113.*1.376953125e-3;
t2579 = t63.*t114.*1.376953125e-3;
t2582 = t3.*t9.*t1919;
t2587 = t9.*t2218;
t2594 = -t2389;
t2596 = t63.*t129.*(-2.75390625e-3);
t2604 = t63.*t123.*1.376953125e-3;
t2605 = t63.*t124.*1.376953125e-3;
t2616 = t63.*t86.*1.376953125e-3;
t2617 = t63.*t87.*1.376953125e-3;
t2622 = t7.*t11.*t13.*t99.*1.1015625e-2;
t2623 = t12.*t58.*t96.*1.865e-2;
t2625 = t49.*t1962;
t2628 = t98.*t1621;
t2629 = t58.*t1947;
t2631 = t12.*t51.*t103.*9.325e-3;
t2638 = t9.*t2240;
t2644 = t19.*t1866;
t2649 = t21.*t1866;
t2650 = t20.*t1867;
t2652 = t21.*t1869;
t2659 = t21.*t1876;
t2660 = t21.*t1877;
t2661 = t21.*t1878;
t2665 = t12.*t58.*t100.*3.73e-2;
t2666 = t62.*t194.*3.73e-2;
t2667 = t7.*t11.*t13.*t112.*1.1015625e-2;
t2668 = t61.*t191.*1.865e-2;
t2669 = t12.*t58.*t104.*1.865e-2;
t2670 = t12.*t58.*t106.*1.865e-2;
t2671 = t86.*t99.*1.865e-2;
t2673 = t60.*t1947;
t2674 = t202.*t957;
t2675 = t203.*t957;
t2679 = t114.*t1622;
t2681 = t6.*t12.*t196.*9.325e-3;
t2682 = t12.*t52.*t112.*9.325e-3;
t2683 = t12.*t58.*t103.*9.325e-3;
t2685 = t9.*t2277;
t2689 = t21.*t1886;
t2692 = t28.*t1876;
t2694 = t28.*t1878;
t2696 = t12.*t51.*t82.*3.73e-2;
t2697 = t50.*t214.*1.865e-2;
t2698 = t12.*t51.*t84.*1.865e-2;
t2700 = t210.*t957;
t2701 = t129.*t1619;
t2702 = t55.*t1979;
t2703 = t211.*t957;
t2705 = t127.*t1621;
t2706 = t12.*t58.*t118.*9.325e-3;
t2707 = t12.*t58.*t119.*9.325e-3;
t2711 = t56.*t107.*6.88175e-1;
t2723 = t12.*t97.*2.98328125e-2;
t2724 = t12.*t98.*2.98328125e-2;
t2734 = t20.*t1919;
t2736 = t12.*t112.*2.98328125e-2;
t2739 = t10.*t2324;
t2744 = t6.*t86.*2.98328125e-2;
t2745 = t12.*t130.*2.98328125e-2;
t2747 = t18.*t50.*t87.*(-9.0./1.0e+2);
t2748 = t18.*t1944;
t2751 = t12.*t19.*t98.*1.865e-2;
t2752 = t49.*t56.*t1009;
t2753 = t12.*t97.*t1009;
t2754 = t3.*t4.*t1870;
t2755 = t12.*t98.*t1009;
t2756 = t12.*t99.*t1009;
t2757 = t20.*t1950;
t2758 = t21.*t190.*9.325e-3;
t2759 = t21.*t1951;
t2763 = t9.*t22.*t109.*(-5.5078125e-3);
t2764 = t11.*t22.*t112.*(-5.5078125e-3);
t2766 = t12.*t22.*t112.*(-5.5078125e-3);
t2767 = t12.*t22.*t114.*(-5.5078125e-3);
t2770 = t10.*t20.*t100.*(-9.325e-3);
t2776 = t7.*t98.*t1323;
t2778 = -t2519;
t2782 = -t2526;
t2784 = t25.*t2096;
t2795 = t4.*t2366;
t2800 = t12.*t98.*t1323;
t2802 = t3.*t4.*t2071;
t2803 = t13.*t98.*t1323;
t2804 = t12.*t99.*t1323;
t2806 = t13.*t99.*t1323;
t2807 = t7.*t114.*t1323;
t2809 = t51.*t2070;
t2810 = t51.*t2071;
t2812 = t3.*t2378;
t2813 = t3.*t2382;
t2814 = -t2540;
t2815 = t6.*t7.*t346.*(9.0./8.0e+2);
t2819 = t20.*t2125;
t2820 = t20.*t2126;
t2821 = t22.*t2125;
t2827 = t7.*t123.*t1323;
t2828 = t7.*t124.*t1323;
t2829 = t13.*t108.*t1323;
t2830 = t13.*t109.*t1323;
t2832 = t7.*t125.*t1323;
t2833 = t13.*t110.*t1323;
t2834 = t7.*t126.*t1323;
t2836 = t13.*t111.*t1323;
t2839 = t13.*t112.*t1323;
t2842 = t7.*t128.*t1323;
t2843 = t13.*t113.*t1323;
t2844 = t13.*t114.*t1323;
t2850 = t57.*t2071;
t2858 = t4.*t13.*t346.*5.625e-3;
t2860 = t5.*t13.*t346.*5.625e-3;
t2862 = t6.*t13.*t346.*5.625e-3;
t2864 = t5.*t13.*t346.*1.6875e-2;
t2865 = t7.*t11.*t346.*1.6875e-2;
t2866 = -t2557;
t2870 = t210.*t1323;
t2871 = t13.*t123.*t1323;
t2872 = t13.*t124.*t1323;
t2873 = t7.*t85.*t1323;
t2877 = t86.*t1741;
t2880 = t12.*t130.*t1323;
t2882 = t13.*t130.*t1323;
t2883 = t60.*t2071;
t2885 = t62.*t2071;
t2887 = -t2561;
t2888 = t10.*t13.*t346.*(-9.0./1.6e+2);
t2890 = t10.*t13.*t346.*5.625e-3;
t2891 = t11.*t13.*t346.*5.625e-3;
t2892 = t12.*t13.*t346.*5.625e-3;
t2901 = -t2586;
t2903 = -t2588;
t2904 = -t2589;
t2905 = -t2590;
t2906 = -t2591;
t2911 = -t2608;
t2912 = -t2611;
t2913 = t7.*t13.*t60.*t98.*2.203125e-2;
t2916 = t51.*t2094;
t2919 = t97.*t1803;
t2921 = t7.*t13.*t194.*(-5.5078125e-3);
t2922 = t7.*t13.*t195.*(-5.5078125e-3);
t2923 = t98.*t1805;
t2924 = t12.*t52.*t98.*(-9.325e-3);
t2925 = -t2633;
t2926 = -t2634;
t2927 = -t2635;
t2928 = -t2636;
t2929 = -t2637;
t2930 = -t2639;
t2931 = t19.*t2034;
t2932 = t21.*t2034;
t2934 = t6.*t12.*t2094;
t2937 = t20.*t2037;
t2938 = t21.*t2036;
t2940 = t10.*t2433;
t2943 = t7.*t13.*t204.*(-5.5078125e-3);
t2944 = t6.*t2454;
t2945 = t112.*t1806;
t2946 = t114.*t1806;
t2947 = -t2684;
t2949 = t27.*t2036;
t2950 = t27.*t2037;
t2954 = t10.*t2451;
t2956 = t125.*t1803;
t2957 = t7.*t13.*t210.*(-5.5078125e-3);
t2959 = t56.*t2111;
t2960 = t127.*t1805;
t2962 = t3.*t4.*t2125;
t2964 = t22.*t2052;
t2965 = t19.*t2055;
t2966 = -t2708;
t2970 = t62.*t97.*5.9665625e-2;
t2973 = t7.*t13.*t215.*(-5.5078125e-3);
t2981 = t18.*t2063;
t2983 = t3.*t21.*t1747;
t2984 = t4.*t20.*t1747;
t2986 = t22.*t2063;
t2988 = t5.*t21.*t1748;
t2991 = t18.*t2071;
t2995 = t19.*t2071;
t2997 = t20.*t2071;
t2998 = t21.*t2071;
t3003 = t4.*t27.*t1747;
t3004 = t22.*t2076;
t3006 = t10.*t2478;
t3007 = t20.*t2078;
t3012 = -t2731;
t3025 = t21.*t2094;
t3028 = t13.*t51.*t346.*(9.0./3.2e+2);
t3035 = t7.*t63.*t98.*(-2.75390625e-3);
t3036 = t7.*t63.*t99.*(-2.75390625e-3);
t3037 = t49.*t2218;
t3040 = t3.*t10.*t13.*t346.*(9.0./3.2e+2);
t3042 = t13.*t58.*t346.*(9.0./3.2e+2);
t3046 = -t2791;
t3051 = t7.*t63.*t108.*(-2.75390625e-3);
t3053 = t7.*t63.*t112.*(-2.75390625e-3);
t3057 = t6.*t7.*t346.*(-5.625e-3);
t3059 = t20.*t2324;
t3060 = t103+t104+t214;
t3061 = t110+t111+t215;
t3062 = t13.*t62.*t346.*(9.0./3.2e+2);
t3064 = -t2823;
t3065 = -t2824;
t3066 = t13.*t63.*t108.*(-2.75390625e-3);
t3068 = t13.*t63.*t110.*(-2.75390625e-3);
t3069 = t12.*t63.*t112.*(-2.75390625e-3);
t3070 = t13.*t63.*t111.*(-2.75390625e-3);
t3071 = t12.*t63.*t114.*(-2.75390625e-3);
t3072 = t13.*t63.*t112.*(-2.75390625e-3);
t3073 = t7.*t63.*t127.*(-2.75390625e-3);
t3074 = t13.*t63.*t114.*(-2.75390625e-3);
t3076 = t7.*t63.*t130.*(-2.75390625e-3);
t3079 = t13.*t2572;
t3080 = t63.*t202.*1.376953125e-3;
t3081 = t63.*t203.*1.376953125e-3;
t3082 = t63.*t204.*1.376953125e-3;
t3083 = t10.*t56.*t1919;
t3085 = t9.*t2585;
t3087 = t21.*t123.*1.491640625e-2;
t3088 = t21.*t124.*1.491640625e-2;
t3091 = t7.*t12.*t346.*(-5.625e-3);
t3092 = -t2868;
t3093 = t63.*t210.*(-2.75390625e-3);
t3094 = t13.*t63.*t125.*(-2.75390625e-3);
t3095 = t13.*t63.*t126.*(-2.75390625e-3);
t3096 = t10.*t2598;
t3097 = t13.*t63.*t128.*(-2.75390625e-3);
t3100 = t12.*t2602;
t3103 = t28.*t123.*1.491640625e-2;
t3104 = t28.*t124.*1.491640625e-2;
t3107 = t12.*t98.*t104.*1.865e-2;
t3108 = t111.*t1948;
t3110 = t13.*t63.*t86.*(-2.75390625e-3);
t3111 = t13.*t63.*t87.*(-2.75390625e-3);
t3112 = t63.*t215.*1.376953125e-3;
t3126 = t21.*t2153;
t3128 = t21.*t2155;
t3131 = t7.*t13.*t57.*t107.*1.1015625e-2;
t3132 = t7.*t13.*t49.*t130.*1.1015625e-2;
t3133 = t7.*t13.*t60.*t99.*1.1015625e-2;
t3134 = t7.*t13.*t50.*t130.*1.1015625e-2;
t3135 = t12.*t103.*t114.*1.865e-2;
t3140 = t19.*t21.*t117.*1.865e-2;
t3142 = t21.*t2166;
t3146 = t19.*t29.*t111.*5.5078125e-3;
t3147 = t20.*t29.*t109.*5.5078125e-3;
t3148 = t20.*t29.*t110.*5.5078125e-3;
t3156 = t21.*t2174;
t3160 = t48.*t58.*t86.*3.73e-2;
t3161 = t7.*t13.*t49.*t85.*1.1015625e-2;
t3162 = t7.*t13.*t51.*t87.*1.1015625e-2;
t3163 = t204.*t1622;
t3164 = t127.*t1963;
t3167 = t19.*t28.*t117.*1.865e-2;
t3168 = t19.*t21.*t83.*1.865e-2;
t3170 = t5.*t25.*t61.*t1009;
t3175 = t51.*t59.*t86.*3.73e-2;
t3182 = t19.*t28.*t83.*1.865e-2;
t3185 = t51.*t111.*2.98328125e-2;
t3187 = -t2961;
t3188 = t3.*t4.*t2324;
t3189 = t22.*t2214;
t3190 = t22.*t2215;
t3193 = t20.*t2218;
t3196 = t12.*t194.*2.98328125e-2;
t3197 = t58.*t111.*2.98328125e-2;
t3198 = t9.*t12.*t99.*2.98328125e-2;
t3199 = t58.*t113.*2.98328125e-2;
t3200 = t11.*t12.*t99.*2.98328125e-2;
t3203 = -t2974;
t3205 = -t2977;
t3207 = -t2979;
t3209 = t10.*t2725;
t3215 = t10.*t2727;
t3218 = t9.*t2730;
t3219 = t21.*t2223;
t3220 = t10.*t2729;
t3221 = t9.*t2731;
t3222 = t21.*t2224;
t3223 = t22.*t2223;
t3224 = t21.*t2225;
t3225 = t21.*t2226;
t3226 = t22.*t2224;
t3227 = t22.*t2225;
t3228 = t22.*t2226;
t3230 = t29.*t2215;
t3232 = t3.*t26.*t1919;
t3234 = t27.*t2218;
tau = ft_5({dq1,dq2,dq3,dq4,dq5,dq6,t10,t100,t1001,t1002,t1003,t1004,t1005,t1006,t1007,t1009,t101,t1010,t1011,t1013,t1016,t1018,t1019,t102,t1022,t1023,t1025,t1027,t1029,t1030,t1033,t1034,t1035,t1037,t1039,t104,t1041,t1042,t1043,t1047,t1048,t105,t1050,t1051,t1053,t1055,t1056,t1058,t1059,t106,t1060,t1061,t1062,t1063,t1065,t1067,t1068,t107,t1072,t1073,t1074,t1076,t1077,t1078,t108,t1080,t1081,t1082,t1083,t1084,t1085,t1086,t1087,t1088,t1089,t109,t1090,t1091,t1092,t1095,t1096,t1098,t1099,t11,t110,t1100,t1101,t1102,t1103,t1104,t1105,t1106,t1107,t1108,t111,t1110,t1111,t1112,t1113,t1114,t1116,t1117,t1119,t112,t1120,t1122,t1123,t1124,t1127,t113,t1131,t1132,t1133,t1134,t1135,t114,t1141,t1144,t1145,t1147,t1148,t1149,t1151,t1158,t1159,t116,t1160,t1161,t1162,t1163,t1164,t1165,t1166,t1167,t1169,t1170,t1171,t1172,t1173,t1176,t1177,t1178,t118,t1180,t1182,t1183,t1186,t1188,t1189,t119,t1190,t1191,t1192,t1193,t1194,t1195,t1196,t1198,t1199,t12,t120,t1201,t1202,t1203,t1204,t1205,t1207,t1208,t1210,t1211,t1212,t1214,t1215,t1216,t1217,t1218,t1219,t1220,t1221,t1222,t1224,t1227,t1228,t1229,t123,t1230,t1231,t1233,t1234,t1235,t1239,t124,t1240,t1241,t1242,t1243,t1244,t1245,t1246,t1247,t125,t1254,t1255,t1256,t126,t1263,t1266,t127,t128,t1283,t1286,t1287,t1288,t1289,t129,t1291,t1293,t1295,t1296,t1297,t1298,t1299,t13,t130,t131,t1316,t1317,t1319,t132,t1320,t1323,t1324,t1325,t1326,t1327,t1328,t1329,t133,t1331,t1332,t1333,t1334,t1335,t1345,t1346,t1347,t1349,t135,t1352,t1353,t1355,t1356,t1357,t1358,t1359,t1361,t1362,t1363,t1366,t1369,t137,t1370,t1371,t1372,t1373,t1375,t1376,t1377,t1379,t138,t1380,t1383,t1385,t1386,t1387,t1388,t139,t1390,t1391,t1392,t1393,t1395,t1397,t1398,t1399,t140,t1400,t1401,t1402,t1403,t1404,t1406,t1407,t1408,t1409,t141,t1410,t1413,t1416,t1417,t1419,t142,t1423,t1424,t1426,t1427,t1429,t143,t1432,t1433,t1434,t1435,t1438,t1441,t1442,t1443,t1445,t1447,t1450,t1452,t1453,t1456,t1457,t1458,t1462,t1463,t1464,t1465,t1466,t1467,t1468,t1469,t1470,t1473,t1475,t1476,t1477,t1479,t1480,t1481,t1482,t1483,t1484,t1487,t1488,t1489,t1490,t1491,t1493,t1494,t1495,t1496,t1497,t1498,t1499,t1500,t1502,t1503,t1504,t1505,t1511,t1513,t1523,t1524,t1525,t1526,t1528,t1530,t1531,t1532,t1533,t1534,t1536,t1537,t1538,t1539,t1540,t1541,t1544,t1545,t1546,t1554,t1555,t1556,t1557,t1558,t1562,t1563,t1564,t1566,t1567,t1568,t1571,t1575,t1576,t158,t1581,t1582,t1584,t1585,t1586,t1587,t1589,t159,t1590,t1591,t1592,t1593,t1595,t1597,t1598,t1599,t160,t1600,t1601,t1602,t1603,t1604,t1605,t1606,t1607,t1608,t1609,t161,t1610,t1611,t1612,t1613,t1614,t1618,t1619,t162,t1620,t1621,t1623,t1624,t1626,t1627,t1628,t1629,t163,t1630,t1631,t1632,t1633,t1634,t1635,t1637,t164,t1643,t165,t1654,t1655,t1656,t1657,t166,t1660,t1661,t1662,t1663,t1664,t1665,t1666,t1668,t1669,t167,t1670,t1671,t1673,t1675,t1676,t1677,t168,t1681,t1682,t1684,t1685,t1686,t1688,t1689,t1690,t1691,t1692,t1695,t1696,t1697,t1698,t170,t1700,t1701,t1702,t1703,t1704,t1705,t1706,t1709,t171,t1711,t1713,t1714,t1715,t1716,t1717,t1718,t1719,t1720,t1721,t1722,t1723,t1724,t1726,t1727,t1728,t173,t1730,t1732,t1734,t1736,t1739,t1741,t1742,t1747,t1748,t1749,t1750,t1752,t1753,t1754,t1755,t1756,t1758,t1759,t1760,t1761,t1763,t1764,t1765,t1766,t1767,t1768,t177,t1772,t1773,t1776,t1778,t1779,t178,t1780,t1781,t1782,t1785,t1786,t1787,t179,t1794,t1796,t18,t180,t1800,t1801,t1802,t1803,t1804,t1805,t1806,t1808,t181,t1815,t1816,t1817,t1818,t1819,t182,t1820,t1821,t1822,t1823,t1827,t1828,t1829,t183,t1830,t1831,t1832,t1833,t1837,t1838,t1839,t184,t1840,t1844,t1845,t1847,t1849,t185,t1850,t1851,t1852,t1853,t1854,t1857,t1858,t1859,t186,t1860,t1861,t1862,t1866,t1867,t1868,t1869,t187,t1870,t1871,t1872,t1873,t1874,t1875,t1876,t1877,t1878,t1879,t188,t1881,t1882,t1883,t1884,t1885,t1888,t1889,t189,t1890,t1893,t1895,t1896,t1897,t1898,t1899,t19,t1900,t1901,t1902,t1904,t1906,t1907,t191,t1911,t1913,t1917,t1919,t192,t1921,t1922,t1923,t1925,t1926,t1927,t193,t1931,t1936,t1937,t194,t1943,t1944,t1947,t1949,t195,t1950,t1952,t1953,t1954,t1955,t1956,t1957,t1958,t1959,t1962,t1964,t1965,t1966,t1967,t1970,t1971,t1973,t1974,t1975,t1976,t1977,t1978,t1980,t1981,t1982,t1983,t1984,t1985,t1986,t1987,t1988,t1990,t1991,t1992,t1993,t1994,t1997,t2,t20,t200,t2001,t2002,t2003,t2004,t2005,t2007,t2009,t201,t2010,t2014,t2015,t2017,t2018,t202,t2021,t2023,t2024,t2025,t2029,t203,t2030,t2031,t2034,t2035,t2036,t2037,t2038,t2039,t204,t2040,t2041,t2043,t2046,t2047,t2048,t2050,t2052,t2053,t2054,t2055,t2056,t2057,t2058,t2059,t206,t2061,t2063,t2064,t2065,t2066,t2067,t2068,t2069,t2070,t2071,t2072,t2073,t2075,t2077,t2078,t208,t2080,t2081,t2083,t2084,t2085,t2086,t2087,t2089,t209,t2090,t2091,t2092,t2093,t2094,t2096,t2097,t2098,t2099,t21,t210,t2106,t211,t2111,t2112,t2115,t2118,t212,t2121,t2124,t2125,t2126,t2128,t213,t2132,t2134,t2135,t2136,t2137,t2138,t2139,t214,t2140,t2141,t2144,t2145,t2148,t215,t2152,t2154,t2156,t2157,t2158,t2159,t216,t2160,t2161,t2162,t2163,t2165,t2167,t2169,t217,t2171,t2172,t2175,t2176,t2177,t2178,t2179,t218,t2180,t2181,t2182,t2183,t2184,t2185,t2186,t2187,t2188,t2189,t219,t2190,t2191,t2193,t2196,t2197,t2198,t2199,t22,t220,t2201,t2203,t2204,t2205,t2206,t2208,t221,t2212,t2213,t2214,t2215,t2216,t2217,t2219,t222,t2221,t2222,t2223,t2224,t2225,t2226,t2227,t2229,t223,t2231,t2232,t2233,t2235,t2236,t2237,t2238,t2239,t224,t2240,t2242,t2243,t2245,t2246,t2247,t2248,t2249,t225,t2250,t2251,t2252,t2253,t2254,t2256,t2258,t2259,t226,t2263,t2264,t2265,t2266,t2267,t2268,t2269,t227,t2277,t2278,t228,t2281,t2282,t2283,t2284,t2285,t2287,t2289,t229,t2290,t2292,t2293,t2296,t2297,t2299,t230,t2300,t2301,t231,t2310,t2312,t2313,t2314,t2319,t2322,t2323,t2324,t2326,t2327,t2329,t2330,t2331,t2332,t2333,t2334,t2338,t2339,t234,t2342,t2343,t2344,t235,t2356,t2357,t2358,t236,t2362,t2363,t2364,t2365,t2368,t2369,t237,t2370,t2371,t2372,t2374,t2376,t2378,t2379,t238,t2381,t2382,t2383,t2386,t2387,t239,t2390,t2391,t2392,t2394,t2395,t2396,t2397,t2398,t240,t2400,t2401,t2402,t2403,t2405,t2408,t2409,t241,t2410,t2412,t2413,t2414,t2416,t2417,t2418,t2419,t242,t2421,t2422,t2423,t2424,t2425,t2426,t2427,t2428,t2429,t243,t2430,t2431,t2432,t2433,t2436,t2437,t2438,t2439,t244,t2440,t2449,t245,t2450,t2451,t2452,t2453,t2454,t2455,t2456,t2457,t2459,t246,t2464,t2465,t2466,t2467,t2468,t2469,t247,t2470,t2471,t2472,t2473,t2474,t2475,t2476,t2477,t2478,t2479,t248,t2481,t2482,t2483,t2484,t2485,t2486,t2487,t2488,t249,t2491,t2492,t2494,t2495,t2496,t2498,t25,t250,t2504,t2508,t251,t2511,t2512,t2513,t2514,t2515,t2516,t2517,t2518,t252,t2520,t2523,t2524,t2525,t2527,t2529,t253,t2531,t2534,t2536,t2537,t2538,t2541,t2542,t2546,t2547,t2548,t255,t2550,t2552,t2553,t2554,t2555,t2556,t2557,t2559,t256,t2560,t2563,t2564,t2565,t2566,t2567,t2568,t2569,t2570,t2571,t2572,t2573,t2574,t2575,t2576,t2577,t2578,t2579,t2580,t2581,t2582,t2583,t2585,t2586,t2587,t2588,t259,t2591,t2593,t2594,t2595,t2596,t2597,t2598,t2599,t26,t260,t2600,t2601,t2602,t2603,t2604,t2605,t2607,t2608,t2609,t261,t2610,t2611,t2614,t2615,t2616,t2617,t262,t2622,t2623,t2625,t2628,t2629,t263,t2631,t2632,t2634,t2636,t2638,t2644,t2646,t2649,t265,t2650,t2652,t2659,t2660,t2661,t2665,t2666,t2667,t2668,t2669,t267,t2670,t2671,t2672,t2673,t2674,t2675,t2679,t2681,t2682,t2683,t2685,t2686,t2689,t269,t2692,t2694,t2696,t2697,t2698,t27,t270,t2700,t2701,t2702,t2703,t2705,t2706,t2707,t2711,t272,t2723,t2724,t2725,t2726,t2727,t2729,t273,t2730,t2731,t2732,t2733,t2734,t2735,t2736,t2738,t2739,t274,t2740,t2741,t2742,t2744,t2745,t2746,t2747,t2748,t2749,t275,t2751,t2752,t2753,t2754,t2755,t2756,t2757,t2758,t2759,t276,t2762,t2763,t2764,t2765,t2766,t2767,t2769,t277,t2770,t2771,t2776,t2778,t2779,t278,t2780,t2782,t2784,t2785,t2786,t2788,t279,t2792,t2793,t2795,t28,t280,t2800,t2802,t2803,t2804,t2806,t2807,t2809,t281,t2810,t2812,t2813,t2814,t2815,t2819,t2820,t2821,t2822,t2825,t2827,t2828,t2829,t283,t2830,t2832,t2833,t2834,t2836,t2839,t284,t2842,t2843,t2844,t285,t2850,t2854,t2858,t286,t2860,t2862,t2864,t2865,t2866,t2867,t2869,t287,t2870,t2871,t2872,t2873,t2877,t288,t2880,t2882,t2883,t2885,t2887,t2888,t289,t2890,t2891,t2892,t2899,t29,t290,t2900,t2901,t2902,t2903,t2904,t2905,t2906,t2911,t2912,t2913,t2916,t2919,t292,t2921,t2922,t2923,t2924,t2925,t2926,t2927,t2928,t2929,t293,t2930,t2931,t2932,t2933,t2934,t2935,t2937,t2938,t2939,t294,t2940,t2942,t2943,t2944,t2945,t2946,t2947,t2948,t2949,t295,t2950,t2951,t2952,t2953,t2954,t2956,t2957,t2959,t296,t2960,t2962,t2964,t2965,t2966,t2967,t2968,t297,t2970,t2973,t2974,t2975,t2977,t2978,t2979,t298,t2981,t2983,t2984,t2986,t2988,t299,t2991,t2995,t2997,t2998,t3,t300,t3002,t3003,t3004,t3006,t3007,t301,t3010,t3011,t3012,t3013,t3015,t3016,t3017,t302,t3020,t3021,t3023,t3025,t3028,t303,t3034,t3035,t3036,t3037,t304,t3040,t3042,t3046,t3047,t3049,t305,t3051,t3052,t3053,t3054,t3056,t3057,t3058,t3059,t306,t3060,t3061,t3062,t3064,t3065,t3066,t3067,t3068,t3069,t307,t3070,t3071,t3072,t3073,t3074,t3075,t3076,t3077,t3078,t3079,t308,t3080,t3081,t3082,t3083,t3085,t3087,t3088,t309,t3091,t3092,t3093,t3094,t3095,t3096,t3097,t3099,t3100,t3101,t3102,t3103,t3104,t3107,t3108,t3109,t311,t3110,t3111,t3112,t3118,t312,t3126,t3128,t313,t3131,t3132,t3133,t3134,t3135,t3138,t3139,t314,t3140,t3142,t3143,t3146,t3147,t3148,t315,t3156,t316,t3160,t3161,t3162,t3163,t3164,t3167,t3168,t317,t3170,t3175,t318,t3182,t3185,t3187,t3188,t3189,t319,t3190,t3192,t3193,t3196,t3197,t3198,t3199,t320,t3200,t3203,t3204,t3205,t3206,t3207,t3208,t3209,t321,t3210,t3211,t3212,t3213,t3214,t3215,t3216,t3217,t3218,t3219,t322,t3220,t3221,t3222,t3223,t3224,t3225,t3226,t3227,t3228,t323,t3230,t3231,t3232,t3234,t324,t3245,t3246,t325,t326,t3262,t327,t3272,t328,t329,t3298,t3299,t330,t331,t332,t3320,t3326,t333,t3330,t334,t336,t337,t338,t3388,t339,t3396,t341,t342,t343,t344,t345,t3453,t346,t347,t3470,t3471,t3473,t3479,t348,t3480,t3483,t3484,t3485,t3486,t349,t3490,t3491,t3497,t3498,t350,t3501,t3510,t3511,t352,t3521,t3526,t3527,t3528,t3529,t353,t354,t3546,t3547,t3549,t355,t3551,t3559,t356,t3560,t3562,t357,t358,t3589,t3590,t3592,t3593,t3594,t3595,t360,t3608,t3609,t3611,t3612,t3613,t3614,t3615,t3616,t3617,t3627,t3628,t3629,t3630,t3635,t3636,t3637,t364,t3648,t365,t3650,t3651,t367,t368,t3680,t3687,t3690,t3691,t3692,t3704,t3705,t371,t3722,t3723,t3724,t3725,t3726,t373,t375,t376,t377,t3779,t378,t379,t3796,t380,t381,t3811,t382,t3822,t3823,t3824,t3827,t3828,t383,t3839,t384,t385,t386,t3862,t3865,t3868,t387,t3871,t3872,t388,t3884,t389,t3909,t391,t3910,t392,t3932,t3935,t3941,t396,t3960,t3963,t397,t399,t4,t400,t401,t402,t4031,t404,t4042,t4043,t4046,t4047,t405,t4057,t406,t4060,t4061,t4067,t407,t4075,t408,t409,t410,t4103,t4109,t411,t412,t413,t414,t415,t416,t4168,t417,t4174,t418,t419,t420,t4204,t4208,t4209,t421,t4212,t422,t423,t424,t425,t426,t4260,t4261,t4262,t4263,t4265,t427,t4280,t429,t430,t431,t432,t433,t434,t4344,t4345,t4347,t435,t436,t437,t4372,t438,t439,t440,t441,t442,t443,t444,t4451,t4452,t4456,t4457,t4475,t4477,t4478,t450,t4508,t451,t453,t4539,t454,t4542,t4544,t4545,t4546,t4547,t456,t4565,t4566,t4568,t4579,t458,t4581,t4584,t459,t460,t461,t462,t463,t464,t465,t467,t468,t469,t470,t471,t472,t473,t474,t475,t476,t4763,t4765,t4766,t4768,t4769,t477,t4770,t4771,t4773,t478,t479,t48,t480,t4806,t4808,t481,t482,t483,t4830,t4831,t4833,t484,t486,t487,t488,t489,t4895,t4898,t49,t490,t4900,t491,t492,t494,t495,t496,t497,t498,t499,t5,t50,t500,t501,t502,t5041,t5054,t5055,t509,t51,t510,t5103,t511,t512,t513,t514,t515,t516,t517,t5175,t5176,t518,t519,t52,t520,t521,t522,t523,t524,t527,t528,t5280,t529,t53,t530,t531,t534,t5343,t5344,t535,t5354,t5356,t536,t5361,t539,t54,t540,t5411,t542,t543,t545,t546,t547,t548,t5491,t5492,t55,t550,t551,t552,t553,t5551,t5552,t556,t557,t558,t559,t56,t560,t561,t5613,t562,t563,t565,t566,t567,t569,t57,t574,t58,t582,t585,t589,t59,t590,t592,t594,t595,t597,t598,t599,t6,t60,t600,t601,t602,t6023,t604,t605,t606,t608,t609,t61,t610,t611,t613,t614,t616,t617,t62,t624,t63,t630,t632,t635,t636,t641,t643,t644,t645,t647,t6473,t648,t649,t650,t651,t652,t653,t654,t655,t656,t657,t658,t66,t660,t661,t663,t664,t666,t667,t669,t67,t670,t6734,t6735,t6736,t674,t6742,t6743,t6744,t6745,t675,t6754,t6755,t676,t677,t6772,t678,t679,t680,t681,t683,t684,t685,t686,t687,t688,t689,t690,t691,t692,t693,t696,t699,t7,t700,t702,t703,t704,t705,t706,t708,t711,t713,t715,t716,t717,t719,t720,t721,t722,t723,t725,t726,t729,t731,t732,t734,t737,t738,t742,t744,t748,t750,t751,t754,t756,t758,t759,t761,t763,t766,t767,t768,t769,t770,t773,t774,t775,t776,t781,t782,t784,t785,t788,t789,t790,t793,t795,t796,t798,t799,t8,t800,t803,t805,t807,t808,t809,t81,t814,t815,t816,t817,t819,t82,t820,t821,t822,t823,t824,t826,t828,t829,t83,t831,t832,t833,t834,t835,t837,t838,t839,t84,t842,t844,t847,t848,t849,t85,t850,t851,t852,t853,t854,t858,t859,t86,t861,t863,t864,t867,t868,t87,t871,t872,t875,t879,t88,t880,t883,t884,t885,t886,t888,t89,t890,t891,t894,t895,t896,t897,t898,t899,t9,t90,t900,t902,t905,t906,t907,t908,t909,t910,t911,t912,t913,t914,t915,t916,t918,t919,t92,t920,t921,t923,t926,t928,t929,t93,t930,t931,t933,t934,t935,t936,t937,t938,t944,t945,t946,t947,t948,t949,t95,t950,t951,t954,t955,t956,t957,t958,t959,t96,t960,t961,t962,t963,t964,t965,t966,t967,t968,t969,t97,t970,t972,t973,t974,t975,t976,t977,t978,t98,t981,t982,t984,t986,t987,t988,t99,t990,t991,t992,t993,t994,t996,t997,t999});
end
function tau = ft_5(ct)
